simulink model "KUKA_LBR_Simulink_model_flatness_based_control"  (R2017a)
(part 9 of 19)

dblMassInertFullRow6Col4 = (cos(q3)*sin(q1) + cos(q1)*cos(q2)*sin(q3))*(KUKA_LBR_param_.dblLink7InertXZ*(cos(q5)*sin(q2)*sin(q3) + (cos(q3)*cos(q4)*sin(q2) - cos(q2)*sin(q4))*sin(q5)) + KUKA_LBR_param_.dblLink7InertXX*(-(cos(q5)*(cos(q3)*sin(q1) + cos(q1)*cos(q2)*sin(q3))) + (cos(q4)*sin(q1)*sin(q3) - cos(q1)*(cos(q2)*cos(q3)*cos(q4) + sin(q2)*sin(q4)))*sin(q5)) + KUKA_LBR_param_.dblLink7InertXY*(cos(q1)*(cos(q3)*cos(q5) - cos(q4)*sin(q3)*sin(q5)) - sin(q1)*(sin(q2)*sin(q4)*sin(q5) + cos(q2)*(cos(q5)*sin(q3) + cos(q3)*cos(q4)*sin(q5))))) + (-(cos(q1)*cos(q3)) + cos(q2)*sin(q1)*sin(q3))*(KUKA_LBR_param_.dblLink7InertYZ*(cos(q5)*sin(q2)*sin(q3) + (cos(q3)*cos(q4)*sin(q2) - cos(q2)*sin(q4))*sin(q5)) + KUKA_LBR_param_.dblLink7InertXY*(-(cos(q5)*(cos(q3)*sin(q1) + cos(q1)*cos(q2)*sin(q3))) + (cos(q4)*sin(q1)*sin(q3) - cos(q1)*(cos(q2)*cos(q3)*cos(q4) + sin(q2)*sin(q4)))*sin(q5)) + KUKA_LBR_param_.dblLink7InertYY*(cos(q1)*(cos(q3)*cos(q5) - cos(q4)*sin(q3)*sin(q5)) - sin(q1)*(sin(q2)*sin(q4)*sin(q5) + cos(q2)*(cos(q5)*sin(q3) + cos(q3)*cos(q4)*sin(q5))))) - sin(q2)*sin(q3)*(KUKA_LBR_param_.dblLink7InertZZ*(cos(q5)*sin(q2)*sin(q3) + (cos(q3)*cos(q4)*sin(q2) - cos(q2)*sin(q4))*sin(q5)) + KUKA_LBR_param_.dblLink7InertXZ*(-(cos(q5)*(cos(q3)*sin(q1) + cos(q1)*cos(q2)*sin(q3))) + (cos(q4)*sin(q1)*sin(q3) - cos(q1)*(cos(q2)*cos(q3)*cos(q4) + sin(q2)*sin(q4)))*sin(q5)) + KUKA_LBR_param_.dblLink7InertYZ*(cos(q1)*(cos(q3)*cos(q5) - cos(q4)*sin(q3)*sin(q5)) - sin(q1)*(sin(q2)*sin(q4)*sin(q5) + cos(q2)*(cos(q5)*sin(q3) + cos(q3)*cos(q4)*sin(q5))))) + (cos(q5)*(-12*KUKA_LBR_param_.dblLink6InertXX - 12*KUKA_LBR_param_.dblLink6InertYY - 8*KUKA_LBR_param_.dblLink6InertZZ - 32*power(KUKA_LBR_param_.dblLink6CogX,2)*KUKA_LBR_param_.dblLink6Mass - 32*power(KUKA_LBR_param_.dblLink6CogY,2)*KUKA_LBR_param_.dblLink6Mass + 4*(KUKA_LBR_param_.dblLink6InertXX - KUKA_LBR_param_.dblLink6InertYY)*cos(2*q1) + 8*KUKA_LBR_param_.dblLink6InertYZ*cos(q1 - 2*q2) - 2*KUKA_LBR_param_.dblLink6InertXX*cos(2*(q1 - q2)) + 2*KUKA_LBR_param_.dblLink6InertYY*cos(2*(q1 - q2)) - 4*KUKA_LBR_param_.dblLink6InertXX*cos(2*q2) - 4*KUKA_LBR_param_.dblLink6InertYY*cos(2*q2) + 8*KUKA_LBR_param_.dblLink6InertZZ*cos(2*q2) - 2*KUKA_LBR_param_.dblLink6InertXX*cos(2*(q1 + q2)) + 2*KUKA_LBR_param_.dblLink6InertYY*cos(2*(q1 + q2)) - 8*KUKA_LBR_param_.dblLink6InertYZ*cos(q1 + 2*q2) + 8*KUKA_LBR_param_.dblLink6InertYZ*cos(q1 - q2 - 2*q3) - 4*KUKA_LBR_param_.dblLink6InertXX*cos(2*q1 - q2 - 2*q3) + 4*KUKA_LBR_param_.dblLink6InertYY*cos(2*q1 - q2 - 2*q3) - 8*KUKA_LBR_param_.dblLink6InertYZ*cos(q1 + q2 - 2*q3) - 4*KUKA_LBR_param_.dblLink6InertXX*cos(2*q1 + q2 - 2*q3) + 4*KUKA_LBR_param_.dblLink6InertYY*cos(2*q1 + q2 - 2*q3) + 4*KUKA_LBR_param_.dblLink6InertYZ*cos(q1 + 2*q2 - 2*q3) + 6*KUKA_LBR_param_.dblLink6InertXX*cos(2*(q1 - q3)) - 6*KUKA_LBR_param_.dblLink6InertYY*cos(2*(q1 - q3)) + KUKA_LBR_param_.dblLink6InertXX*cos(2*(q1 - q2 - q3)) - KUKA_LBR_param_.dblLink6InertYY*cos(2*(q1 - q2 - q3)) + 2*KUKA_LBR_param_.dblLink6InertXX*cos(2*(q2 - q3)) + 2*KUKA_LBR_param_.dblLink6InertYY*cos(2*(q2 - q3)) - 4*KUKA_LBR_param_.dblLink6InertZZ*cos(2*(q2 - q3)) + KUKA_LBR_param_.dblLink6InertXX*cos(2*(q1 + q2 - q3)) - KUKA_LBR_param_.dblLink6InertYY*cos(2*(q1 + q2 - q3)) - 4*KUKA_LBR_param_.dblLink6InertXX*cos(2*q3) - 4*KUKA_LBR_param_.dblLink6InertYY*cos(2*q3) + 8*KUKA_LBR_param_.dblLink6InertZZ*cos(2*q3) + 6*KUKA_LBR_param_.dblLink6InertXX*cos(2*(q1 + q3)) - 6*KUKA_LBR_param_.dblLink6InertYY*cos(2*(q1 + q3)) + KUKA_LBR_param_.dblLink6InertXX*cos(2*(q1 - q2 + q3)) - KUKA_LBR_param_.dblLink6InertYY*cos(2*(q1 - q2 + q3)) + 2*KUKA_LBR_param_.dblLink6InertXX*cos(2*(q2 + q3)) + 2*KUKA_LBR_param_.dblLink6InertYY*cos(2*(q2 + q3)) - 4*KUKA_LBR_param_.dblLink6InertZZ*cos(2*(q2 + q3)) + KUKA_LBR_param_.dblLink6InertXX*cos(2*(q1 + q2 + q3)) - KUKA_LBR_param_.dblLink6InertYY*cos(2*(q1 + q2 + q3)) - 4*KUKA_LBR_param_.dblLink6InertYZ*cos(q1 - 2*q2 + 2*q3) - 8*KUKA_LBR_param_.dblLink6InertYZ*cos(q1 - q2 + 2*q3) + 4*KUKA_LBR_param_.dblLink6InertXX*cos(2*q1 - q2 + 2*q3) - 4*KUKA_LBR_param_.dblLink6InertYY*cos(2*q1 - q2 + 2*q3) + 8*KUKA_LBR_param_.dblLink6InertYZ*cos(q1 + q2 + 2*q3) + 4*KUKA_LBR_param_.dblLink6InertXX*cos(2*q1 + q2 + 2*q3) - 4*KUKA_LBR_param_.dblLink6InertYY*cos(2*q1 + q2 + 2*q3) - 4*KUKA_LBR_param_.dblLink6InertYZ*cos(q1 - 2*(q2 + q3)) + 4*KUKA_LBR_param_.dblLink6InertYZ*cos(q1 + 2*(q2 + q3)) - 32*KUKA_LBR_param_.dblLink45Len*KUKA_LBR_param_.dblLink6CogY*KUKA_LBR_param_.dblLink6Mass*cos(q6) + 8*KUKA_LBR_param_.dblLink6InertXY*sin(2*q1) - 8*KUKA_LBR_param_.dblLink6InertXZ*sin(q1 - 2*q2) - 4*KUKA_LBR_param_.dblLink6InertXY*sin(2*(q1 - q2)) - 4*KUKA_LBR_param_.dblLink6InertXY*sin(2*(q1 + q2)) + 8*KUKA_LBR_param_.dblLink6InertXZ*sin(q1 + 2*q2) - 8*KUKA_LBR_param_.dblLink6InertXZ*sin(q1 - q2 - 2*q3) - 8*KUKA_LBR_param_.dblLink6InertXY*sin(2*q1 - q2 - 2*q3) + 8*KUKA_LBR_param_.dblLink6InertXZ*sin(q1 + q2 - 2*q3) - 8*KUKA_LBR_param_.dblLink6InertXY*sin(2*q1 + q2 - 2*q3) - 4*KUKA_LBR_param_.dblLink6InertXZ*sin(q1 + 2*q2 - 2*q3) + 12*KUKA_LBR_param_.dblLink6InertXY*sin(2*(q1 - q3)) + 2*KUKA_LBR_param_.dblLink6InertXY*sin(2*(q1 - q2 - q3)) + 2*KUKA_LBR_param_.dblLink6InertXY*sin(2*(q1 + q2 - q3)) + 12*KUKA_LBR_param_.dblLink6InertXY*sin(2*(q1 + q3)) + 2*KUKA_LBR_param_.dblLink6InertXY*sin(2*(q1 - q2 + q3)) + 2*KUKA_LBR_param_.dblLink6InertXY*sin(2*(q1 + q2 + q3)) + 4*KUKA_LBR_param_.dblLink6InertXZ*sin(q1 - 2*q2 + 2*q3) + 8*KUKA_LBR_param_.dblLink6InertXZ*sin(q1 - q2 + 2*q3) + 8*KUKA_LBR_param_.dblLink6InertXY*sin(2*q1 - q2 + 2*q3) - 8*KUKA_LBR_param_.dblLink6InertXZ*sin(q1 + q2 + 2*q3) + 8*KUKA_LBR_param_.dblLink6InertXY*sin(2*q1 + q2 + 2*q3) + 4*KUKA_LBR_param_.dblLink6InertXZ*sin(q1 - 2*(q2 + q3)) - 4*KUKA_LBR_param_.dblLink6InertXZ*sin(q1 + 2*(q2 + q3)) - 32*KUKA_LBR_param_.dblLink45Len*KUKA_LBR_param_.dblLink6CogX*KUKA_LBR_param_.dblLink6Mass*sin(q6)) + 4*sin(q5)*(-8*KUKA_LBR_param_.dblLink6CogX*KUKA_LBR_param_.dblLink6CogZ*KUKA_LBR_param_.dblLink6Mass*cos(q6) + 8*KUKA_LBR_param_.dblLink6InertXZ*power(cos(q3),2)*cos(q4)*sin(q1)*sin(q2) - 8*KUKA_LBR_param_.dblLink6InertXZ*cos(q4)*sin(q1)*sin(q2)*power(sin(q3),2) + KUKA_LBR_param_.dblLink6InertXX*cos(q4)*sin(2*q3) + KUKA_LBR_param_.dblLink6InertYY*cos(q4)*sin(2*q3) - 2*KUKA_LBR_param_.dblLink6InertZZ*cos(q4)*sin(2*q3) + 3*KUKA_LBR_param_.dblLink6InertXX*cos(q4)*power(sin(q1),2)*sin(2*q3) - 3*KUKA_LBR_param_.dblLink6InertYY*cos(q4)*power(sin(q1),2)*sin(2*q3) - 6*KUKA_LBR_param_.dblLink6InertXY*cos(q4)*sin(2*q1)*sin(2*q3) + KUKA_LBR_param_.dblLink6InertXX*cos(q4)*power(sin(q2),2)*sin(2*q3) + KUKA_LBR_param_.dblLink6InertYY*cos(q4)*power(sin(q2),2)*sin(2*q3) - 2*KUKA_LBR_param_.dblLink6InertZZ*cos(q4)*power(sin(q2),2)*sin(2*q3) - KUKA_LBR_param_.dblLink6InertXX*cos(q4)*power(sin(q1),2)*power(sin(q2),2)*sin(2*q3) + KUKA_LBR_param_.dblLink6InertYY*cos(q4)*power(sin(q1),2)*power(sin(q2),2)*sin(2*q3) + 2*KUKA_LBR_param_.dblLink6InertXY*cos(q4)*sin(2*q1)*power(sin(q2),2)*sin(2*q3) + 4*KUKA_LBR_param_.dblLink6InertYZ*cos(q4)*sin(q1)*sin(2*q2)*sin(2*q3) - 8*KUKA_LBR_param_.dblLink6InertXY*cos(q3)*power(sin(q1),2)*sin(q2)*sin(q4) - 4*KUKA_LBR_param_.dblLink6InertXX*cos(q3)*sin(2*q1)*sin(q2)*sin(q4) + 4*KUKA_LBR_param_.dblLink6InertYY*cos(q3)*sin(2*q1)*sin(q2)*sin(q4) - 4*KUKA_LBR_param_.dblLink6InertXX*cos(q2)*sin(q2)*sin(q3)*sin(q4) + 4*KUKA_LBR_param_.dblLink6InertXX*cos(q2)*power(sin(q1),2)*sin(q2)*sin(q3)*sin(q4) + 8*KUKA_LBR_param_.dblLink6InertYZ*sin(q1)*power(sin(q2),2)*sin(q3)*sin(q4) - 2*KUKA_LBR_param_.dblLink6InertYY*sin(2*q2)*sin(q3)*sin(q4) + 4*KUKA_LBR_param_.dblLink6InertZZ*sin(2*q2)*sin(q3)*sin(q4) - 2*KUKA_LBR_param_.dblLink6InertYY*power(sin(q1),2)*sin(2*q2)*sin(q3)*sin(q4) - 4*KUKA_LBR_param_.dblLink6InertXY*sin(2*q1)*sin(2*q2)*sin(q3)*sin(q4) - 4*cos(q2)*(2*KUKA_LBR_param_.dblLink6InertXY*power(cos(q3),2)*cos(q4)*power(sin(q1),2) + cos(q4)*((KUKA_LBR_param_.dblLink6InertXX - KUKA_LBR_param_.dblLink6InertYY)*cos(2*q3)*sin(2*q1) - 2*KUKA_LBR_param_.dblLink6InertXY*power(sin(q1),2)*power(sin(q3),2)) + 2*KUKA_LBR_param_.dblLink6InertXZ*cos(q3)*sin(q1)*sin(q4)) - (power(cos(q2),2)*(cos(q4)*(KUKA_LBR_param_.dblLink6InertXX + 3*KUKA_LBR_param_.dblLink6InertYY - 4*KUKA_LBR_param_.dblLink6InertZZ + (KUKA_LBR_param_.dblLink6InertXX - KUKA_LBR_param_.dblLink6InertYY)*cos(2*q1) + 4*KUKA_LBR_param_.dblLink6InertXY*sin(2*q1))*sin(2*q3) + 16*KUKA_LBR_param_.dblLink6InertYZ*sin(q1)*sin(q3)*sin(q4)))/2.0 - 8*cos(q1)*(KUKA_LBR_param_.dblLink6InertYZ*power(cos(q3),2)*cos(q4)*sin(q2) - cos(q2)*cos(q3)*(2*KUKA_LBR_param_.dblLink6InertXZ*cos(q4)*sin(q2)*sin(q3) + KUKA_LBR_param_.dblLink6InertYZ*sin(q4)) + sin(q3)*(-(KUKA_LBR_param_.dblLink6InertYZ*cos(q4)*sin(q2)*sin(q3)) + KUKA_LBR_param_.dblLink6InertXZ*cos(2*q2)*sin(q4))) + 2*power(cos(q1),2)*(-((KUKA_LBR_param_.dblLink6InertXX - KUKA_LBR_param_.dblLink6InertYY)*power(cos(q2),2)*cos(q3)*cos(q4)*sin(q3)) + KUKA_LBR_param_.dblLink6InertYY*sin(2*q2)*sin(q3)*sin(q4) + cos(q3)*(-((KUKA_LBR_param_.dblLink6InertXX - KUKA_LBR_param_.dblLink6InertYY)*(5 + cos(2*q2))*cos(q4)*sin(q3))/2.0 + 4*KUKA_LBR_param_.dblLink6InertXY*sin(q2)*sin(q4)) + cos(q2)*(4*KUKA_LBR_param_.dblLink6InertXY*power(cos(q3),2)*cos(q4) - 2*sin(q3)*(2*KUKA_LBR_param_.dblLink6InertXY*cos(q4)*sin(q3) + KUKA_LBR_param_.dblLink6InertXX*sin(q2)*sin(q4)))) + 8*KUKA_LBR_param_.dblLink6CogY*KUKA_LBR_param_.dblLink6CogZ*KUKA_LBR_param_.dblLink6Mass*sin(q6)))/32.0 - KUKA_LBR_param_.dblLink7Mass*(cos(q4)*(-(sin(q1)*sin(q2)*sin(q5)*(KUKA_LBR_param_.dblLink7CogY*cos(q7) + KUKA_LBR_param_.dblLink7CogX*sin(q7))) + cos(q1)*sin(q3)*(KUKA_LBR_param_.dblLink45Len + KUKA_LBR_param_.dblLink7CogZ*cos(q6) + KUKA_LBR_param_.dblLink7CogX*cos(q7)*sin(q6) - KUKA_LBR_param_.dblLink7CogY*sin(q6)*sin(q7)) - cos(q5)*sin(q1)*sin(q2)*(KUKA_LBR_param_.dblLink7CogZ*sin(q6) + cos(q6)*(-(KUKA_LBR_param_.dblLink7CogX*cos(q7)) + KUKA_LBR_param_.dblLink7CogY*sin(q7)))) + sin(q4)*(sin(q1)*sin(q2)*(KUKA_LBR_param_.dblLink45Len + KUKA_LBR_param_.dblLink7CogZ*cos(q6) + KUKA_LBR_param_.dblLink7CogX*cos(q7)*sin(q6) - KUKA_LBR_param_.dblLink7CogY*sin(q6)*sin(q7)) + cos(q1)*sin(q3)*(sin(q5)*(KUKA_LBR_param_.dblLink7CogY*cos(q7) + KUKA_LBR_param_.dblLink7CogX*sin(q7)) + cos(q5)*(-(KUKA_LBR_param_.dblLink7CogX*cos(q6)*cos(q7)) + KUKA_LBR_param_.dblLink7CogZ*sin(q6) + KUKA_LBR_param_.dblLink7CogY*cos(q6)*sin(q7)))) + cos(q2)*cos(q3)*sin(q1)*(cos(q4)*(KUKA_LBR_param_.dblLink45Len + KUKA_LBR_param_.dblLink7CogZ*cos(q6) + KUKA_LBR_param_.dblLink7CogX*cos(q7)*sin(q6) - KUKA_LBR_param_.dblLink7CogY*sin(q6)*sin(q7)) + sin(q4)*(sin(q5)*(KUKA_LBR_param_.dblLink7CogY*cos(q7) + KUKA_LBR_param_.dblLink7CogX*sin(q7)) + cos(q5)*(-(KUKA_LBR_param_.dblLink7CogX*cos(q6)*cos(q7)) + KUKA_LBR_param_.dblLink7CogZ*sin(q6) + KUKA_LBR_param_.dblLink7CogY*cos(q6)*sin(q7)))))*(KUKA_LBR_param_.dblLink7CogZ*cos(q5)*cos(q6)*sin(q1)*sin(q2)*sin(q4) - KUKA_LBR_param_.dblLink7CogX*cos(q1)*cos(q6)*cos(q7)*sin(q3)*sin(q4) + KUKA_LBR_param_.dblLink7CogZ*cos(q1)*cos(q3)*cos(q6)*sin(q5) + KUKA_LBR_param_.dblLink7CogX*cos(q5)*cos(q7)*sin(q1)*sin(q2)*sin(q4)*sin(q6) + KUKA_LBR_param_.dblLink7CogZ*cos(q1)*sin(q3)*sin(q4)*sin(q6) + KUKA_LBR_param_.dblLink7CogX*cos(q1)*cos(q3)*cos(q7)*sin(q5)*sin(q6) + KUKA_LBR_param_.dblLink7CogY*cos(q1)*cos(q6)*sin(q3)*sin(q4)*sin(q7) - KUKA_LBR_param_.dblLink7CogY*cos(q5)*sin(q1)*sin(q2)*sin(q4)*sin(q6)*sin(q7) - KUKA_LBR_param_.dblLink7CogY*cos(q1)*cos(q3)*sin(q5)*sin(q6)*sin(q7) + cos(q4)*(cos(q6)*(KUKA_LBR_param_.dblLink7CogX*cos(q7)*sin(q1)*sin(q2) + KUKA_LBR_param_.dblLink7CogZ*cos(q1)*cos(q5)*sin(q3) - KUKA_LBR_param_.dblLink7CogY*sin(q1)*sin(q2)*sin(q7)) - sin(q6)*(KUKA_LBR_param_.dblLink7CogZ*sin(q1)*sin(q2) + cos(q1)*cos(q5)*sin(q3)*(-(KUKA_LBR_param_.dblLink7CogX*cos(q7)) + KUKA_LBR_param_.dblLink7CogY*sin(q7)))) + cos(q2)*sin(q1)*(-(sin(q3)*sin(q5)*(KUKA_LBR_param_.dblLink7CogZ*cos(q6) + sin(q6)*(KUKA_LBR_param_.dblLink7CogX*cos(q7) - KUKA_LBR_param_.dblLink7CogY*sin(q7)))) + cos(q3)*(sin(q4)*(-(KUKA_LBR_param_.dblLink7CogX*cos(q6)*cos(q7)) + KUKA_LBR_param_.dblLink7CogZ*sin(q6) + KUKA_LBR_param_.dblLink7CogY*cos(q6)*sin(q7)) + cos(q4)*cos(q5)*(KUKA_LBR_param_.dblLink7CogZ*cos(q6) + KUKA_LBR_param_.dblLink7CogX*cos(q7)*sin(q6) - KUKA_LBR_param_.dblLink7CogY*sin(q6)*sin(q7))))) + KUKA_LBR_param_.dblLink7Mass*(cos(q2)*(-(sin(q4)*(KUKA_LBR_param_.dblLink45Len + KUKA_LBR_param_.dblLink7CogZ*cos(q6) + KUKA_LBR_param_.dblLink7CogX*cos(q7)*sin(q6) - KUKA_LBR_param_.dblLink7CogY*sin(q6)*sin(q7))) + cos(q4)*(sin(q5)*(KUKA_LBR_param_.dblLink7CogY*cos(q7) + KUKA_LBR_param_.dblLink7CogX*sin(q7)) + cos(q5)*(-(KUKA_LBR_param_.dblLink7CogX*cos(q6)*cos(q7)) + KUKA_LBR_param_.dblLink7CogZ*sin(q6) + KUKA_LBR_param_.dblLink7CogY*cos(q6)*sin(q7)))) + cos(q3)*sin(q2)*(cos(q4)*(KUKA_LBR_param_.dblLink45Len + KUKA_LBR_param_.dblLink7CogZ*cos(q6) + KUKA_LBR_param_.dblLink7CogX*cos(q7)*sin(q6) - KUKA_LBR_param_.dblLink7CogY*sin(q6)*sin(q7)) + sin(q4)*(sin(q5)*(KUKA_LBR_param_.dblLink7CogY*cos(q7) + KUKA_LBR_param_.dblLink7CogX*sin(q7)) + cos(q5)*(-(KUKA_LBR_param_.dblLink7CogX*cos(q6)*cos(q7)) + KUKA_LBR_param_.dblLink7CogZ*sin(q6) + KUKA_LBR_param_.dblLink7CogY*cos(q6)*sin(q7)))))*(cos(q2)*(cos(q4)*(KUKA_LBR_param_.dblLink7CogX*cos(q6)*cos(q7) - KUKA_LBR_param_.dblLink7CogZ*sin(q6) - KUKA_LBR_param_.dblLink7CogY*cos(q6)*sin(q7)) + cos(q5)*sin(q4)*(KUKA_LBR_param_.dblLink7CogZ*cos(q6) + KUKA_LBR_param_.dblLink7CogX*cos(q7)*sin(q6) - KUKA_LBR_param_.dblLink7CogY*sin(q6)*sin(q7))) - sin(q2)*(-(sin(q3)*sin(q5)*(KUKA_LBR_param_.dblLink7CogZ*cos(q6) + sin(q6)*(KUKA_LBR_param_.dblLink7CogX*cos(q7) - KUKA_LBR_param_.dblLink7CogY*sin(q7)))) + cos(q3)*(sin(q4)*(-(KUKA_LBR_param_.dblLink7CogX*cos(q6)*cos(q7)) + KUKA_LBR_param_.dblLink7CogZ*sin(q6) + KUKA_LBR_param_.dblLink7CogY*cos(q6)*sin(q7)) + cos(q4)*cos(q5)*(KUKA_LBR_param_.dblLink7CogZ*cos(q6) + KUKA_LBR_param_.dblLink7CogX*cos(q7)*sin(q6) - KUKA_LBR_param_.dblLink7CogY*sin(q6)*sin(q7))))) + KUKA_LBR_param_.dblLink7Mass*(sin(q1)*sin(q3)*(cos(q4)*(KUKA_LBR_param_.dblLink45Len + KUKA_LBR_param_.dblLink7CogZ*cos(q6) + KUKA_LBR_param_.dblLink7CogX*cos(q7)*sin(q6) - KUKA_LBR_param_.dblLink7CogY*sin(q6)*sin(q7)) + sin(q4)*(sin(q5)*(KUKA_LBR_param_.dblLink7CogY*cos(q7) + KUKA_LBR_param_.dblLink7CogX*sin(q7)) + cos(q5)*(-(KUKA_LBR_param_.dblLink7CogX*cos(q6)*cos(q7)) + KUKA_LBR_param_.dblLink7CogZ*sin(q6) + KUKA_LBR_param_.dblLink7CogY*cos(q6)*sin(q7)))) - cos(q1)*(sin(q2)*(sin(q4)*(KUKA_LBR_param_.dblLink45Len + KUKA_LBR_param_.dblLink7CogZ*cos(q6) + KUKA_LBR_param_.dblLink7CogX*cos(q7)*sin(q6) - KUKA_LBR_param_.dblLink7CogY*sin(q6)*sin(q7)) - cos(q4)*(sin(q5)*(KUKA_LBR_param_.dblLink7CogY*cos(q7) + KUKA_LBR_param_.dblLink7CogX*sin(q7)) + cos(q5)*(-(KUKA_LBR_param_.dblLink7CogX*cos(q6)*cos(q7)) + KUKA_LBR_param_.dblLink7CogZ*sin(q6) + KUKA_LBR_param_.dblLink7CogY*cos(q6)*sin(q7)))) + cos(q2)*cos(q3)*(cos(q4)*(KUKA_LBR_param_.dblLink45Len + KUKA_LBR_param_.dblLink7CogZ*cos(q6) + KUKA_LBR_param_.dblLink7CogX*cos(q7)*sin(q6) - KUKA_LBR_param_.dblLink7CogY*sin(q6)*sin(q7)) + sin(q4)*(sin(q5)*(KUKA_LBR_param_.dblLink7CogY*cos(q7) + KUKA_LBR_param_.dblLink7CogX*sin(q7)) + cos(q5)*(-(KUKA_LBR_param_.dblLink7CogX*cos(q6)*cos(q7)) + KUKA_LBR_param_.dblLink7CogZ*sin(q6) + KUKA_LBR_param_.dblLink7CogY*cos(q6)*sin(q7))))))*(-(sin(q1)*(cos(q6)*(-(KUKA_LBR_param_.dblLink7CogX*cos(q7)*sin(q3)*sin(q4)) + KUKA_LBR_param_.dblLink7CogZ*cos(q3)*sin(q5) + KUKA_LBR_param_.dblLink7CogY*sin(q3)*sin(q4)*sin(q7)) + sin(q6)*(KUKA_LBR_param_.dblLink7CogZ*sin(q3)*sin(q4) + cos(q3)*sin(q5)*(KUKA_LBR_param_.dblLink7CogX*cos(q7) - KUKA_LBR_param_.dblLink7CogY*sin(q7))) + cos(q4)*cos(q5)*sin(q3)*(KUKA_LBR_param_.dblLink7CogZ*cos(q6) + sin(q6)*(KUKA_LBR_param_.dblLink7CogX*cos(q7) - KUKA_LBR_param_.dblLink7CogY*sin(q7))))) + cos(q1)*(sin(q2)*(cos(q4)*(KUKA_LBR_param_.dblLink7CogX*cos(q6)*cos(q7) - KUKA_LBR_param_.dblLink7CogZ*sin(q6) - KUKA_LBR_param_.dblLink7CogY*cos(q6)*sin(q7)) + cos(q5)*sin(q4)*(KUKA_LBR_param_.dblLink7CogZ*cos(q6) + KUKA_LBR_param_.dblLink7CogX*cos(q7)*sin(q6) - KUKA_LBR_param_.dblLink7CogY*sin(q6)*sin(q7))) + cos(q2)*(-(sin(q3)*sin(q5)*(KUKA_LBR_param_.dblLink7CogZ*cos(q6) + sin(q6)*(KUKA_LBR_param_.dblLink7CogX*cos(q7) - KUKA_LBR_param_.dblLink7CogY*sin(q7)))) + cos(q3)*(sin(q4)*(-(KUKA_LBR_param_.dblLink7CogX*cos(q6)*cos(q7)) + KUKA_LBR_param_.dblLink7CogZ*sin(q6) + KUKA_LBR_param_.dblLink7CogY*cos(q6)*sin(q7)) + cos(q4)*cos(q5)*(KUKA_LBR_param_.dblLink7CogZ*cos(q6) + KUKA_LBR_param_.dblLink7CogX*cos(q7)*sin(q6) - KUKA_LBR_param_.dblLink7CogY*sin(q6)*sin(q7))))));
dblMassInertFullRow6Col5 = (sin(q1)*sin(q3)*sin(q4) + cos(q1)*(cos(q4)*sin(q2) - cos(q2)*cos(q3)*sin(q4)))*(KUKA_LBR_param_.dblLink7InertXZ*(cos(q5)*sin(q2)*sin(q3) + (cos(q3)*cos(q4)*sin(q2) - cos(q2)*sin(q4))*sin(q5)) + KUKA_LBR_param_.dblLink7InertXX*(-(cos(q5)*(cos(q3)*sin(q1) + cos(q1)*cos(q2)*sin(q3))) + (cos(q4)*sin(q1)*sin(q3) - cos(q1)*(cos(q2)*cos(q3)*cos(q4) + sin(q2)*sin(q4)))*sin(q5)) + KUKA_LBR_param_.dblLink7InertXY*(cos(q1)*(cos(q3)*cos(q5) - cos(q4)*sin(q3)*sin(q5)) - sin(q1)*(sin(q2)*sin(q4)*sin(q5) + cos(q2)*(cos(q5)*sin(q3) + cos(q3)*cos(q4)*sin(q5))))) + (cos(q4)*sin(q1)*sin(q2) - (cos(q2)*cos(q3)*sin(q1) + cos(q1)*sin(q3))*sin(q4))*(KUKA_LBR_param_.dblLink7InertYZ*(cos(q5)*sin(q2)*sin(q3) + (cos(q3)*cos(q4)*sin(q2) - cos(q2)*sin(q4))*sin(q5)) + KUKA_LBR_param_.dblLink7InertXY*(-(cos(q5)*(cos(q3)*sin(q1) + cos(q1)*cos(q2)*sin(q3))) + (cos(q4)*sin(q1)*sin(q3) - cos(q1)*(cos(q2)*cos(q3)*cos(q4) + sin(q2)*sin(q4)))*sin(q5)) + KUKA_LBR_param_.dblLink7InertYY*(cos(q1)*(cos(q3)*cos(q5) - cos(q4)*sin(q3)*sin(q5)) - sin(q1)*(sin(q2)*sin(q4)*sin(q5) + cos(q2)*(cos(q5)*sin(q3) + cos(q3)*cos(q4)*sin(q5))))) + (cos(q2)*cos(q4) + cos(q3)*sin(q2)*sin(q4))*(KUKA_LBR_param_.dblLink7InertZZ*(cos(q5)*sin(q2)*sin(q3) + (cos(q3)*cos(q4)*sin(q2) - cos(q2)*sin(q4))*sin(q5)) + KUKA_LBR_param_.dblLink7InertXZ*(-(cos(q5)*(cos(q3)*sin(q1) + cos(q1)*cos(q2)*sin(q3))) + (cos(q4)*sin(q1)*sin(q3) - cos(q1)*(cos(q2)*cos(q3)*cos(q4) + sin(q2)*sin(q4)))*sin(q5)) + KUKA_LBR_param_.dblLink7InertYZ*(cos(q1)*(cos(q3)*cos(q5) - cos(q4)*sin(q3)*sin(q5)) - sin(q1)*(sin(q2)*sin(q4)*sin(q5) + cos(q2)*(cos(q5)*sin(q3) + cos(q3)*cos(q4)*sin(q5))))) + (power(cos(q1),2)*(32*KUKA_LBR_param_.dblLink6InertXY*cos(q2)*cos(q5)*power(sin(q3),2)*sin(q4) + 10*KUKA_LBR_param_.dblLink6InertXX*cos(q5)*sin(2*q3)*sin(q4) - 14*KUKA_LBR_param_.dblLink6InertYY*cos(q5)*sin(2*q3)*sin(q4) + 4*KUKA_LBR_param_.dblLink6InertXX*power(cos(q2),2)*cos(q5)*sin(2*q3)*sin(q4) + 2*KUKA_LBR_param_.dblLink6InertXX*cos(2*q2)*cos(q5)*sin(2*q3)*sin(q4) - 2*KUKA_LBR_param_.dblLink6InertYY*cos(2*q2)*cos(q5)*sin(2*q3)*sin(q4) + 4*KUKA_LBR_param_.dblLink6InertYY*cos(q5)*power(sin(q2),2)*sin(2*q3)*sin(q4) - 32*KUKA_LBR_param_.dblLink6InertXY*power(cos(q4),2)*sin(q2)*sin(q3)*sin(q5) + 32*KUKA_LBR_param_.dblLink6InertXY*sin(q2)*sin(q3)*power(sin(q4),2)*sin(q5) - 6*KUKA_LBR_param_.dblLink6InertXX*sin(2*q4)*sin(q5) + 6*KUKA_LBR_param_.dblLink6InertYY*sin(2*q4)*sin(q5) + 5*KUKA_LBR_param_.dblLink6InertXX*power(cos(q2),2)*sin(2*q4)*sin(q5) - 5*KUKA_LBR_param_.dblLink6InertYY*power(cos(q2),2)*sin(2*q4)*sin(q5) + KUKA_LBR_param_.dblLink6InertXX*power(cos(q2),2)*cos(2*q3)*sin(2*q4)*sin(q5) - KUKA_LBR_param_.dblLink6InertYY*power(cos(q2),2)*cos(2*q3)*sin(2*q4)*sin(q5) - 6*KUKA_LBR_param_.dblLink6InertXX*power(sin(q2),2)*sin(2*q4)*sin(q5) + 6*KUKA_LBR_param_.dblLink6InertYY*power(sin(q2),2)*sin(2*q4)*sin(q5) - 6*KUKA_LBR_param_.dblLink6InertXX*power(sin(q3),2)*sin(2*q4)*sin(q5) + 6*KUKA_LBR_param_.dblLink6InertYY*power(sin(q3),2)*sin(2*q4)*sin(q5) - 2*KUKA_LBR_param_.dblLink6InertYY*power(sin(q2),2)*power(sin(q3),2)*sin(2*q4)*sin(q5) + 16*KUKA_LBR_param_.dblLink6InertXY*cos(q2)*sin(2*q3)*sin(2*q4)*sin(q5) - 2*power(cos(q3),2)*sin(q4)*(16*KUKA_LBR_param_.dblLink6InertXY*cos(q2)*cos(q5) - 2*(KUKA_LBR_param_.dblLink6InertXX - KUKA_LBR_param_.dblLink6InertYY)*power(cos(q2),2)*cos(q4)*sin(q5) - (KUKA_LBR_param_.dblLink6InertXX - KUKA_LBR_param_.dblLink6InertYY)*(5 + cos(2*q2))*cos(q4)*sin(q5)) + 4*cos(q4)*sin(q3)*(-2*(KUKA_LBR_param_.dblLink6InertXX - KUKA_LBR_param_.dblLink6InertYY)*cos(q5)*sin(2*q2) + KUKA_LBR_param_.dblLink6InertXX*power(sin(q2),2)*sin(q3)*sin(q4)*sin(q5)) + 8*cos(q3)*(4*KUKA_LBR_param_.dblLink6InertXY*cos(q4)*cos(q5)*sin(q2) - (KUKA_LBR_param_.dblLink6InertXX - KUKA_LBR_param_.dblLink6InertYY)*power(cos(q4),2)*sin(2*q2)*sin(q5) + (KUKA_LBR_param_.dblLink6InertXX - KUKA_LBR_param_.dblLink6InertYY)*sin(2*q2)*power(sin(q4),2)*sin(q5))) + 8*cos(q1)*(4*KUKA_LBR_param_.dblLink6InertXZ*cos(q4)*cos(q5)*power(sin(q2),2)*sin(q3) + 4*KUKA_LBR_param_.dblLink6InertYZ*power(cos(q3),2)*cos(q5)*sin(q2)*sin(q4) - 4*KUKA_LBR_param_.dblLink6InertYZ*cos(q5)*sin(q2)*power(sin(q3),2)*sin(q4) - 2*KUKA_LBR_param_.dblLink6InertXZ*cos(q5)*sin(2*q2)*sin(2*q3)*sin(q4) + 4*KUKA_LBR_param_.dblLink6InertXX*power(cos(q4),2)*sin(q1)*sin(q2)*sin(q3)*sin(q5) - 4*KUKA_LBR_param_.dblLink6InertYY*power(cos(q4),2)*sin(q1)*sin(q2)*sin(q3)*sin(q5) - 4*KUKA_LBR_param_.dblLink6InertXX*sin(q1)*sin(q2)*sin(q3)*power(sin(q4),2)*sin(q5) + 4*KUKA_LBR_param_.dblLink6InertYY*sin(q1)*sin(q2)*sin(q3)*power(sin(q4),2)*sin(q5) - 3*KUKA_LBR_param_.dblLink6InertXZ*sin(2*q2)*sin(2*q4)*sin(q5) + KUKA_LBR_param_.dblLink6InertXZ*sin(2*q2)*power(sin(q3),2)*sin(2*q4)*sin(q5) - 2*KUKA_LBR_param_.dblLink6InertYZ*sin(q2)*sin(2*q3)*sin(2*q4)*sin(q5) - 4*KUKA_LBR_param_.dblLink6InertXZ*power(cos(q2),2)*(cos(q4)*cos(q5)*sin(q3) + cos(q3)*power(cos(q4),2)*sin(q5) - cos(q3)*power(sin(q4),2)*sin(q5)) + 4*cos(q3)*sin(q2)*(-((KUKA_LBR_param_.dblLink6InertXX - KUKA_LBR_param_.dblLink6InertYY)*cos(q4)*cos(q5)*sin(q1)) + KUKA_LBR_param_.dblLink6InertXZ*power(cos(q4),2)*sin(q2)*sin(q5) - KUKA_LBR_param_.dblLink6InertXZ*sin(q2)*power(sin(q4),2)*sin(q5)) + 4*cos(q2)*(KUKA_LBR_param_.dblLink6InertYZ*cos(q3)*cos(q4)*cos(q5) - sin(q3)*((KUKA_LBR_param_.dblLink6InertXX - KUKA_LBR_param_.dblLink6InertYY)*cos(q5)*sin(q1)*sin(q3)*sin(q4) + KUKA_LBR_param_.dblLink6InertYZ*cos(2*q4)*sin(q5)) + power(cos(q3),2)*sin(q4)*((KUKA_LBR_param_.dblLink6InertXX - KUKA_LBR_param_.dblLink6InertYY)*cos(q5)*sin(q1) - KUKA_LBR_param_.dblLink6InertXZ*cos(q4)*sin(q2)*sin(q5)))) - 2*(16*KUKA_LBR_param_.dblLink6CogY*KUKA_LBR_param_.dblLink6CogZ*KUKA_LBR_param_.dblLink6Mass*cos(q6) + 16*KUKA_LBR_param_.dblLink6InertXY*cos(q3)*cos(q4)*cos(q5)*power(sin(q1),2)*sin(q2) - 16*KUKA_LBR_param_.dblLink6InertYZ*cos(q4)*cos(q5)*sin(q1)*power(sin(q2),2)*sin(q3) + 4*KUKA_LBR_param_.dblLink6InertXX*cos(q4)*cos(q5)*sin(2*q2)*sin(q3) + 4*KUKA_LBR_param_.dblLink6InertYY*cos(q4)*cos(q5)*sin(2*q2)*sin(q3) - 8*KUKA_LBR_param_.dblLink6InertZZ*cos(q4)*cos(q5)*sin(2*q2)*sin(q3) - 4*KUKA_LBR_param_.dblLink6InertXX*cos(q4)*cos(q5)*power(sin(q1),2)*sin(2*q2)*sin(q3) + 4*KUKA_LBR_param_.dblLink6InertYY*cos(q4)*cos(q5)*power(sin(q1),2)*sin(2*q2)*sin(q3) + 8*KUKA_LBR_param_.dblLink6InertXY*cos(q4)*cos(q5)*sin(2*q1)*sin(2*q2)*sin(q3) + 16*KUKA_LBR_param_.dblLink6InertXZ*power(cos(q3),2)*cos(q5)*sin(q1)*sin(q2)*sin(q4) + 4*KUKA_LBR_param_.dblLink6InertXX*cos(q3)*cos(q5)*sin(q3)*sin(q4) + 4*KUKA_LBR_param_.dblLink6InertYY*cos(q3)*cos(q5)*sin(q3)*sin(q4) + 4*KUKA_LBR_param_.dblLink6InertXX*cos(q3)*cos(q5)*power(sin(q2),2)*sin(q3)*sin(q4) + 4*KUKA_LBR_param_.dblLink6InertYY*cos(q3)*cos(q5)*power(sin(q2),2)*sin(q3)*sin(q4) + 4*KUKA_LBR_param_.dblLink6InertYY*cos(q3)*cos(q5)*power(sin(q1),2)*power(sin(q2),2)*sin(q3)*sin(q4) - 16*KUKA_LBR_param_.dblLink6InertXZ*cos(q5)*sin(q1)*sin(q2)*power(sin(q3),2)*sin(q4) - 4*KUKA_LBR_param_.dblLink6InertZZ*cos(q5)*sin(2*q3)*sin(q4) + 6*KUKA_LBR_param_.dblLink6InertXX*cos(q5)*power(sin(q1),2)*sin(2*q3)*sin(q4) - 6*KUKA_LBR_param_.dblLink6InertYY*cos(q5)*power(sin(q1),2)*sin(2*q3)*sin(q4) - 12*KUKA_LBR_param_.dblLink6InertXY*cos(q5)*sin(2*q1)*sin(2*q3)*sin(q4) - 4*KUKA_LBR_param_.dblLink6InertZZ*cos(q5)*power(sin(q2),2)*sin(2*q3)*sin(q4) - 2*KUKA_LBR_param_.dblLink6InertXX*cos(q5)*power(sin(q1),2)*power(sin(q2),2)*sin(2*q3)*sin(q4) + 4*KUKA_LBR_param_.dblLink6InertXY*cos(q5)*sin(2*q1)*power(sin(q2),2)*sin(2*q3)*sin(q4) + 8*KUKA_LBR_param_.dblLink6InertYZ*cos(q5)*sin(q1)*sin(2*q2)*sin(2*q3)*sin(q4) - 16*KUKA_LBR_param_.dblLink6InertYZ*cos(q3)*power(cos(q4),2)*sin(q1)*power(sin(q2),2)*sin(q5) + 4*KUKA_LBR_param_.dblLink6InertXX*cos(q3)*power(cos(q4),2)*sin(2*q2)*sin(q5) + 4*KUKA_LBR_param_.dblLink6InertYY*cos(q3)*power(cos(q4),2)*sin(2*q2)*sin(q5) - 8*KUKA_LBR_param_.dblLink6InertZZ*cos(q3)*power(cos(q4),2)*sin(2*q2)*sin(q5) - 4*KUKA_LBR_param_.dblLink6InertXX*cos(q3)*power(cos(q4),2)*power(sin(q1),2)*sin(2*q2)*sin(q5) + 4*KUKA_LBR_param_.dblLink6InertYY*cos(q3)*power(cos(q4),2)*power(sin(q1),2)*sin(2*q2)*sin(q5) + 8*KUKA_LBR_param_.dblLink6InertXY*cos(q3)*power(cos(q4),2)*sin(2*q1)*sin(2*q2)*sin(q5) - 16*KUKA_LBR_param_.dblLink6InertXY*power(cos(q4),2)*power(sin(q1),2)*sin(q2)*sin(q3)*sin(q5) - 2*KUKA_LBR_param_.dblLink6InertXX*cos(q4)*sin(q4)*sin(q5) - 2*KUKA_LBR_param_.dblLink6InertYY*cos(q4)*sin(q4)*sin(q5) + 4*KUKA_LBR_param_.dblLink6InertZZ*cos(q4)*sin(q4)*sin(q5) - 2*KUKA_LBR_param_.dblLink6InertXX*power(cos(q3),2)*cos(q4)*power(sin(q1),2)*power(sin(q2),2)*sin(q4)*sin(q5) - 2*KUKA_LBR_param_.dblLink6InertXX*cos(q4)*power(sin(q3),2)*sin(q4)*sin(q5) - 2*KUKA_LBR_param_.dblLink6InertYY*cos(q4)*power(sin(q3),2)*sin(q4)*sin(q5) + 4*KUKA_LBR_param_.dblLink6InertZZ*cos(q4)*power(sin(q3),2)*sin(q4)*sin(q5) - 2*KUKA_LBR_param_.dblLink6InertXX*cos(q4)*power(sin(q2),2)*power(sin(q3),2)*sin(q4)*sin(q5) - 2*KUKA_LBR_param_.dblLink6InertYY*cos(q4)*power(sin(q2),2)*power(sin(q3),2)*sin(q4)*sin(q5) + 4*KUKA_LBR_param_.dblLink6InertZZ*cos(q4)*power(sin(q2),2)*power(sin(q3),2)*sin(q4)*sin(q5) - 2*KUKA_LBR_param_.dblLink6InertYY*cos(q4)*power(sin(q1),2)*power(sin(q2),2)*power(sin(q3),2)*sin(q4)*sin(q5) + 16*KUKA_LBR_param_.dblLink6InertYZ*cos(q3)*sin(q1)*power(sin(q2),2)*power(sin(q4),2)*sin(q5) - 4*KUKA_LBR_param_.dblLink6InertXX*cos(q3)*sin(2*q2)*power(sin(q4),2)*sin(q5) - 4*KUKA_LBR_param_.dblLink6InertYY*cos(q3)*sin(2*q2)*power(sin(q4),2)*sin(q5) + 8*KUKA_LBR_param_.dblLink6InertZZ*cos(q3)*sin(2*q2)*power(sin(q4),2)*sin(q5) + 4*KUKA_LBR_param_.dblLink6InertXX*cos(q3)*power(sin(q1),2)*sin(2*q2)*power(sin(q4),2)*sin(q5) - 4*KUKA_LBR_param_.dblLink6InertYY*cos(q3)*power(sin(q1),2)*sin(2*q2)*power(sin(q4),2)*sin(q5) - 8*KUKA_LBR_param_.dblLink6InertXY*cos(q3)*sin(2*q1)*sin(2*q2)*power(sin(q4),2)*sin(q5) + 16*KUKA_LBR_param_.dblLink6InertXY*power(sin(q1),2)*sin(q2)*sin(q3)*power(sin(q4),2)*sin(q5) + KUKA_LBR_param_.dblLink6InertXX*power(cos(q3),2)*sin(2*q4)*sin(q5) + KUKA_LBR_param_.dblLink6InertYY*power(cos(q3),2)*sin(2*q4)*sin(q5) - 2*KUKA_LBR_param_.dblLink6InertZZ*power(cos(q3),2)*sin(2*q4)*sin(q5) - 3*KUKA_LBR_param_.dblLink6InertXX*power(sin(q1),2)*sin(2*q4)*sin(q5) + 3*KUKA_LBR_param_.dblLink6InertYY*power(sin(q1),2)*sin(2*q4)*sin(q5) + 3*KUKA_LBR_param_.dblLink6InertXX*power(cos(q3),2)*power(sin(q1),2)*sin(2*q4)*sin(q5) - 3*KUKA_LBR_param_.dblLink6InertYY*power(cos(q3),2)*power(sin(q1),2)*sin(2*q4)*sin(q5) + 6*KUKA_LBR_param_.dblLink6InertXY*sin(2*q1)*sin(2*q4)*sin(q5) - 6*KUKA_LBR_param_.dblLink6InertXY*power(cos(q3),2)*sin(2*q1)*sin(2*q4)*sin(q5) + 3*KUKA_LBR_param_.dblLink6InertXX*power(sin(q2),2)*sin(2*q4)*sin(q5) + 3*KUKA_LBR_param_.dblLink6InertYY*power(sin(q2),2)*sin(2*q4)*sin(q5) - 6*KUKA_LBR_param_.dblLink6InertZZ*power(sin(q2),2)*sin(2*q4)*sin(q5) + KUKA_LBR_param_.dblLink6InertXX*power(cos(q3),2)*power(sin(q2),2)*sin(2*q4)*sin(q5) + KUKA_LBR_param_.dblLink6InertYY*power(cos(q3),2)*power(sin(q2),2)*sin(2*q4)*sin(q5) - 2*KUKA_LBR_param_.dblLink6InertZZ*power(cos(q3),2)*power(sin(q2),2)*sin(2*q4)*sin(q5) - 3*KUKA_LBR_param_.dblLink6InertXX*power(sin(q1),2)*power(sin(q2),2)*sin(2*q4)*sin(q5) + 3*KUKA_LBR_param_.dblLink6InertYY*power(sin(q1),2)*power(sin(q2),2)*sin(2*q4)*sin(q5) + KUKA_LBR_param_.dblLink6InertYY*power(cos(q3),2)*power(sin(q1),2)*power(sin(q2),2)*sin(2*q4)*sin(q5) + 6*KUKA_LBR_param_.dblLink6InertXY*sin(2*q1)*power(sin(q2),2)*sin(2*q4)*sin(q5) + 2*KUKA_LBR_param_.dblLink6InertXY*power(cos(q3),2)*sin(2*q1)*power(sin(q2),2)*sin(2*q4)*sin(q5) + 12*KUKA_LBR_param_.dblLink6InertYZ*sin(q1)*sin(2*q2)*sin(2*q4)*sin(q5) + 4*KUKA_LBR_param_.dblLink6InertYZ*power(cos(q3),2)*sin(q1)*sin(2*q2)*sin(2*q4)*sin(q5) - 3*KUKA_LBR_param_.dblLink6InertXX*power(sin(q1),2)*power(sin(q3),2)*sin(2*q4)*sin(q5) + 3*KUKA_LBR_param_.dblLink6InertYY*power(sin(q1),2)*power(sin(q3),2)*sin(2*q4)*sin(q5) + 6*KUKA_LBR_param_.dblLink6InertXY*sin(2*q1)*power(sin(q3),2)*sin(2*q4)*sin(q5) + KUKA_LBR_param_.dblLink6InertXX*power(sin(q1),2)*power(sin(q2),2)*power(sin(q3),2)*sin(2*q4)*sin(q5) - 2*KUKA_LBR_param_.dblLink6InertXY*sin(2*q1)*power(sin(q2),2)*power(sin(q3),2)*sin(2*q4)*sin(q5) - 4*KUKA_LBR_param_.dblLink6InertYZ*sin(q1)*sin(2*q2)*power(sin(q3),2)*sin(2*q4)*sin(q5) - 8*KUKA_LBR_param_.dblLink6InertXZ*sin(q1)*sin(q2)*sin(2*q3)*sin(2*q4)*sin(q5) + 4*cos(q2)*(4*KUKA_LBR_param_.dblLink6InertXZ*cos(q3)*cos(q4)*cos(q5)*sin(q1) - 4*KUKA_LBR_param_.dblLink6InertXY*power(cos(q3),2)*cos(q5)*power(sin(q1),2)*sin(q4) + 4*KUKA_LBR_param_.dblLink6InertXY*cos(q5)*power(sin(q1),2)*power(sin(q3),2)*sin(q4) + (-4*KUKA_LBR_param_.dblLink6InertXZ*power(cos(q4),2)*sin(q1)*sin(q3) + 4*KUKA_LBR_param_.dblLink6InertXZ*sin(q1)*sin(q3)*power(sin(q4),2) + 2*KUKA_LBR_param_.dblLink6InertXY*power(sin(q1),2)*sin(2*q3)*sin(2*q4) + (KUKA_LBR_param_.dblLink6InertXX - KUKA_LBR_param_.dblLink6InertYY)*sin(2*q1)*sin(2*q3)*sin(2*q4))*sin(q5)) + power(cos(q2),2)*(-2*KUKA_LBR_param_.dblLink6InertXX*cos(q5)*sin(2*q3)*sin(q4) - 2*KUKA_LBR_param_.dblLink6InertYY*cos(q5)*sin(2*q3)*sin(q4) + 4*KUKA_LBR_param_.dblLink6InertZZ*cos(q5)*sin(2*q3)*sin(q4) - 2*KUKA_LBR_param_.dblLink6InertYY*cos(q5)*power(sin(q1),2)*sin(2*q3)*sin(q4) - 4*KUKA_LBR_param_.dblLink6InertXY*cos(q5)*sin(2*q1)*sin(2*q3)*sin(q4) + 16*KUKA_LBR_param_.dblLink6InertYZ*cos(q3)*power(cos(q4),2)*sin(q1)*sin(q5) - 3*KUKA_LBR_param_.dblLink6InertXX*sin(2*q4)*sin(q5) - 3*KUKA_LBR_param_.dblLink6InertYY*sin(2*q4)*sin(q5) + 6*KUKA_LBR_param_.dblLink6InertZZ*sin(2*q4)*sin(q5) + 3*KUKA_LBR_param_.dblLink6InertXX*power(sin(q1),2)*sin(2*q4)*sin(q5) - 3*KUKA_LBR_param_.dblLink6InertYY*power(sin(q1),2)*sin(2*q4)*sin(q5) + power(cos(q3),2)*sin(q1)*(-4*KUKA_LBR_param_.dblLink6InertXY*cos(q1) + KUKA_LBR_param_.dblLink6InertXX*sin(q1))*sin(2*q4)*sin(q5) - 6*KUKA_LBR_param_.dblLink6InertXY*sin(2*q1)*sin(2*q4)*sin(q5) + KUKA_LBR_param_.dblLink6InertXX*power(sin(q3),2)*sin(2*q4)*sin(q5) + KUKA_LBR_param_.dblLink6InertYY*power(sin(q3),2)*sin(2*q4)*sin(q5) - 2*KUKA_LBR_param_.dblLink6InertZZ*power(sin(q3),2)*sin(2*q4)*sin(q5) + KUKA_LBR_param_.dblLink6InertYY*power(sin(q1),2)*power(sin(q3),2)*sin(2*q4)*sin(q5) + 2*KUKA_LBR_param_.dblLink6InertXY*sin(2*q1)*power(sin(q3),2)*sin(2*q4)*sin(q5) + 4*cos(q3)*sin(q1)*sin(q4)*(KUKA_LBR_param_.dblLink6InertXX*cos(q5)*sin(q1)*sin(q3) - 4*KUKA_LBR_param_.dblLink6InertYZ*sin(q4)*sin(q5)) + 2*cos(q4)*(8*KUKA_LBR_param_.dblLink6InertYZ*cos(q5)*sin(q1)*sin(q3) - (power(cos(q3),2)*(KUKA_LBR_param_.dblLink6InertXX + KUKA_LBR_param_.dblLink6InertYY - 2*KUKA_LBR_param_.dblLink6InertZZ + KUKA_LBR_param_.dblLink6InertYY*power(sin(q1),2)) + KUKA_LBR_param_.dblLink6InertXX*power(sin(q1),2)*power(sin(q3),2))*sin(q4)*sin(q5))) + 16*KUKA_LBR_param_.dblLink6CogX*KUKA_LBR_param_.dblLink6CogZ*KUKA_LBR_param_.dblLink6Mass*sin(q6)))/32.0 - KUKA_LBR_param_.dblLink7Mass*(cos(q5)*(KUKA_LBR_param_.dblLink7CogZ*sin(q2)*sin(q3)*sin(q6) + cos(q2)*sin(q4)*(KUKA_LBR_param_.dblLink7CogY*cos(q7) + KUKA_LBR_param_.dblLink7CogX*sin(q7)) - cos(q6)*sin(q2)*sin(q3)*(KUKA_LBR_param_.dblLink7CogX*cos(q7) - KUKA_LBR_param_.dblLink7CogY*sin(q7))) + sin(q5)*(cos(q7)*(KUKA_LBR_param_.dblLink7CogY*sin(q2)*sin(q3) + KUKA_LBR_param_.dblLink7CogX*cos(q2)*cos(q6)*sin(q4)) + KUKA_LBR_param_.dblLink7CogX*sin(q2)*sin(q3)*sin(q7) - cos(q2)*sin(q4)*(KUKA_LBR_param_.dblLink7CogZ*sin(q6) + KUKA_LBR_param_.dblLink7CogY*cos(q6)*sin(q7))) - cos(q3)*cos(q4)*sin(q2)*(cos(q5)*(KUKA_LBR_param_.dblLink7CogY*cos(q7) + KUKA_LBR_param_.dblLink7CogX*sin(q7)) - sin(q5)*(KUKA_LBR_param_.dblLink7CogZ*sin(q6) + cos(q6)*(-(KUKA_LBR_param_.dblLink7CogX*cos(q7)) + KUKA_LBR_param_.dblLink7CogY*sin(q7)))))*(cos(q2)*(cos(q4)*(-(KUKA_LBR_param_.dblLink7CogX*cos(q6)*cos(q7)) + KUKA_LBR_param_.dblLink7CogZ*sin(q6) + KUKA_LBR_param_.dblLink7CogY*cos(q6)*sin(q7)) - cos(q5)*sin(q4)*(KUKA_LBR_param_.dblLink7CogZ*cos(q6) + KUKA_LBR_param_.dblLink7CogX*cos(q7)*sin(q6) - KUKA_LBR_param_.dblLink7CogY*sin(q6)*sin(q7))) + sin(q2)*(-(sin(q3)*sin(q5)*(KUKA_LBR_param_.dblLink7CogZ*cos(q6) + sin(q6)*(KUKA_LBR_param_.dblLink7CogX*cos(q7) - KUKA_LBR_param_.dblLink7CogY*sin(q7)))) + cos(q3)*(sin(q4)*(-(KUKA_LBR_param_.dblLink7CogX*cos(q6)*cos(q7)) + KUKA_LBR_param_.dblLink7CogZ*sin(q6) + KUKA_LBR_param_.dblLink7CogY*cos(q6)*sin(q7)) + cos(q4)*cos(q5)*(KUKA_LBR_param_.dblLink7CogZ*cos(q6) + KUKA_LBR_param_.dblLink7CogX*cos(q7)*sin(q6) - KUKA_LBR_param_.dblLink7CogY*sin(q6)*sin(q7))))) + KUKA_LBR_param_.dblLink7Mass*(KUKA_LBR_param_.dblLink7CogZ*cos(q5)*cos(q6)*sin(q1)*sin(q2)*sin(q4) - KUKA_LBR_param_.dblLink7CogX*cos(q1)*cos(q6)*cos(q7)*sin(q3)*sin(q4) + KUKA_LBR_param_.dblLink7CogZ*cos(q1)*cos(q3)*cos(q6)*sin(q5) + KUKA_LBR_param_.dblLink7CogX*cos(q5)*cos(q7)*sin(q1)*sin(q2)*sin(q4)*sin(q6) + KUKA_LBR_param_.dblLink7CogZ*cos(q1)*sin(q3)*sin(q4)*sin(q6) + KUKA_LBR_param_.dblLink7CogX*cos(q1)*cos(q3)*cos(q7)*sin(q5)*sin(q6) + KUKA_LBR_param_.dblLink7CogY*cos(q1)*cos(q6)*sin(q3)*sin(q4)*sin(q7) - KUKA_LBR_param_.dblLink7CogY*cos(q5)*sin(q1)*sin(q2)*sin(q4)*sin(q6)*sin(q7) - KUKA_LBR_param_.dblLink7CogY*cos(q1)*cos(q3)*sin(q5)*sin(q6)*sin(q7) + cos(q4)*(cos(q6)*(KUKA_LBR_param_.dblLink7CogX*cos(q7)*sin(q1)*sin(q2) + KUKA_LBR_param_.dblLink7CogZ*cos(q1)*cos(q5)*sin(q3) - KUKA_LBR_param_.dblLink7CogY*sin(q1)*sin(q2)*sin(q7)) - sin(q6)*(KUKA_LBR_param_.dblLink7CogZ*sin(q1)*sin(q2) + cos(q1)*cos(q5)*sin(q3)*(-(KUKA_LBR_param_.dblLink7CogX*cos(q7)) + KUKA_LBR_param_.dblLink7CogY*sin(q7)))) + cos(q2)*sin(q1)*(-(sin(q3)*sin(q5)*(KUKA_LBR_param_.dblLink7CogZ*cos(q6) + sin(q6)*(KUKA_LBR_param_.dblLink7CogX*cos(q7) - KUKA_LBR_param_.dblLink7CogY*sin(q7)))) + cos(q3)*(sin(q4)*(-(KUKA_LBR_param_.dblLink7CogX*cos(q6)*cos(q7)) + KUKA_LBR_param_.dblLink7CogZ*sin(q6) + KUKA_LBR_param_.dblLink7CogY*cos(q6)*sin(q7)) + cos(q4)*cos(q5)*(KUKA_LBR_param_.dblLink7CogZ*cos(q6) + KUKA_LBR_param_.dblLink7CogX*cos(q7)*sin(q6) - KUKA_LBR_param_.dblLink7CogY*sin(q6)*sin(q7)))))*(cos(q1)*(cos(q4)*sin(q3)*(cos(q5)*(KUKA_LBR_param_.dblLink7CogY*cos(q7) + KUKA_LBR_param_.dblLink7CogX*sin(q7)) + sin(q5)*(KUKA_LBR_param_.dblLink7CogX*cos(q6)*cos(q7) - KUKA_LBR_param_.dblLink7CogZ*sin(q6) - KUKA_LBR_param_.dblLink7CogY*cos(q6)*sin(q7))) + cos(q3)*(sin(q5)*(KUKA_LBR_param_.dblLink7CogY*cos(q7) + KUKA_LBR_param_.dblLink7CogX*sin(q7)) + cos(q5)*(-(KUKA_LBR_param_.dblLink7CogX*cos(q6)*cos(q7)) + KUKA_LBR_param_.dblLink7CogZ*sin(q6) + KUKA_LBR_param_.dblLink7CogY*cos(q6)*sin(q7)))) + sin(q1)*(sin(q2)*sin(q4)*(cos(q5)*(KUKA_LBR_param_.dblLink7CogY*cos(q7) + KUKA_LBR_param_.dblLink7CogX*sin(q7)) + sin(q5)*(KUKA_LBR_param_.dblLink7CogX*cos(q6)*cos(q7) - KUKA_LBR_param_.dblLink7CogZ*sin(q6) - KUKA_LBR_param_.dblLink7CogY*cos(q6)*sin(q7))) + cos(q2)*(cos(q3)*cos(q4)*(cos(q5)*(KUKA_LBR_param_.dblLink7CogY*cos(q7) + KUKA_LBR_param_.dblLink7CogX*sin(q7)) + sin(q5)*(KUKA_LBR_param_.dblLink7CogX*cos(q6)*cos(q7) - KUKA_LBR_param_.dblLink7CogZ*sin(q6) - KUKA_LBR_param_.dblLink7CogY*cos(q6)*sin(q7))) - sin(q3)*(sin(q5)*(KUKA_LBR_param_.dblLink7CogY*cos(q7) + KUKA_LBR_param_.dblLink7CogX*sin(q7)) + cos(q5)*(-(KUKA_LBR_param_.dblLink7CogX*cos(q6)*cos(q7)) + KUKA_LBR_param_.dblLink7CogZ*sin(q6) + KUKA_LBR_param_.dblLink7CogY*cos(q6)*sin(q7)))))) - KUKA_LBR_param_.dblLink7Mass*(sin(q1)*(-(cos(q4)*sin(q3)*(cos(q5)*(KUKA_LBR_param_.dblLink7CogY*cos(q7) + KUKA_LBR_param_.dblLink7CogX*sin(q7)) + sin(q5)*(KUKA_LBR_param_.dblLink7CogX*cos(q6)*cos(q7) - KUKA_LBR_param_.dblLink7CogZ*sin(q6) - KUKA_LBR_param_.dblLink7CogY*cos(q6)*sin(q7)))) - cos(q3)*(sin(q5)*(KUKA_LBR_param_.dblLink7CogY*cos(q7) + KUKA_LBR_param_.dblLink7CogX*sin(q7)) + cos(q5)*(-(KUKA_LBR_param_.dblLink7CogX*cos(q6)*cos(q7)) + KUKA_LBR_param_.dblLink7CogZ*sin(q6) + KUKA_LBR_param_.dblLink7CogY*cos(q6)*sin(q7)))) + cos(q1)*(sin(q2)*sin(q4)*(cos(q5)*(KUKA_LBR_param_.dblLink7CogY*cos(q7) + KUKA_LBR_param_.dblLink7CogX*sin(q7)) + sin(q5)*(KUKA_LBR_param_.dblLink7CogX*cos(q6)*cos(q7) - KUKA_LBR_param_.dblLink7CogZ*sin(q6) - KUKA_LBR_param_.dblLink7CogY*cos(q6)*sin(q7))) + cos(q2)*(cos(q3)*cos(q4)*(cos(q5)*(KUKA_LBR_param_.dblLink7CogY*cos(q7) + KUKA_LBR_param_.dblLink7CogX*sin(q7)) + sin(q5)*(KUKA_LBR_param_.dblLink7CogX*cos(q6)*cos(q7) - KUKA_LBR_param_.dblLink7CogZ*sin(q6) - KUKA_LBR_param_.dblLink7CogY*cos(q6)*sin(q7))) - sin(q3)*(sin(q5)*(KUKA_LBR_param_.dblLink7CogY*cos(q7) + KUKA_LBR_param_.dblLink7CogX*sin(q7)) + cos(q5)*(-(KUKA_LBR_param_.dblLink7CogX*cos(q6)*cos(q7)) + KUKA_LBR_param_.dblLink7CogZ*sin(q6) + KUKA_LBR_param_.dblLink7CogY*cos(q6)*sin(q7))))))*(sin(q1)*(cos(q6)*(-(KUKA_LBR_param_.dblLink7CogX*cos(q7)*sin(q3)*sin(q4)) + KUKA_LBR_param_.dblLink7CogZ*cos(q3)*sin(q5) + KUKA_LBR_param_.dblLink7CogY*sin(q3)*sin(q4)*sin(q7)) + sin(q6)*(KUKA_LBR_param_.dblLink7CogZ*sin(q3)*sin(q4) + cos(q3)*sin(q5)*(KUKA_LBR_param_.dblLink7CogX*cos(q7) - KUKA_LBR_param_.dblLink7CogY*sin(q7))) + cos(q4)*cos(q5)*sin(q3)*(KUKA_LBR_param_.dblLink7CogZ*cos(q6) + sin(q6)*(KUKA_LBR_param_.dblLink7CogX*cos(q7) - KUKA_LBR_param_.dblLink7CogY*sin(q7)))) - cos(q1)*(sin(q2)*(cos(q4)*(KUKA_LBR_param_.dblLink7CogX*cos(q6)*cos(q7) - KUKA_LBR_param_.dblLink7CogZ*sin(q6) - KUKA_LBR_param_.dblLink7CogY*cos(q6)*sin(q7)) + cos(q5)*sin(q4)*(KUKA_LBR_param_.dblLink7CogZ*cos(q6) + KUKA_LBR_param_.dblLink7CogX*cos(q7)*sin(q6) - KUKA_LBR_param_.dblLink7CogY*sin(q6)*sin(q7))) + cos(q2)*(-(sin(q3)*sin(q5)*(KUKA_LBR_param_.dblLink7CogZ*cos(q6) + sin(q6)*(KUKA_LBR_param_.dblLink7CogX*cos(q7) - KUKA_LBR_param_.dblLink7CogY*sin(q7)))) + cos(q3)*(sin(q4)*(-(KUKA_LBR_param_.dblLink7CogX*cos(q6)*cos(q7)) + KUKA_LBR_param_.dblLink7CogZ*sin(q6) + KUKA_LBR_param_.dblLink7CogY*cos(q6)*sin(q7)) + cos(q4)*cos(q5)*(KUKA_LBR_param_.dblLink7CogZ*cos(q6) + KUKA_LBR_param_.dblLink7CogX*cos(q7)*sin(q6) - KUKA_LBR_param_.dblLink7CogY*sin(q6)*sin(q7))))));
dblMassInertFullRow6Col6 = (-(cos(q5)*(cos(q3)*sin(q1) + cos(q1)*cos(q2)*sin(q3))) + (cos(q4)*sin(q1)*sin(q3) - cos(q1)*(cos(q2)*cos(q3)*cos(q4) + sin(q2)*sin(q4)))*sin(q5))*(KUKA_LBR_param_.dblLink6InertXZ*(cos(q5)*sin(q2)*sin(q3) + (cos(q3)*cos(q4)*sin(q2) - cos(q2)*sin(q4))*sin(q5)) + KUKA_LBR_param_.dblLink6InertXX*(-(cos(q5)*(cos(q3)*sin(q1) + cos(q1)*cos(q2)*sin(q3))) + (cos(q4)*sin(q1)*sin(q3) - cos(q1)*(cos(q2)*cos(q3)*cos(q4) + sin(q2)*sin(q4)))*sin(q5)) + KUKA_LBR_param_.dblLink6InertXY*(cos(q1)*(cos(q3)*cos(q5) - cos(q4)*sin(q3)*sin(q5)) - sin(q1)*(sin(q2)*sin(q4)*sin(q5) + cos(q2)*(cos(q5)*sin(q3) + cos(q3)*cos(q4)*sin(q5))))) + (cos(q1)*(cos(q3)*cos(q5) - cos(q4)*sin(q3)*sin(q5)) - sin(q1)*(sin(q2)*sin(q4)*sin(q5) + cos(q2)*(cos(q5)*sin(q3) + cos(q3)*cos(q4)*sin(q5))))*(KUKA_LBR_param_.dblLink6InertYZ*(cos(q5)*sin(q2)*sin(q3) + (cos(q3)*cos(q4)*sin(q2) - cos(q2)*sin(q4))*sin(q5)) + KUKA_LBR_param_.dblLink6InertXY*(-(cos(q5)*(cos(q3)*sin(q1) + cos(q1)*cos(q2)*sin(q3))) + (cos(q4)*sin(q1)*sin(q3) - cos(q1)*(cos(q2)*cos(q3)*cos(q4) + sin(q2)*sin(q4)))*sin(q5)) + KUKA_LBR_param_.dblLink6InertYY*(cos(q1)*(cos(q3)*cos(q5) - cos(q4)*sin(q3)*sin(q5)) - sin(q1)*(sin(q2)*sin(q4)*sin(q5) + cos(q2)*(cos(q5)*sin(q3) + cos(q3)*cos(q4)*sin(q5))))) + (cos(q5)*sin(q2)*sin(q3) + (cos(q3)*cos(q4)*sin(q2) - cos(q2)*sin(q4))*sin(q5))*(KUKA_LBR_param_.dblLink6InertZZ*(cos(q5)*sin(q2)*sin(q3) + (cos(q3)*cos(q4)*sin(q2) - cos(q2)*sin(q4))*sin(q5)) + KUKA_LBR_param_.dblLink6InertXZ*(-(cos(q5)*(cos(q3)*sin(q1) + cos(q1)*cos(q2)*sin(q3))) + (cos(q4)*sin(q1)*sin(q3) - cos(q1)*(cos(q2)*cos(q3)*cos(q4) + sin(q2)*sin(q4)))*sin(q5)) + KUKA_LBR_param_.dblLink6InertYZ*(cos(q1)*(cos(q3)*cos(q5) - cos(q4)*sin(q3)*sin(q5)) - sin(q1)*(sin(q2)*sin(q4)*sin(q5) + cos(q2)*(cos(q5)*sin(q3) + cos(q3)*cos(q4)*sin(q5))))) + (-(cos(q5)*(cos(q3)*sin(q1) + cos(q1)*cos(q2)*sin(q3))) + (cos(q4)*sin(q1)*sin(q3) - cos(q1)*(cos(q2)*cos(q3)*cos(q4) + sin(q2)*sin(q4)))*sin(q5))*(KUKA_LBR_param_.dblLink7InertXZ*(cos(q5)*sin(q2)*sin(q3) + (cos(q3)*cos(q4)*sin(q2) - cos(q2)*sin(q4))*sin(q5)) + KUKA_LBR_param_.dblLink7InertXX*(-(cos(q5)*(cos(q3)*sin(q1) + cos(q1)*cos(q2)*sin(q3))) + (cos(q4)*sin(q1)*sin(q3) - cos(q1)*(cos(q2)*cos(q3)*cos(q4) + sin(q2)*sin(q4)))*sin(q5)) + KUKA_LBR_param_.dblLink7InertXY*(cos(q1)*(cos(q3)*cos(q5) - cos(q4)*sin(q3)*sin(q5)) - sin(q1)*(sin(q2)*sin(q4)*sin(q5) + cos(q2)*(cos(q5)*sin(q3) + cos(q3)*cos(q4)*sin(q5))))) + (cos(q1)*(cos(q3)*cos(q5) - cos(q4)*sin(q3)*sin(q5)) - sin(q1)*(sin(q2)*sin(q4)*sin(q5) + cos(q2)*(cos(q5)*sin(q3) + cos(q3)*cos(q4)*sin(q5))))*(KUKA_LBR_param_.dblLink7InertYZ*(cos(q5)*sin(q2)*sin(q3) + (cos(q3)*cos(q4)*sin(q2) - cos(q2)*sin(q4))*sin(q5)) + KUKA_LBR_param_.dblLink7InertXY*(-(cos(q5)*(cos(q3)*sin(q1) + cos(q1)*cos(q2)*sin(q3))) + (cos(q4)*sin(q1)*sin(q3) - cos(q1)*(cos(q2)*cos(q3)*cos(q4) + sin(q2)*sin(q4)))*sin(q5)) + KUKA_LBR_param_.dblLink7InertYY*(cos(q1)*(cos(q3)*cos(q5) - cos(q4)*sin(q3)*sin(q5)) - sin(q1)*(sin(q2)*sin(q4)*sin(q5) + cos(q2)*(cos(q5)*sin(q3) + cos(q3)*cos(q4)*sin(q5))))) + (cos(q5)*sin(q2)*sin(q3) + (cos(q3)*cos(q4)*sin(q2) - cos(q2)*sin(q4))*sin(q5))*(KUKA_LBR_param_.dblLink7InertZZ*(cos(q5)*sin(q2)*sin(q3) + (cos(q3)*cos(q4)*sin(q2) - cos(q2)*sin(q4))*sin(q5)) + KUKA_LBR_param_.dblLink7InertXZ*(-(cos(q5)*(cos(q3)*sin(q1) + cos(q1)*cos(q2)*sin(q3))) + (cos(q4)*sin(q1)*sin(q3) - cos(q1)*(cos(q2)*cos(q3)*cos(q4) + sin(q2)*sin(q4)))*sin(q5)) + KUKA_LBR_param_.dblLink7InertYZ*(cos(q1)*(cos(q3)*cos(q5) - cos(q4)*sin(q3)*sin(q5)) - sin(q1)*(sin(q2)*sin(q4)*sin(q5) + cos(q2)*(cos(q5)*sin(q3) + cos(q3)*cos(q4)*sin(q5))))) + KUKA_LBR_param_.dblLink6Mass*power(cos(q2)*(cos(q5)*sin(q4)*(KUKA_LBR_param_.dblLink6CogY*cos(q6) + KUKA_LBR_param_.dblLink6CogX*sin(q6)) + cos(q4)*(KUKA_LBR_param_.dblLink6CogX*cos(q6) - KUKA_LBR_param_.dblLink6CogY*sin(q6))) + sin(q2)*(sin(q3)*sin(q5)*(KUKA_LBR_param_.dblLink6CogY*cos(q6) + KUKA_LBR_param_.dblLink6CogX*sin(q6)) - cos(q3)*(cos(q4)*cos(q5)*(KUKA_LBR_param_.dblLink6CogY*cos(q6) + KUKA_LBR_param_.dblLink6CogX*sin(q6)) + sin(q4)*(-(KUKA_LBR_param_.dblLink6CogX*cos(q6)) + KUKA_LBR_param_.dblLink6CogY*sin(q6)))),2) + KUKA_LBR_param_.dblLink6Mass*power(KUKA_LBR_param_.dblLink6CogY*cos(q5)*cos(q6)*sin(q1)*sin(q2)*sin(q4) - KUKA_LBR_param_.dblLink6CogX*cos(q1)*cos(q6)*sin(q3)*sin(q4) + KUKA_LBR_param_.dblLink6CogY*cos(q1)*cos(q3)*cos(q6)*sin(q5) + KUKA_LBR_param_.dblLink6CogX*cos(q5)*sin(q1)*sin(q2)*sin(q4)*sin(q6) + KUKA_LBR_param_.dblLink6CogY*cos(q1)*sin(q3)*sin(q4)*sin(q6) + KUKA_LBR_param_.dblLink6CogX*cos(q1)*cos(q3)*sin(q5)*sin(q6) + cos(q4)*(KUKA_LBR_param_.dblLink6CogX*cos(q6)*sin(q1)*sin(q2) + KUKA_LBR_param_.dblLink6CogY*cos(q1)*cos(q5)*cos(q6)*sin(q3) - KUKA_LBR_param_.dblLink6CogY*sin(q1)*sin(q2)*sin(q6) + KUKA_LBR_param_.dblLink6CogX*cos(q1)*cos(q5)*sin(q3)*sin(q6)) + cos(q2)*sin(q1)*(-(sin(q3)*sin(q5)*(KUKA_LBR_param_.dblLink6CogY*cos(q6) + KUKA_LBR_param_.dblLink6CogX*sin(q6))) + cos(q3)*(cos(q4)*cos(q5)*(KUKA_LBR_param_.dblLink6CogY*cos(q6) + KUKA_LBR_param_.dblLink6CogX*sin(q6)) + sin(q4)*(-(KUKA_LBR_param_.dblLink6CogX*cos(q6)) + KUKA_LBR_param_.dblLink6CogY*sin(q6)))),2) + KUKA_LBR_param_.dblLink6Mass*power(sin(q1)*(-(KUKA_LBR_param_.dblLink6CogX*cos(q6)*sin(q3)*sin(q4)) + KUKA_LBR_param_.dblLink6CogY*cos(q3)*cos(q6)*sin(q5) + KUKA_LBR_param_.dblLink6CogY*sin(q3)*sin(q4)*sin(q6) + KUKA_LBR_param_.dblLink6CogX*cos(q3)*sin(q5)*sin(q6) + cos(q4)*cos(q5)*sin(q3)*(KUKA_LBR_param_.dblLink6CogY*cos(q6) + KUKA_LBR_param_.dblLink6CogX*sin(q6))) - cos(q1)*(sin(q2)*(cos(q5)*sin(q4)*(KUKA_LBR_param_.dblLink6CogY*cos(q6) + KUKA_LBR_param_.dblLink6CogX*sin(q6)) + cos(q4)*(KUKA_LBR_param_.dblLink6CogX*cos(q6) - KUKA_LBR_param_.dblLink6CogY*sin(q6))) + cos(q2)*(-(sin(q3)*sin(q5)*(KUKA_LBR_param_.dblLink6CogY*cos(q6) + KUKA_LBR_param_.dblLink6CogX*sin(q6))) + cos(q3)*(cos(q4)*cos(q5)*(KUKA_LBR_param_.dblLink6CogY*cos(q6) + KUKA_LBR_param_.dblLink6CogX*sin(q6)) + sin(q4)*(-(KUKA_LBR_param_.dblLink6CogX*cos(q6)) + KUKA_LBR_param_.dblLink6CogY*sin(q6))))),2) + KUKA_LBR_param_.dblLink7Mass*power(KUKA_LBR_param_.dblLink7CogZ*cos(q5)*cos(q6)*sin(q1)*sin(q2)*sin(q4) - KUKA_LBR_param_.dblLink7CogX*cos(q1)*cos(q6)*cos(q7)*sin(q3)*sin(q4) + KUKA_LBR_param_.dblLink7CogZ*cos(q1)*cos(q3)*cos(q6)*sin(q5) + KUKA_LBR_param_.dblLink7CogX*cos(q5)*cos(q7)*sin(q1)*sin(q2)*sin(q4)*sin(q6) + KUKA_LBR_param_.dblLink7CogZ*cos(q1)*sin(q3)*sin(q4)*sin(q6) + KUKA_LBR_param_.dblLink7CogX*cos(q1)*cos(q3)*cos(q7)*sin(q5)*sin(q6) + KUKA_LBR_param_.dblLink7CogY*cos(q1)*cos(q6)*sin(q3)*sin(q4)*sin(q7) - KUKA_LBR_param_.dblLink7CogY*cos(q5)*sin(q1)*sin(q2)*sin(q4)*sin(q6)*sin(q7) - KUKA_LBR_param_.dblLink7CogY*cos(q1)*cos(q3)*sin(q5)*sin(q6)*sin(q7) + cos(q4)*(cos(q6)*(KUKA_LBR_param_.dblLink7CogX*cos(q7)*sin(q1)*sin(q2) + KUKA_LBR_param_.dblLink7CogZ*cos(q1)*cos(q5)*sin(q3) - KUKA_LBR_param_.dblLink7CogY*sin(q1)*sin(q2)*sin(q7)) - sin(q6)*(KUKA_LBR_param_.dblLink7CogZ*sin(q1)*sin(q2) + cos(q1)*cos(q5)*sin(q3)*(-(KUKA_LBR_param_.dblLink7CogX*cos(q7)) + KUKA_LBR_param_.dblLink7CogY*sin(q7)))) + cos(q2)*sin(q1)*(-(sin(q3)*sin(q5)*(KUKA_LBR_param_.dblLink7CogZ*cos(q6) + sin(q6)*(KUKA_LBR_param_.dblLink7CogX*cos(q7) - KUKA_LBR_param_.dblLink7CogY*sin(q7)))) + cos(q3)*(sin(q4)*(-(KUKA_LBR_param_.dblLink7CogX*cos(q6)*cos(q7)) + KUKA_LBR_param_.dblLink7CogZ*sin(q6) + KUKA_LBR_param_.dblLink7CogY*cos(q6)*sin(q7)) + cos(q4)*cos(q5)*(KUKA_LBR_param_.dblLink7CogZ*cos(q6) + KUKA_LBR_param_.dblLink7CogX*cos(q7)*sin(q6) - KUKA_LBR_param_.dblLink7CogY*sin(q6)*sin(q7)))),2) + KUKA_LBR_param_.dblLink7Mass*power(cos(q2)*(cos(q4)*(KUKA_LBR_param_.dblLink7CogX*cos(q6)*cos(q7) - KUKA_LBR_param_.dblLink7CogZ*sin(q6) - KUKA_LBR_param_.dblLink7CogY*cos(q6)*sin(q7)) + cos(q5)*sin(q4)*(KUKA_LBR_param_.dblLink7CogZ*cos(q6) + KUKA_LBR_param_.dblLink7CogX*cos(q7)*sin(q6) - KUKA_LBR_param_.dblLink7CogY*sin(q6)*sin(q7))) - sin(q2)*(-(sin(q3)*sin(q5)*(KUKA_LBR_param_.dblLink7CogZ*cos(q6) + sin(q6)*(KUKA_LBR_param_.dblLink7CogX*cos(q7) - KUKA_LBR_param_.dblLink7CogY*sin(q7)))) + cos(q3)*(sin(q4)*(-(KUKA_LBR_param_.dblLink7CogX*cos(q6)*cos(q7)) + KUKA_LBR_param_.dblLink7CogZ*sin(q6) + KUKA_LBR_param_.dblLink7CogY*cos(q6)*sin(q7)) + cos(q4)*cos(q5)*(KUKA_LBR_param_.dblLink7CogZ*cos(q6) + KUKA_LBR_param_.dblLink7CogX*cos(q7)*sin(q6) - KUKA_LBR_param_.dblLink7CogY*sin(q6)*sin(q7)))),2) + KUKA_LBR_param_.dblLink7Mass*power(sin(q1)*(cos(q6)*(-(KUKA_LBR_param_.dblLink7CogX*cos(q7)*sin(q3)*sin(q4)) + KUKA_LBR_param_.dblLink7CogZ*cos(q3)*sin(q5) + KUKA_LBR_param_.dblLink7CogY*sin(q3)*sin(q4)*sin(q7)) + sin(q6)*(KUKA_LBR_param_.dblLink7CogZ*sin(q3)*sin(q4) + cos(q3)*sin(q5)*(KUKA_LBR_param_.dblLink7CogX*cos(q7) - KUKA_LBR_param_.dblLink7CogY*sin(q7))) + cos(q4)*cos(q5)*sin(q3)*(KUKA_LBR_param_.dblLink7CogZ*cos(q6) + sin(q6)*(KUKA_LBR_param_.dblLink7CogX*cos(q7) - KUKA_LBR_param_.dblLink7CogY*sin(q7)))) - cos(q1)*(sin(q2)*(cos(q4)*(KUKA_LBR_param_.dblLink7CogX*cos(q6)*cos(q7) - KUKA_LBR_param_.dblLink7CogZ*sin(q6) - KUKA_LBR_param_.dblLink7CogY*cos(q6)*sin(q7)) + cos(q5)*sin(q4)*(KUKA_LBR_param_.dblLink7CogZ*cos(q6) + KUKA_LBR_param_.dblLink7CogX*cos(q7)*sin(q6) - KUKA_LBR_param_.dblLink7CogY*sin(q6)*sin(q7))) + cos(q2)*(-(sin(q3)*sin(q5)*(KUKA_LBR_param_.dblLink7CogZ*cos(q6) + sin(q6)*(KUKA_LBR_param_.dblLink7CogX*cos(q7) - KUKA_LBR_param_.dblLink7CogY*sin(q7)))) + cos(q3)*(sin(q4)*(-(KUKA_LBR_param_.dblLink7CogX*cos(q6)*cos(q7)) + KUKA_LBR_param_.dblLink7CogZ*sin(q6) + KUKA_LBR_param_.dblLink7CogY*cos(q6)*sin(q7)) + cos(q4)*cos(q5)*(KUKA_LBR_param_.dblLink7CogZ*cos(q6) + KUKA_LBR_param_.dblLink7CogX*cos(q7)*sin(q6) - KUKA_LBR_param_.dblLink7CogY*sin(q6)*sin(q7))))),2);
dblMassInertFullRow6Col7 = (KUKA_LBR_param_.dblLink7InertXZ*(cos(q5)*sin(q2)*sin(q3) + (cos(q3)*cos(q4)*sin(q2) - cos(q2)*sin(q4))*sin(q5)) + KUKA_LBR_param_.dblLink7InertXX*(-(cos(q5)*(cos(q3)*sin(q1) + cos(q1)*cos(q2)*sin(q3))) + (cos(q4)*sin(q1)*sin(q3) - cos(q1)*(cos(q2)*cos(q3)*cos(q4) + sin(q2)*sin(q4)))*sin(q5)) + KUKA_LBR_param_.dblLink7InertXY*(cos(q1)*(cos(q3)*cos(q5) - cos(q4)*sin(q3)*sin(q5)) - sin(q1)*(sin(q2)*sin(q4)*sin(q5) + cos(q2)*(cos(q5)*sin(q3) + cos(q3)*cos(q4)*sin(q5)))))*(cos(q6)*(sin(q1)*sin(q3)*sin(q4) + cos(q1)*(cos(q4)*sin(q2) - cos(q2)*cos(q3)*sin(q4))) - (cos(q5)*(cos(q4)*sin(q1)*sin(q3) - cos(q1)*(cos(q2)*cos(q3)*cos(q4) + sin(q2)*sin(q4))) + (cos(q3)*sin(q1) + cos(q1)*cos(q2)*sin(q3))*sin(q5))*sin(q6)) + (KUKA_LBR_param_.dblLink7InertYZ*(cos(q5)*sin(q2)*sin(q3) + (cos(q3)*cos(q4)*sin(q2) - cos(q2)*sin(q4))*sin(q5)) + KUKA_LBR_param_.dblLink7InertXY*(-(cos(q5)*(cos(q3)*sin(q1) + cos(q1)*cos(q2)*sin(q3))) + (cos(q4)*sin(q1)*sin(q3) - cos(q1)*(cos(q2)*cos(q3)*cos(q4) + sin(q2)*sin(q4)))*sin(q5)) + KUKA_LBR_param_.dblLink7InertYY*(cos(q1)*(cos(q3)*cos(q5) - cos(q4)*sin(q3)*sin(q5)) - sin(q1)*(sin(q2)*sin(q4)*sin(q5) + cos(q2)*(cos(q5)*sin(q3) + cos(q3)*cos(q4)*sin(q5)))))*(cos(q6)*(cos(q4)*sin(q1)*sin(q2) - (cos(q2)*cos(q3)*sin(q1) + cos(q1)*sin(q3))*sin(q4)) + (cos(q5)*sin(q1)*sin(q2)*sin(q4) + cos(q1)*(cos(q4)*cos(q5)*sin(q3) + cos(q3)*sin(q5)) + cos(q2)*sin(q1)*(cos(q3)*cos(q4)*cos(q5) - sin(q3)*sin(q5)))*sin(q6)) + (KUKA_LBR_param_.dblLink7InertZZ*(cos(q5)*sin(q2)*sin(q3) + (cos(q3)*cos(q4)*sin(q2) - cos(q2)*sin(q4))*sin(q5)) + KUKA_LBR_param_.dblLink7InertXZ*(-(cos(q5)*(cos(q3)*sin(q1) + cos(q1)*cos(q2)*sin(q3))) + (cos(q4)*sin(q1)*sin(q3) - cos(q1)*(cos(q2)*cos(q3)*cos(q4) + sin(q2)*sin(q4)))*sin(q5)) + KUKA_LBR_param_.dblLink7InertYZ*(cos(q1)*(cos(q3)*cos(q5) - cos(q4)*sin(q3)*sin(q5)) - sin(q1)*(sin(q2)*sin(q4)*sin(q5) + cos(q2)*(cos(q5)*sin(q3) + cos(q3)*cos(q4)*sin(q5)))))*(cos(q2)*(cos(q4)*cos(q6) + cos(q5)*sin(q4)*sin(q6)) + sin(q2)*(sin(q3)*sin(q5)*sin(q6) + cos(q3)*(cos(q6)*sin(q4) - cos(q4)*cos(q5)*sin(q6)))) - KUKA_LBR_param_.dblLink7Mass*(-(KUKA_LBR_param_.dblLink7CogY*cos(q6)*cos(q7)*sin(q2)*sin(q3)*sin(q5)) - KUKA_LBR_param_.dblLink7CogX*cos(q2)*cos(q7)*sin(q4)*sin(q5) + KUKA_LBR_param_.dblLink7CogY*cos(q2)*cos(q4)*cos(q7)*sin(q6) - KUKA_LBR_param_.dblLink7CogX*cos(q6)*sin(q2)*sin(q3)*sin(q5)*sin(q7) + KUKA_LBR_param_.dblLink7CogY*cos(q2)*sin(q4)*sin(q5)*sin(q7) + KUKA_LBR_param_.dblLink7CogX*cos(q2)*cos(q4)*sin(q6)*sin(q7) + cos(q5)*(cos(q7)*(KUKA_LBR_param_.dblLink7CogX*sin(q2)*sin(q3) - KUKA_LBR_param_.dblLink7CogY*cos(q2)*cos(q6)*sin(q4)) - (KUKA_LBR_param_.dblLink7CogY*sin(q2)*sin(q3) + KUKA_LBR_param_.dblLink7CogX*cos(q2)*cos(q6)*sin(q4))*sin(q7)) + cos(q3)*sin(q2)*(sin(q4)*sin(q6)*(KUKA_LBR_param_.dblLink7CogY*cos(q7) + KUKA_LBR_param_.dblLink7CogX*sin(q7)) + cos(q4)*(cos(q5)*cos(q6)*(KUKA_LBR_param_.dblLink7CogY*cos(q7) + KUKA_LBR_param_.dblLink7CogX*sin(q7)) + sin(q5)*(KUKA_LBR_param_.dblLink7CogX*cos(q7) - KUKA_LBR_param_.dblLink7CogY*sin(q7)))))*(cos(q2)*(cos(q4)*(KUKA_LBR_param_.dblLink7CogX*cos(q6)*cos(q7) - KUKA_LBR_param_.dblLink7CogZ*sin(q6) - KUKA_LBR_param_.dblLink7CogY*cos(q6)*sin(q7)) + cos(q5)*sin(q4)*(KUKA_LBR_param_.dblLink7CogZ*cos(q6) + KUKA_LBR_param_.dblLink7CogX*cos(q7)*sin(q6) - KUKA_LBR_param_.dblLink7CogY*sin(q6)*sin(q7))) - sin(q2)*(-(sin(q3)*sin(q5)*(KUKA_LBR_param_.dblLink7CogZ*cos(q6) + sin(q6)*(KUKA_LBR_param_.dblLink7CogX*cos(q7) - KUKA_LBR_param_.dblLink7CogY*sin(q7)))) + cos(q3)*(sin(q4)*(-(KUKA_LBR_param_.dblLink7CogX*cos(q6)*cos(q7)) + KUKA_LBR_param_.dblLink7CogZ*sin(q6) + KUKA_LBR_param_.dblLink7CogY*cos(q6)*sin(q7)) + cos(q4)*cos(q5)*(KUKA_LBR_param_.dblLink7CogZ*cos(q6) + KUKA_LBR_param_.dblLink7CogX*cos(q7)*sin(q6) - KUKA_LBR_param_.dblLink7CogY*sin(q6)*sin(q7))))) + KUKA_LBR_param_.dblLink7Mass*(-(sin(q1)*(cos(q6)*(-(KUKA_LBR_param_.dblLink7CogX*cos(q7)*sin(q3)*sin(q4)) + KUKA_LBR_param_.dblLink7CogZ*cos(q3)*sin(q5) + KUKA_LBR_param_.dblLink7CogY*sin(q3)*sin(q4)*sin(q7)) + sin(q6)*(KUKA_LBR_param_.dblLink7CogZ*sin(q3)*sin(q4) + cos(q3)*sin(q5)*(KUKA_LBR_param_.dblLink7CogX*cos(q7) - KUKA_LBR_param_.dblLink7CogY*sin(q7))) + cos(q4)*cos(q5)*sin(q3)*(KUKA_LBR_param_.dblLink7CogZ*cos(q6) + sin(q6)*(KUKA_LBR_param_.dblLink7CogX*cos(q7) - KUKA_LBR_param_.dblLink7CogY*sin(q7))))) + cos(q1)*(sin(q2)*(cos(q4)*(KUKA_LBR_param_.dblLink7CogX*cos(q6)*cos(q7) - KUKA_LBR_param_.dblLink7CogZ*sin(q6) - KUKA_LBR_param_.dblLink7CogY*cos(q6)*sin(q7)) + cos(q5)*sin(q4)*(KUKA_LBR_param_.dblLink7CogZ*cos(q6) + KUKA_LBR_param_.dblLink7CogX*cos(q7)*sin(q6) - KUKA_LBR_param_.dblLink7CogY*sin(q6)*sin(q7))) + cos(q2)*(-(sin(q3)*sin(q5)*(KUKA_LBR_param_.dblLink7CogZ*cos(q6) + sin(q6)*(KUKA_LBR_param_.dblLink7CogX*cos(q7) - KUKA_LBR_param_.dblLink7CogY*sin(q7)))) + cos(q3)*(sin(q4)*(-(KUKA_LBR_param_.dblLink7CogX*cos(q6)*cos(q7)) + KUKA_LBR_param_.dblLink7CogZ*sin(q6) + KUKA_LBR_param_.dblLink7CogY*cos(q6)*sin(q7)) + cos(q4)*cos(q5)*(KUKA_LBR_param_.dblLink7CogZ*cos(q6) + KUKA_LBR_param_.dblLink7CogX*cos(q7)*sin(q6) - KUKA_LBR_param_.dblLink7CogY*sin(q6)*sin(q7))))))*(sin(q1)*(cos(q3)*(-(cos(q6)*sin(q5)*(KUKA_LBR_param_.dblLink7CogY*cos(q7) + KUKA_LBR_param_.dblLink7CogX*sin(q7))) + cos(q5)*(KUKA_LBR_param_.dblLink7CogX*cos(q7) - KUKA_LBR_param_.dblLink7CogY*sin(q7))) - sin(q3)*(sin(q4)*sin(q6)*(KUKA_LBR_param_.dblLink7CogY*cos(q7) + KUKA_LBR_param_.dblLink7CogX*sin(q7)) + cos(q4)*(cos(q5)*cos(q6)*(KUKA_LBR_param_.dblLink7CogY*cos(q7) + KUKA_LBR_param_.dblLink7CogX*sin(q7)) + sin(q5)*(KUKA_LBR_param_.dblLink7CogX*cos(q7) - KUKA_LBR_param_.dblLink7CogY*sin(q7))))) + cos(q1)*(sin(q2)*(cos(q7)*(KUKA_LBR_param_.dblLink7CogX*sin(q4)*sin(q5) - KUKA_LBR_param_.dblLink7CogY*cos(q4)*sin(q6)) - (KUKA_LBR_param_.dblLink7CogY*sin(q4)*sin(q5) + KUKA_LBR_param_.dblLink7CogX*cos(q4)*sin(q6))*sin(q7) + cos(q5)*cos(q6)*sin(q4)*(KUKA_LBR_param_.dblLink7CogY*cos(q7) + KUKA_LBR_param_.dblLink7CogX*sin(q7))) + cos(q2)*(sin(q3)*(-(cos(q6)*sin(q5)*(KUKA_LBR_param_.dblLink7CogY*cos(q7) + KUKA_LBR_param_.dblLink7CogX*sin(q7))) + cos(q5)*(KUKA_LBR_param_.dblLink7CogX*cos(q7) - KUKA_LBR_param_.dblLink7CogY*sin(q7))) + cos(q3)*(sin(q4)*sin(q6)*(KUKA_LBR_param_.dblLink7CogY*cos(q7) + KUKA_LBR_param_.dblLink7CogX*sin(q7)) + cos(q4)*(cos(q5)*cos(q6)*(KUKA_LBR_param_.dblLink7CogY*cos(q7) + KUKA_LBR_param_.dblLink7CogX*sin(q7)) + sin(q5)*(KUKA_LBR_param_.dblLink7CogX*cos(q7) - KUKA_LBR_param_.dblLink7CogY*sin(q7))))))) + KUKA_LBR_param_.dblLink7Mass*(KUKA_LBR_param_.dblLink7CogZ*cos(q5)*cos(q6)*sin(q1)*sin(q2)*sin(q4) - KUKA_LBR_param_.dblLink7CogX*cos(q1)*cos(q6)*cos(q7)*sin(q3)*sin(q4) + KUKA_LBR_param_.dblLink7CogZ*cos(q1)*cos(q3)*cos(q6)*sin(q5) + KUKA_LBR_param_.dblLink7CogX*cos(q5)*cos(q7)*sin(q1)*sin(q2)*sin(q4)*sin(q6) + KUKA_LBR_param_.dblLink7CogZ*cos(q1)*sin(q3)*sin(q4)*sin(q6) + KUKA_LBR_param_.dblLink7CogX*cos(q1)*cos(q3)*cos(q7)*sin(q5)*sin(q6) + KUKA_LBR_param_.dblLink7CogY*cos(q1)*cos(q6)*sin(q3)*sin(q4)*sin(q7) - KUKA_LBR_param_.dblLink7CogY*cos(q5)*sin(q1)*sin(q2)*sin(q4)*sin(q6)*sin(q7) - KUKA_LBR_param_.dblLink7CogY*cos(q1)*cos(q3)*sin(q5)*sin(q6)*sin(q7) + cos(q4)*(cos(q6)*(KUKA_LBR_param_.dblLink7CogX*cos(q7)*sin(q1)*sin(q2) + KUKA_LBR_param_.dblLink7CogZ*cos(q1)*cos(q5)*sin(q3) - KUKA_LBR_param_.dblLink7CogY*sin(q1)*sin(q2)*sin(q7)) - sin(q6)*(KUKA_LBR_param_.dblLink7CogZ*sin(q1)*sin(q2) + cos(q1)*cos(q5)*sin(q3)*(-(KUKA_LBR_param_.dblLink7CogX*cos(q7)) + KUKA_LBR_param_.dblLink7CogY*sin(q7)))) + cos(q2)*sin(q1)*(-(sin(q3)*sin(q5)*(KUKA_LBR_param_.dblLink7CogZ*cos(q6) + sin(q6)*(KUKA_LBR_param_.dblLink7CogX*cos(q7) - KUKA_LBR_param_.dblLink7CogY*sin(q7)))) + cos(q3)*(sin(q4)*(-(KUKA_LBR_param_.dblLink7CogX*cos(q6)*cos(q7)) + KUKA_LBR_param_.dblLink7CogZ*sin(q6) + KUKA_LBR_param_.dblLink7CogY*cos(q6)*sin(q7)) + cos(q4)*cos(q5)*(KUKA_LBR_param_.dblLink7CogZ*cos(q6) + KUKA_LBR_param_.dblLink7CogX*cos(q7)*sin(q6) - KUKA_LBR_param_.dblLink7CogY*sin(q6)*sin(q7)))))*(cos(q1)*(cos(q3)*(cos(q6)*sin(q5)*(KUKA_LBR_param_.dblLink7CogY*cos(q7) + KUKA_LBR_param_.dblLink7CogX*sin(q7)) + cos(q5)*(-(KUKA_LBR_param_.dblLink7CogX*cos(q7)) + KUKA_LBR_param_.dblLink7CogY*sin(q7))) + sin(q3)*(sin(q4)*sin(q6)*(KUKA_LBR_param_.dblLink7CogY*cos(q7) + KUKA_LBR_param_.dblLink7CogX*sin(q7)) + cos(q4)*(cos(q5)*cos(q6)*(KUKA_LBR_param_.dblLink7CogY*cos(q7) + KUKA_LBR_param_.dblLink7CogX*sin(q7)) + sin(q5)*(KUKA_LBR_param_.dblLink7CogX*cos(q7) - KUKA_LBR_param_.dblLink7CogY*sin(q7))))) + sin(q1)*(sin(q2)*(cos(q7)*(KUKA_LBR_param_.dblLink7CogX*sin(q4)*sin(q5) - KUKA_LBR_param_.dblLink7CogY*cos(q4)*sin(q6)) - (KUKA_LBR_param_.dblLink7CogY*sin(q4)*sin(q5) + KUKA_LBR_param_.dblLink7CogX*cos(q4)*sin(q6))*sin(q7) + cos(q5)*cos(q6)*sin(q4)*(KUKA_LBR_param_.dblLink7CogY*cos(q7) + KUKA_LBR_param_.dblLink7CogX*sin(q7))) + cos(q2)*(sin(q3)*(-(cos(q6)*sin(q5)*(KUKA_LBR_param_.dblLink7CogY*cos(q7) + KUKA_LBR_param_.dblLink7CogX*sin(q7))) + cos(q5)*(KUKA_LBR_param_.dblLink7CogX*cos(q7) - KUKA_LBR_param_.dblLink7CogY*sin(q7))) + cos(q3)*(sin(q4)*sin(q6)*(KUKA_LBR_param_.dblLink7CogY*cos(q7) + KUKA_LBR_param_.dblLink7CogX*sin(q7)) + cos(q4)*(cos(q5)*cos(q6)*(KUKA_LBR_param_.dblLink7CogY*cos(q7) + KUKA_LBR_param_.dblLink7CogX*sin(q7)) + sin(q5)*(KUKA_LBR_param_.dblLink7CogX*cos(q7) - KUKA_LBR_param_.dblLink7CogY*sin(q7)))))));
dblMassInertFullRow7Col1 = KUKA_LBR_param_.dblLink7InertXZ*(cos(q6)*(sin(q1)*sin(q3)*sin(q4) + cos(q1)*(cos(q4)*sin(q2) - cos(q2)*cos(q3)*sin(q4))) - (cos(q5)*(cos(q4)*sin(q1)*sin(q3) - cos(q1)*(cos(q2)*cos(q3)*cos(q4) + sin(q2)*sin(q4))) + (cos(q3)*sin(q1) + cos(q1)*cos(q2)*sin(q3))*sin(q5))*sin(q6)) + KUKA_LBR_param_.dblLink7InertYZ*(cos(q6)*(cos(q4)*sin(q1)*sin(q2) - (cos(q2)*cos(q3)*sin(q1) + cos(q1)*sin(q3))*sin(q4)) + (cos(q5)*sin(q1)*sin(q2)*sin(q4) + cos(q1)*(cos(q4)*cos(q5)*sin(q3) + cos(q3)*sin(q5)) + cos(q2)*sin(q1)*(cos(q3)*cos(q4)*cos(q5) - sin(q3)*sin(q5)))*sin(q6)) + KUKA_LBR_param_.dblLink7InertZZ*(cos(q2)*(cos(q4)*cos(q6) + cos(q5)*sin(q4)*sin(q6)) + sin(q2)*(sin(q3)*sin(q5)*sin(q6) + cos(q3)*(cos(q6)*sin(q4) - cos(q4)*cos(q5)*sin(q6)))) - KUKA_LBR_param_.dblLink7Mass*(sin(q1)*(cos(q3)*(cos(q6)*sin(q5)*(KUKA_LBR_param_.dblLink7CogY*cos(q7) + KUKA_LBR_param_.dblLink7CogX*sin(q7)) + cos(q5)*(-(KUKA_LBR_param_.dblLink7CogX*cos(q7)) + KUKA_LBR_param_.dblLink7CogY*sin(q7))) + sin(q3)*(sin(q4)*sin(q6)*(KUKA_LBR_param_.dblLink7CogY*cos(q7) + KUKA_LBR_param_.dblLink7CogX*sin(q7)) + cos(q4)*(cos(q5)*cos(q6)*(KUKA_LBR_param_.dblLink7CogY*cos(q7) + KUKA_LBR_param_.dblLink7CogX*sin(q7)) + sin(q5)*(KUKA_LBR_param_.dblLink7CogX*cos(q7) - KUKA_LBR_param_.dblLink7CogY*sin(q7))))) - cos(q1)*(sin(q2)*(cos(q7)*(KUKA_LBR_param_.dblLink7CogX*sin(q4)*sin(q5) - KUKA_LBR_param_.dblLink7CogY*cos(q4)*sin(q6)) - (KUKA_LBR_param_.dblLink7CogY*sin(q4)*sin(q5) + KUKA_LBR_param_.dblLink7CogX*cos(q4)*sin(q6))*sin(q7) + cos(q5)*cos(q6)*sin(q4)*(KUKA_LBR_param_.dblLink7CogY*cos(q7) + KUKA_LBR_param_.dblLink7CogX*sin(q7))) + cos(q2)*(sin(q3)*(-(cos(q6)*sin(q5)*(KUKA_LBR_param_.dblLink7CogY*cos(q7) + KUKA_LBR_param_.dblLink7CogX*sin(q7))) + cos(q5)*(KUKA_LBR_param_.dblLink7CogX*cos(q7) - KUKA_LBR_param_.dblLink7CogY*sin(q7))) + cos(q3)*(sin(q4)*sin(q6)*(KUKA_LBR_param_.dblLink7CogY*cos(q7) + KUKA_LBR_param_.dblLink7CogX*sin(q7)) + cos(q4)*(cos(q5)*cos(q6)*(KUKA_LBR_param_.dblLink7CogY*cos(q7) + KUKA_LBR_param_.dblLink7CogX*sin(q7)) + sin(q5)*(KUKA_LBR_param_.dblLink7CogX*cos(q7) - KUKA_LBR_param_.dblLink7CogY*sin(q7)))))))*(cos(q1)*(cos(q3)*(cos(q5)*(KUKA_LBR_param_.dblLink7CogY*cos(q7) + KUKA_LBR_param_.dblLink7CogX*sin(q7)) + sin(q5)*(KUKA_LBR_param_.dblLink7CogX*cos(q6)*cos(q7) - KUKA_LBR_param_.dblLink7CogZ*sin(q6) - KUKA_LBR_param_.dblLink7CogY*cos(q6)*sin(q7))) + sin(q3)*(sin(q4)*(KUKA_LBR_param_.dblLink45Len + KUKA_LBR_param_.dblLink7CogZ*cos(q6) + KUKA_LBR_param_.dblLink7CogX*cos(q7)*sin(q6) - KUKA_LBR_param_.dblLink7CogY*sin(q6)*sin(q7)) - cos(q4)*(sin(q5)*(KUKA_LBR_param_.dblLink7CogY*cos(q7) + KUKA_LBR_param_.dblLink7CogX*sin(q7)) + cos(q5)*(-(KUKA_LBR_param_.dblLink7CogX*cos(q6)*cos(q7)) + KUKA_LBR_param_.dblLink7CogZ*sin(q6) + KUKA_LBR_param_.dblLink7CogY*cos(q6)*sin(q7))))) + sin(q1)*(-(sin(q2)*(KUKA_LBR_param_.dblLink23Len + KUKA_LBR_param_.dblLink7CogY*cos(q7)*sin(q4)*sin(q5) + KUKA_LBR_param_.dblLink7CogX*sin(q4)*sin(q5)*sin(q7) + cos(q5)*sin(q4)*(-(KUKA_LBR_param_.dblLink7CogX*cos(q6)*cos(q7)) + KUKA_LBR_param_.dblLink7CogZ*sin(q6) + KUKA_LBR_param_.dblLink7CogY*cos(q6)*sin(q7)) + cos(q4)*(KUKA_LBR_param_.dblLink45Len + KUKA_LBR_param_.dblLink7CogZ*cos(q6) + KUKA_LBR_param_.dblLink7CogX*cos(q7)*sin(q6) - KUKA_LBR_param_.dblLink7CogY*sin(q6)*sin(q7)))) + cos(q2)*(-(sin(q3)*(cos(q5)*(KUKA_LBR_param_.dblLink7CogY*cos(q7) + KUKA_LBR_param_.dblLink7CogX*sin(q7)) + sin(q5)*(KUKA_LBR_param_.dblLink7CogX*cos(q6)*cos(q7) - KUKA_LBR_param_.dblLink7CogZ*sin(q6) - KUKA_LBR_param_.dblLink7CogY*cos(q6)*sin(q7)))) + cos(q3)*(sin(q4)*(KUKA_LBR_param_.dblLink45Len + KUKA_LBR_param_.dblLink7CogZ*cos(q6) + KUKA_LBR_param_.dblLink7CogX*cos(q7)*sin(q6) - KUKA_LBR_param_.dblLink7CogY*sin(q6)*sin(q7)) - cos(q4)*(sin(q5)*(KUKA_LBR_param_.dblLink7CogY*cos(q7) + KUKA_LBR_param_.dblLink7CogX*sin(q7)) + cos(q5)*(-(KUKA_LBR_param_.dblLink7CogX*cos(q6)*cos(q7)) + KUKA_LBR_param_.dblLink7CogZ*sin(q6) + KUKA_LBR_param_.dblLink7CogY*cos(q6)*sin(q7))))))) + KUKA_LBR_param_.dblLink7Mass*(cos(q1)*(cos(q3)*(cos(q6)*sin(q5)*(KUKA_LBR_param_.dblLink7CogY*cos(q7) + KUKA_LBR_param_.dblLink7CogX*sin(q7)) + cos(q5)*(-(KUKA_LBR_param_.dblLink7CogX*cos(q7)) + KUKA_LBR_param_.dblLink7CogY*sin(q7))) + sin(q3)*(sin(q4)*sin(q6)*(KUKA_LBR_param_.dblLink7CogY*cos(q7) + KUKA_LBR_param_.dblLink7CogX*sin(q7)) + cos(q4)*(cos(q5)*cos(q6)*(KUKA_LBR_param_.dblLink7CogY*cos(q7) + KUKA_LBR_param_.dblLink7CogX*sin(q7)) + sin(q5)*(KUKA_LBR_param_.dblLink7CogX*cos(q7) - KUKA_LBR_param_.dblLink7CogY*sin(q7))))) + sin(q1)*(sin(q2)*(cos(q7)*(KUKA_LBR_param_.dblLink7CogX*sin(q4)*sin(q5) - KUKA_LBR_param_.dblLink7CogY*cos(q4)*sin(q6)) - (KUKA_LBR_param_.dblLink7CogY*sin(q4)*sin(q5) + KUKA_LBR_param_.dblLink7CogX*cos(q4)*sin(q6))*sin(q7) + cos(q5)*cos(q6)*sin(q4)*(KUKA_LBR_param_.dblLink7CogY*cos(q7) + KUKA_LBR_param_.dblLink7CogX*sin(q7))) + cos(q2)*(sin(q3)*(-(cos(q6)*sin(q5)*(KUKA_LBR_param_.dblLink7CogY*cos(q7) + KUKA_LBR_param_.dblLink7CogX*sin(q7))) + cos(q5)*(KUKA_LBR_param_.dblLink7CogX*cos(q7) - KUKA_LBR_param_.dblLink7CogY*sin(q7))) + cos(q3)*(sin(q4)*sin(q6)*(KUKA_LBR_param_.dblLink7CogY*cos(q7) + KUKA_LBR_param_.dblLink7CogX*sin(q7)) + cos(q4)*(cos(q5)*cos(q6)*(KUKA_LBR_param_.dblLink7CogY*cos(q7) + KUKA_LBR_param_.dblLink7CogX*sin(q7)) + sin(q5)*(KUKA_LBR_param_.dblLink7CogX*cos(q7) - KUKA_LBR_param_.dblLink7CogY*sin(q7)))))))*(sin(q1)*(cos(q3)*(cos(q5)*(KUKA_LBR_param_.dblLink7CogY*cos(q7) + KUKA_LBR_param_.dblLink7CogX*sin(q7)) + sin(q5)*(KUKA_LBR_param_.dblLink7CogX*cos(q6)*cos(q7) - KUKA_LBR_param_.dblLink7CogZ*sin(q6) - KUKA_LBR_param_.dblLink7CogY*cos(q6)*sin(q7))) + sin(q3)*(sin(q4)*(KUKA_LBR_param_.dblLink45Len + KUKA_LBR_param_.dblLink7CogZ*cos(q6) + KUKA_LBR_param_.dblLink7CogX*cos(q7)*sin(q6) - KUKA_LBR_param_.dblLink7CogY*sin(q6)*sin(q7)) - cos(q4)*(sin(q5)*(KUKA_LBR_param_.dblLink7CogY*cos(q7) + KUKA_LBR_param_.dblLink7CogX*sin(q7)) + cos(q5)*(-(KUKA_LBR_param_.dblLink7CogX*cos(q6)*cos(q7)) + KUKA_LBR_param_.dblLink7CogZ*sin(q6) + KUKA_LBR_param_.dblLink7CogY*cos(q6)*sin(q7))))) + cos(q1)*(sin(q2)*(KUKA_LBR_param_.dblLink23Len + KUKA_LBR_param_.dblLink7CogY*cos(q7)*sin(q4)*sin(q5) + KUKA_LBR_param_.dblLink7CogX*sin(q4)*sin(q5)*sin(q7) + cos(q5)*sin(q4)*(-(KUKA_LBR_param_.dblLink7CogX*cos(q6)*cos(q7)) + KUKA_LBR_param_.dblLink7CogZ*sin(q6) + KUKA_LBR_param_.dblLink7CogY*cos(q6)*sin(q7)) + cos(q4)*(KUKA_LBR_param_.dblLink45Len + KUKA_LBR_param_.dblLink7CogZ*cos(q6) + KUKA_LBR_param_.dblLink7CogX*cos(q7)*sin(q6) - KUKA_LBR_param_.dblLink7CogY*sin(q6)*sin(q7))) + cos(q2)*(sin(q3)*(cos(q5)*(KUKA_LBR_param_.dblLink7CogY*cos(q7) + KUKA_LBR_param_.dblLink7CogX*sin(q7)) + sin(q5)*(KUKA_LBR_param_.dblLink7CogX*cos(q6)*cos(q7) - KUKA_LBR_param_.dblLink7CogZ*sin(q6) - KUKA_LBR_param_.dblLink7CogY*cos(q6)*sin(q7))) + cos(q3)*(-(sin(q4)*(KUKA_LBR_param_.dblLink45Len + KUKA_LBR_param_.dblLink7CogZ*cos(q6) + KUKA_LBR_param_.dblLink7CogX*cos(q7)*sin(q6) - KUKA_LBR_param_.dblLink7CogY*sin(q6)*sin(q7))) + cos(q4)*(sin(q5)*(KUKA_LBR_param_.dblLink7CogY*cos(q7) + KUKA_LBR_param_.dblLink7CogX*sin(q7)) + cos(q5)*(-(KUKA_LBR_param_.dblLink7CogX*cos(q6)*cos(q7)) + KUKA_LBR_param_.dblLink7CogZ*sin(q6) + KUKA_LBR_param_.dblLink7CogY*cos(q6)*sin(q7)))))));
dblMassInertFullRow7Col2 = -(sin(q1)*(KUKA_LBR_param_.dblLink7InertXX*(cos(q6)*(sin(q1)*sin(q3)*sin(q4) + cos(q1)*(cos(q4)*sin(q2) - cos(q2)*cos(q3)*sin(q4))) - (cos(q5)*(cos(q4)*sin(q1)*sin(q3) - cos(q1)*(cos(q2)*cos(q3)*cos(q4) + sin(q2)*sin(q4))) + (cos(q3)*sin(q1) + cos(q1)*cos(q2)*sin(q3))*sin(q5))*sin(q6)) + KUKA_LBR_param_.dblLink7InertXY*(cos(q6)*(cos(q4)*sin(q1)*sin(q2) - (cos(q2)*cos(q3)*sin(q1) + cos(q1)*sin(q3))*sin(q4)) + (cos(q5)*sin(q1)*sin(q2)*sin(q4) + cos(q1)*(cos(q4)*cos(q5)*sin(q3) + cos(q3)*sin(q5)) + cos(q2)*sin(q1)*(cos(q3)*cos(q4)*cos(q5) - sin(q3)*sin(q5)))*sin(q6)) + KUKA_LBR_param_.dblLink7InertXZ*(cos(q2)*(cos(q4)*cos(q6) + cos(q5)*sin(q4)*sin(q6)) + sin(q2)*(sin(q3)*sin(q5)*sin(q6) + cos(q3)*(cos(q6)*sin(q4) - cos(q4)*cos(q5)*sin(q6)))))) + cos(q1)*(KUKA_LBR_param_.dblLink7InertXY*(cos(q6)*(sin(q1)*sin(q3)*sin(q4) + cos(q1)*(cos(q4)*sin(q2) - cos(q2)*cos(q3)*sin(q4))) - (cos(q5)*(cos(q4)*sin(q1)*sin(q3) - cos(q1)*(cos(q2)*cos(q3)*cos(q4) + sin(q2)*sin(q4))) + (cos(q3)*sin(q1) + cos(q1)*cos(q2)*sin(q3))*sin(q5))*sin(q6)) + KUKA_LBR_param_.dblLink7InertYY*(cos(q6)*(cos(q4)*sin(q1)*sin(q2) - (cos(q2)*cos(q3)*sin(q1) + cos(q1)*sin(q3))*sin(q4)) + (cos(q5)*sin(q1)*sin(q2)*sin(q4) + cos(q1)*(cos(q4)*cos(q5)*sin(q3) + cos(q3)*sin(q5)) + cos(q2)*sin(q1)*(cos(q3)*cos(q4)*cos(q5) - sin(q3)*sin(q5)))*sin(q6)) + KUKA_LBR_param_.dblLink7InertYZ*(cos(q2)*(cos(q4)*cos(q6) + cos(q5)*sin(q4)*sin(q6)) + sin(q2)*(sin(q3)*sin(q5)*sin(q6) + cos(q3)*(cos(q6)*sin(q4) - cos(q4)*cos(q5)*sin(q6))))) - KUKA_LBR_param_.dblLink7Mass*(-(KUKA_LBR_param_.dblLink7CogY*cos(q6)*cos(q7)*sin(q2)*sin(q3)*sin(q5)) - KUKA_LBR_param_.dblLink7CogX*cos(q2)*cos(q7)*sin(q4)*sin(q5) + KUKA_LBR_param_.dblLink7CogY*cos(q2)*cos(q4)*cos(q7)*sin(q6) - KUKA_LBR_param_.dblLink7CogX*cos(q6)*sin(q2)*sin(q3)*sin(q5)*sin(q7) + KUKA_LBR_param_.dblLink7CogY*cos(q2)*sin(q4)*sin(q5)*sin(q7) + KUKA_LBR_param_.dblLink7CogX*cos(q2)*cos(q4)*sin(q6)*sin(q7) + cos(q5)*(cos(q7)*(KUKA_LBR_param_.dblLink7CogX*sin(q2)*sin(q3) - KUKA_LBR_param_.dblLink7CogY*cos(q2)*cos(q6)*sin(q4)) - (KUKA_LBR_param_.dblLink7CogY*sin(q2)*sin(q3) + KUKA_LBR_param_.dblLink7CogX*cos(q2)*cos(q6)*sin(q4))*sin(q7)) + cos(q3)*sin(q2)*(sin(q4)*sin(q6)*(KUKA_LBR_param_.dblLink7CogY*cos(q7) + KUKA_LBR_param_.dblLink7CogX*sin(q7)) + cos(q4)*(cos(q5)*cos(q6)*(KUKA_LBR_param_.dblLink7CogY*cos(q7) + KUKA_LBR_param_.dblLink7CogX*sin(q7)) + sin(q5)*(KUKA_LBR_param_.dblLink7CogX*cos(q7) - KUKA_LBR_param_.dblLink7CogY*sin(q7)))))*(-(sin(q2)*(KUKA_LBR_param_.dblLink23Len + KUKA_LBR_param_.dblLink7CogY*cos(q7)*sin(q4)*sin(q5) + KUKA_LBR_param_.dblLink7CogX*sin(q4)*sin(q5)*sin(q7) + cos(q5)*sin(q4)*(-(KUKA_LBR_param_.dblLink7CogX*cos(q6)*cos(q7)) + KUKA_LBR_param_.dblLink7CogZ*sin(q6) + KUKA_LBR_param_.dblLink7CogY*cos(q6)*sin(q7)) + cos(q4)*(KUKA_LBR_param_.dblLink45Len + KUKA_LBR_param_.dblLink7CogZ*cos(q6) + KUKA_LBR_param_.dblLink7CogX*cos(q7)*sin(q6) - KUKA_LBR_param_.dblLink7CogY*sin(q6)*sin(q7)))) + cos(q2)*(-(sin(q3)*(cos(q5)*(KUKA_LBR_param_.dblLink7CogY*cos(q7) + KUKA_LBR_param_.dblLink7CogX*sin(q7)) + sin(q5)*(KUKA_LBR_param_.dblLink7CogX*cos(q6)*cos(q7) - KUKA_LBR_param_.dblLink7CogZ*sin(q6) - KUKA_LBR_param_.dblLink7CogY*cos(q6)*sin(q7)))) + cos(q3)*(sin(q4)*(KUKA_LBR_param_.dblLink45Len + KUKA_LBR_param_.dblLink7CogZ*cos(q6) + KUKA_LBR_param_.dblLink7CogX*cos(q7)*sin(q6) - KUKA_LBR_param_.dblLink7CogY*sin(q6)*sin(q7)) - cos(q4)*(sin(q5)*(KUKA_LBR_param_.dblLink7CogY*cos(q7) + KUKA_LBR_param_.dblLink7CogX*sin(q7)) + cos(q5)*(-(KUKA_LBR_param_.dblLink7CogX*cos(q6)*cos(q7)) + KUKA_LBR_param_.dblLink7CogZ*sin(q6) + KUKA_LBR_param_.dblLink7CogY*cos(q6)*sin(q7)))))) + KUKA_LBR_param_.dblLink7Mass*cos(q1)*(cos(q2)*(KUKA_LBR_param_.dblLink23Len + KUKA_LBR_param_.dblLink7CogY*cos(q7)*sin(q4)*sin(q5) + KUKA_LBR_param_.dblLink7CogX*sin(q4)*sin(q5)*sin(q7) + cos(q5)*sin(q4)*(-(KUKA_LBR_param_.dblLink7CogX*cos(q6)*cos(q7)) + KUKA_LBR_param_.dblLink7CogZ*sin(q6) + KUKA_LBR_param_.dblLink7CogY*cos(q6)*sin(q7)) + cos(q4)*(KUKA_LBR_param_.dblLink45Len + KUKA_LBR_param_.dblLink7CogZ*cos(q6) + KUKA_LBR_param_.dblLink7CogX*cos(q7)*sin(q6) - KUKA_LBR_param_.dblLink7CogY*sin(q6)*sin(q7))) + sin(q2)*(-(sin(q3)*(cos(q5)*(KUKA_LBR_param_.dblLink7CogY*cos(q7) + KUKA_LBR_param_.dblLink7CogX*sin(q7)) + sin(q5)*(KUKA_LBR_param_.dblLink7CogX*cos(q6)*cos(q7) - KUKA_LBR_param_.dblLink7CogZ*sin(q6) - KUKA_LBR_param_.dblLink7CogY*cos(q6)*sin(q7)))) + cos(q3)*(sin(q4)*(KUKA_LBR_param_.dblLink45Len + KUKA_LBR_param_.dblLink7CogZ*cos(q6) + KUKA_LBR_param_.dblLink7CogX*cos(q7)*sin(q6) - KUKA_LBR_param_.dblLink7CogY*sin(q6)*sin(q7)) - cos(q4)*(sin(q5)*(KUKA_LBR_param_.dblLink7CogY*cos(q7) + KUKA_LBR_param_.dblLink7CogX*sin(q7)) + cos(q5)*(-(KUKA_LBR_param_.dblLink7CogX*cos(q6)*cos(q7)) + KUKA_LBR_param_.dblLink7CogZ*sin(q6) + KUKA_LBR_param_.dblLink7CogY*cos(q6)*sin(q7))))))*(sin(q1)*(cos(q3)*(-(cos(q6)*sin(q5)*(KUKA_LBR_param_.dblLink7CogY*cos(q7) + KUKA_LBR_param_.dblLink7CogX*sin(q7))) + cos(q5)*(KUKA_LBR_param_.dblLink7CogX*cos(q7) - KUKA_LBR_param_.dblLink7CogY*sin(q7))) - sin(q3)*(sin(q4)*sin(q6)*(KUKA_LBR_param_.dblLink7CogY*cos(q7) + KUKA_LBR_param_.dblLink7CogX*sin(q7)) + cos(q4)*(cos(q5)*cos(q6)*(KUKA_LBR_param_.dblLink7CogY*cos(q7) + KUKA_LBR_param_.dblLink7CogX*sin(q7)) + sin(q5)*(KUKA_LBR_param_.dblLink7CogX*cos(q7) - KUKA_LBR_param_.dblLink7CogY*sin(q7))))) + cos(q1)*(sin(q2)*(cos(q7)*(KUKA_LBR_param_.dblLink7CogX*sin(q4)*sin(q5) - KUKA_LBR_param_.dblLink7CogY*cos(q4)*sin(q6)) - (KUKA_LBR_param_.dblLink7CogY*sin(q4)*sin(q5) + KUKA_LBR_param_.dblLink7CogX*cos(q4)*sin(q6))*sin(q7) + cos(q5)*cos(q6)*sin(q4)*(KUKA_LBR_param_.dblLink7CogY*cos(q7) + KUKA_LBR_param_.dblLink7CogX*sin(q7))) + cos(q2)*(sin(q3)*(-(cos(q6)*sin(q5)*(KUKA_LBR_param_.dblLink7CogY*cos(q7) + KUKA_LBR_param_.dblLink7CogX*sin(q7))) + cos(q5)*(KUKA_LBR_param_.dblLink7CogX*cos(q7) - KUKA_LBR_param_.dblLink7CogY*sin(q7))) + cos(q3)*(sin(q4)*sin(q6)*(KUKA_LBR_param_.dblLink7CogY*cos(q7) + KUKA_LBR_param_.dblLink7CogX*sin(q7)) + cos(q4)*(cos(q5)*cos(q6)*(KUKA_LBR_param_.dblLink7CogY*cos(q7) + KUKA_LBR_param_.dblLink7CogX*sin(q7)) + sin(q5)*(KUKA_LBR_param_.dblLink7CogX*cos(q7) - KUKA_LBR_param_.dblLink7CogY*sin(q7))))))) + KUKA_LBR_param_.dblLink7Mass*sin(q1)*(cos(q2)*(KUKA_LBR_param_.dblLink23Len + KUKA_LBR_param_.dblLink7CogY*cos(q7)*sin(q4)*sin(q5) + KUKA_LBR_param_.dblLink7CogX*sin(q4)*sin(q5)*sin(q7) + cos(q5)*sin(q4)*(-(KUKA_LBR_param_.dblLink7CogX*cos(q6)*cos(q7)) + KUKA_LBR_param_.dblLink7CogZ*sin(q6) + KUKA_LBR_param_.dblLink7CogY*cos(q6)*sin(q7)) + cos(q4)*(KUKA_LBR_param_.dblLink45Len + KUKA_LBR_param_.dblLink7CogZ*cos(q6) + KUKA_LBR_param_.dblLink7CogX*cos(q7)*sin(q6) - KUKA_LBR_param_.dblLink7CogY*sin(q6)*sin(q7))) + sin(q2)*(-(sin(q3)*(cos(q5)*(KUKA_LBR_param_.dblLink7CogY*cos(q7) + KUKA_LBR_param_.dblLink7CogX*sin(q7)) + sin(q5)*(KUKA_LBR_param_.dblLink7CogX*cos(q6)*cos(q7) - KUKA_LBR_param_.dblLink7CogZ*sin(q6) - KUKA_LBR_param_.dblLink7CogY*cos(q6)*sin(q7)))) + cos(q3)*(sin(q4)*(KUKA_LBR_param_.dblLink45Len + KUKA_LBR_param_.dblLink7CogZ*cos(q6) + KUKA_LBR_param_.dblLink7CogX*cos(q7)*sin(q6) - KUKA_LBR_param_.dblLink7CogY*sin(q6)*sin(q7)) - cos(q4)*(sin(q5)*(KUKA_LBR_param_.dblLink7CogY*cos(q7) + KUKA_LBR_param_.dblLink7CogX*sin(q7)) + cos(q5)*(-(KUKA_LBR_param_.dblLink7CogX*cos(q6)*cos(q7)) + KUKA_LBR_param_.dblLink7CogZ*sin(q6) + KUKA_LBR_param_.dblLink7CogY*cos(q6)*sin(q7))))))*(cos(q1)*(cos(q3)*(cos(q6)*sin(q5)*(KUKA_LBR_param_.dblLink7CogY*cos(q7) + KUKA_LBR_param_.dblLink7CogX*sin(q7)) + cos(q5)*(-(KUKA_LBR_param_.dblLink7CogX*cos(q7)) + KUKA_LBR_param_.dblLink7CogY*sin(q7))) + sin(q3)*(sin(q4)*sin(q6)*(KUKA_LBR_param_.dblLink7CogY*cos(q7) + KUKA_LBR_param_.dblLink7CogX*sin(q7)) + cos(q4)*(cos(q5)*cos(q6)*(KUKA_LBR_param_.dblLink7CogY*cos(q7) + KUKA_LBR_param_.dblLink7CogX*sin(q7)) + sin(q5)*(KUKA_LBR_param_.dblLink7CogX*cos(q7) - KUKA_LBR_param_.dblLink7CogY*sin(q7))))) + sin(q1)*(sin(q2)*(cos(q7)*(KUKA_LBR_param_.dblLink7CogX*sin(q4)*sin(q5) - KUKA_LBR_param_.dblLink7CogY*cos(q4)*sin(q6)) - (KUKA_LBR_param_.dblLink7CogY*sin(q4)*sin(q5) + KUKA_LBR_param_.dblLink7CogX*cos(q4)*sin(q6))*sin(q7) + cos(q5)*cos(q6)*sin(q4)*(KUKA_LBR_param_.dblLink7CogY*cos(q7) + KUKA_LBR_param_.dblLink7CogX*sin(q7))) + cos(q2)*(sin(q3)*(-(cos(q6)*sin(q5)*(KUKA_LBR_param_.dblLink7CogY*cos(q7) + KUKA_LBR_param_.dblLink7CogX*sin(q7))) + cos(q5)*(KUKA_LBR_param_.dblLink7CogX*cos(q7) - KUKA_LBR_param_.dblLink7CogY*sin(q7))) + cos(q3)*(sin(q4)*sin(q6)*(KUKA_LBR_param_.dblLink7CogY*cos(q7) + KUKA_LBR_param_.dblLink7CogX*sin(q7)) + cos(q4)*(cos(q5)*cos(q6)*(KUKA_LBR_param_.dblLink7CogY*cos(q7) + KUKA_LBR_param_.dblLink7CogX*sin(q7)) + sin(q5)*(KUKA_LBR_param_.dblLink7CogX*cos(q7) - KUKA_LBR_param_.dblLink7CogY*sin(q7)))))));
dblMassInertFullRow7Col3 = cos(q1)*sin(q2)*(KUKA_LBR_param_.dblLink7InertXX*(cos(q6)*(sin(q1)*sin(q3)*sin(q4) + cos(q1)*(cos(q4)*sin(q2) - cos(q2)*cos(q3)*sin(q4))) - (cos(q5)*(cos(q4)*sin(q1)*sin(q3) - cos(q1)*(cos(q2)*cos(q3)*cos(q4) + sin(q2)*sin(q4))) + (cos(q3)*sin(q1) + cos(q1)*cos(q2)*sin(q3))*sin(q5))*sin(q6)) + KUKA_LBR_param_.dblLink7InertXY*(cos(q6)*(cos(q4)*sin(q1)*sin(q2) - (cos(q2)*cos(q3)*sin(q1) + cos(q1)*sin(q3))*sin(q4)) + (cos(q5)*sin(q1)*sin(q2)*sin(q4) + cos(q1)*(cos(q4)*cos(q5)*sin(q3) + cos(q3)*sin(q5)) + cos(q2)*sin(q1)*(cos(q3)*cos(q4)*cos(q5) - sin(q3)*sin(q5)))*sin(q6)) + KUKA_LBR_param_.dblLink7InertXZ*(cos(q2)*(cos(q4)*cos(q6) + cos(q5)*sin(q4)*sin(q6)) + sin(q2)*(sin(q3)*sin(q5)*sin(q6) + cos(q3)*(cos(q6)*sin(q4) - cos(q4)*cos(q5)*sin(q6))))) + sin(q1)*sin(q2)*(KUKA_LBR_param_.dblLink7InertXY*(cos(q6)*(sin(q1)*sin(q3)*sin(q4) + cos(q1)*(cos(q4)*sin(q2) - cos(q2)*cos(q3)*sin(q4))) - (cos(q5)*(cos(q4)*sin(q1)*sin(q3) - cos(q1)*(cos(q2)*cos(q3)*cos(q4) + sin(q2)*sin(q4))) + (cos(q3)*sin(q1) + cos(q1)*cos(q2)*sin(q3))*sin(q5))*sin(q6)) + KUKA_LBR_param_.dblLink7InertYY*(cos(q6)*(cos(q4)*sin(q1)*sin(q2) - (cos(q2)*cos(q3)*sin(q1) + cos(q1)*sin(q3))*sin(q4)) + (cos(q5)*sin(q1)*sin(q2)*sin(q4) + cos(q1)*(cos(q4)*cos(q5)*sin(q3) + cos(q3)*sin(q5)) + cos(q2)*sin(q1)*(cos(q3)*cos(q4)*cos(q5) - sin(q3)*sin(q5)))*sin(q6)) + KUKA_LBR_param_.dblLink7InertYZ*(cos(q2)*(cos(q4)*cos(q6) + cos(q5)*sin(q4)*sin(q6)) + sin(q2)*(sin(q3)*sin(q5)*sin(q6) + cos(q3)*(cos(q6)*sin(q4) - cos(q4)*cos(q5)*sin(q6))))) + cos(q2)*(KUKA_LBR_param_.dblLink7InertXZ*(cos(q6)*(sin(q1)*sin(q3)*sin(q4) + cos(q1)*(cos(q4)*sin(q2) - cos(q2)*cos(q3)*sin(q4))) - (cos(q5)*(cos(q4)*sin(q1)*sin(q3) - cos(q1)*(cos(q2)*cos(q3)*cos(q4) + sin(q2)*sin(q4))) + (cos(q3)*sin(q1) + cos(q1)*cos(q2)*sin(q3))*sin(q5))*sin(q6)) + KUKA_LBR_param_.dblLink7InertYZ*(cos(q6)*(cos(q4)*sin(q1)*sin(q2) - (cos(q2)*cos(q3)*sin(q1) + cos(q1)*sin(q3))*sin(q4)) + (cos(q5)*sin(q1)*sin(q2)*sin(q4) + cos(q1)*(cos(q4)*cos(q5)*sin(q3) + cos(q3)*sin(q5)) + cos(q2)*sin(q1)*(cos(q3)*cos(q4)*cos(q5) - sin(q3)*sin(q5)))*sin(q6)) + KUKA_LBR_param_.dblLink7InertZZ*(cos(q2)*(cos(q4)*cos(q6) + cos(q5)*sin(q4)*sin(q6)) + sin(q2)*(sin(q3)*sin(q5)*sin(q6) + cos(q3)*(cos(q6)*sin(q4) - cos(q4)*cos(q5)*sin(q6))))) + KUKA_LBR_param_.dblLink7Mass*sin(q2)*(-(KUKA_LBR_param_.dblLink7CogY*cos(q6)*cos(q7)*sin(q2)*sin(q3)*sin(q5)) - KUKA_LBR_param_.dblLink7CogX*cos(q2)*cos(q7)*sin(q4)*sin(q5) + KUKA_LBR_param_.dblLink7CogY*cos(q2)*cos(q4)*cos(q7)*sin(q6) - KUKA_LBR_param_.dblLink7CogX*cos(q6)*sin(q2)*sin(q3)*sin(q5)*sin(q7) + KUKA_LBR_param_.dblLink7CogY*cos(q2)*sin(q4)*sin(q5)*sin(q7) + KUKA_LBR_param_.dblLink7CogX*cos(q2)*cos(q4)*sin(q6)*sin(q7) + cos(q5)*(cos(q7)*(KUKA_LBR_param_.dblLink7CogX*sin(q2)*sin(q3) - KUKA_LBR_param_.dblLink7CogY*cos(q2)*cos(q6)*sin(q4)) - (KUKA_LBR_param_.dblLink7CogY*sin(q2)*sin(q3) + KUKA_LBR_param_.dblLink7CogX*cos(q2)*cos(q6)*sin(q4))*sin(q7)) + cos(q3)*sin(q2)*(sin(q4)*sin(q6)*(KUKA_LBR_param_.dblLink7CogY*cos(q7) + KUKA_LBR_param_.dblLink7CogX*sin(q7)) + cos(q4)*(cos(q5)*cos(q6)*(KUKA_LBR_param_.dblLink7CogY*cos(q7) + KUKA_LBR_param_.dblLink7CogX*sin(q7)) + sin(q5)*(KUKA_LBR_param_.dblLink7CogX*cos(q7) - KUKA_LBR_param_.dblLink7CogY*sin(q7)))))*(cos(q3)*(cos(q5)*(KUKA_LBR_param_.dblLink7CogY*cos(q7) + KUKA_LBR_param_.dblLink7CogX*sin(q7)) + sin(q5)*(KUKA_LBR_param_.dblLink7CogX*cos(q6)*cos(q7) - KUKA_LBR_param_.dblLink7CogZ*sin(q6) - KUKA_LBR_param_.dblLink7CogY*cos(q6)*sin(q7))) + sin(q3)*(sin(q4)*(KUKA_LBR_param_.dblLink45Len + KUKA_LBR_param_.dblLink7CogZ*cos(q6) + KUKA_LBR_param_.dblLink7CogX*cos(q7)*sin(q6) - KUKA_LBR_param_.dblLink7CogY*sin(q6)*sin(q7)) - cos(q4)*(sin(q5)*(KUKA_LBR_param_.dblLink7CogY*cos(q7) + KUKA_LBR_param_.dblLink7CogX*sin(q7)) + cos(q5)*(-(KUKA_LBR_param_.dblLink7CogX*cos(q6)*cos(q7)) + KUKA_LBR_param_.dblLink7CogZ*sin(q6) + KUKA_LBR_param_.dblLink7CogY*cos(q6)*sin(q7))))) + KUKA_LBR_param_.dblLink7Mass*(sin(q1)*(-(sin(q3)*(cos(q5)*(KUKA_LBR_param_.dblLink7CogY*cos(q7) + KUKA_LBR_param_.dblLink7CogX*sin(q7)) + sin(q5)*(KUKA_LBR_param_.dblLink7CogX*cos(q6)*cos(q7) - KUKA_LBR_param_.dblLink7CogZ*sin(q6) - KUKA_LBR_param_.dblLink7CogY*cos(q6)*sin(q7)))) + cos(q3)*(sin(q4)*(KUKA_LBR_param_.dblLink45Len + KUKA_LBR_param_.dblLink7CogZ*cos(q6) + KUKA_LBR_param_.dblLink7CogX*cos(q7)*sin(q6) - KUKA_LBR_param_.dblLink7CogY*sin(q6)*sin(q7)) - cos(q4)*(sin(q5)*(KUKA_LBR_param_.dblLink7CogY*cos(q7) + KUKA_LBR_param_.dblLink7CogX*sin(q7)) + cos(q5)*(-(KUKA_LBR_param_.dblLink7CogX*cos(q6)*cos(q7)) + KUKA_LBR_param_.dblLink7CogZ*sin(q6) + KUKA_LBR_param_.dblLink7CogY*cos(q6)*sin(q7))))) + cos(q1)*cos(q2)*(cos(q3)*(cos(q5)*(KUKA_LBR_param_.dblLink7CogY*cos(q7) + KUKA_LBR_param_.dblLink7CogX*sin(q7)) + sin(q5)*(KUKA_LBR_param_.dblLink7CogX*cos(q6)*cos(q7) - KUKA_LBR_param_.dblLink7CogZ*sin(q6) - KUKA_LBR_param_.dblLink7CogY*cos(q6)*sin(q7))) + sin(q3)*(sin(q4)*(KUKA_LBR_param_.dblLink45Len + KUKA_LBR_param_.dblLink7CogZ*cos(q6) + KUKA_LBR_param_.dblLink7CogX*cos(q7)*sin(q6) - KUKA_LBR_param_.dblLink7CogY*sin(q6)*sin(q7)) - cos(q4)*(sin(q5)*(KUKA_LBR_param_.dblLink7CogY*cos(q7) + KUKA_LBR_param_.dblLink7CogX*sin(q7)) + cos(q5)*(-(KUKA_LBR_param_.dblLink7CogX*cos(q6)*cos(q7)) + KUKA_LBR_param_.dblLink7CogZ*sin(q6) + KUKA_LBR_param_.dblLink7CogY*cos(q6)*sin(q7))))))*(sin(q1)*(cos(q3)*(-(cos(q6)*sin(q5)*(KUKA_LBR_param_.dblLink7CogY*cos(q7) + KUKA_LBR_param_.dblLink7CogX*sin(q7))) + cos(q5)*(KUKA_LBR_param_.dblLink7CogX*cos(q7) - KUKA_LBR_param_.dblLink7CogY*sin(q7))) - sin(q3)*(sin(q4)*sin(q6)*(KUKA_LBR_param_.dblLink7CogY*cos(q7) + KUKA_LBR_param_.dblLink7CogX*sin(q7)) + cos(q4)*(cos(q5)*cos(q6)*(KUKA_LBR_param_.dblLink7CogY*cos(q7) + KUKA_LBR_param_.dblLink7CogX*sin(q7)) + sin(q5)*(KUKA_LBR_param_.dblLink7CogX*cos(q7) - KUKA_LBR_param_.dblLink7CogY*sin(q7))))) + cos(q1)*(sin(q2)*(cos(q7)*(KUKA_LBR_param_.dblLink7CogX*sin(q4)*sin(q5) - KUKA_LBR_param_.dblLink7CogY*cos(q4)*sin(q6)) - (KUKA_LBR_param_.dblLink7CogY*sin(q4)*sin(q5) + KUKA_LBR_param_.dblLink7CogX*cos(q4)*sin(q6))*sin(q7) + cos(q5)*cos(q6)*sin(q4)*(KUKA_LBR_param_.dblLink7CogY*cos(q7) + KUKA_LBR_param_.dblLink7CogX*sin(q7))) + cos(q2)*(sin(q3)*(-(cos(q6)*sin(q5)*(KUKA_LBR_param_.dblLink7CogY*cos(q7) + KUKA_LBR_param_.dblLink7CogX*sin(q7))) + cos(q5)*(KUKA_LBR_param_.dblLink7CogX*cos(q7) - KUKA_LBR_param_.dblLink7CogY*sin(q7))) + cos(q3)*(sin(q4)*sin(q6)*(KUKA_LBR_param_.dblLink7CogY*cos(q7) + KUKA_LBR_param_.dblLink7CogX*sin(q7)) + cos(q4)*(cos(q5)*cos(q6)*(KUKA_LBR_param_.dblLink7CogY*cos(q7) + KUKA_LBR_param_.dblLink7CogX*sin(q7)) + sin(q5)*(KUKA_LBR_param_.dblLink7CogX*cos(q7) - KUKA_LBR_param_.dblLink7CogY*sin(q7))))))) + KUKA_LBR_param_.dblLink7Mass*(cos(q2)*sin(q1)*(cos(q3)*(cos(q5)*(KUKA_LBR_param_.dblLink7CogY*cos(q7) + KUKA_LBR_param_.dblLink7CogX*sin(q7)) + sin(q5)*(KUKA_LBR_param_.dblLink7CogX*cos(q6)*cos(q7) - KUKA_LBR_param_.dblLink7CogZ*sin(q6) - KUKA_LBR_param_.dblLink7CogY*cos(q6)*sin(q7))) + sin(q3)*(sin(q4)*(KUKA_LBR_param_.dblLink45Len + KUKA_LBR_param_.dblLink7CogZ*cos(q6) + KUKA_LBR_param_.dblLink7CogX*cos(q7)*sin(q6) - KUKA_LBR_param_.dblLink7CogY*sin(q6)*sin(q7)) - cos(q4)*(sin(q5)*(KUKA_LBR_param_.dblLink7CogY*cos(q7) + KUKA_LBR_param_.dblLink7CogX*sin(q7)) + cos(q5)*(-(KUKA_LBR_param_.dblLink7CogX*cos(q6)*cos(q7)) + KUKA_LBR_param_.dblLink7CogZ*sin(q6) + KUKA_LBR_param_.dblLink7CogY*cos(q6)*sin(q7))))) + cos(q1)*(sin(q3)*(cos(q5)*(KUKA_LBR_param_.dblLink7CogY*cos(q7) + KUKA_LBR_param_.dblLink7CogX*sin(q7)) + sin(q5)*(KUKA_LBR_param_.dblLink7CogX*cos(q6)*cos(q7) - KUKA_LBR_param_.dblLink7CogZ*sin(q6) - KUKA_LBR_param_.dblLink7CogY*cos(q6)*sin(q7))) + cos(q3)*(-(sin(q4)*(KUKA_LBR_param_.dblLink45Len + KUKA_LBR_param_.dblLink7CogZ*cos(q6) + KUKA_LBR_param_.dblLink7CogX*cos(q7)*sin(q6) - KUKA_LBR_param_.dblLink7CogY*sin(q6)*sin(q7))) + cos(q4)*(sin(q5)*(KUKA_LBR_param_.dblLink7CogY*cos(q7) + KUKA_LBR_param_.dblLink7CogX*sin(q7)) + cos(q5)*(-(KUKA_LBR_param_.dblLink7CogX*cos(q6)*cos(q7)) + KUKA_LBR_param_.dblLink7CogZ*sin(q6) + KUKA_LBR_param_.dblLink7CogY*cos(q6)*sin(q7))))))*(cos(q1)*(cos(q3)*(cos(q6)*sin(q5)*(KUKA_LBR_param_.dblLink7CogY*cos(q7) + KUKA_LBR_param_.dblLink7CogX*sin(q7)) + cos(q5)*(-(KUKA_LBR_param_.dblLink7CogX*cos(q7)) + KUKA_LBR_param_.dblLink7CogY*sin(q7))) + sin(q3)*(sin(q4)*sin(q6)*(KUKA_LBR_param_.dblLink7CogY*cos(q7) + KUKA_LBR_param_.dblLink7CogX*sin(q7)) + cos(q4)*(cos(q5)*cos(q6)*(KUKA_LBR_param_.dblLink7CogY*cos(q7) + KUKA_LBR_param_.dblLink7CogX*sin(q7)) + sin(q5)*(KUKA_LBR_param_.dblLink7CogX*cos(q7) - KUKA_LBR_param_.dblLink7CogY*sin(q7))))) + sin(q1)*(sin(q2)*(cos(q7)*(KUKA_LBR_param_.dblLink7CogX*sin(q4)*sin(q5) - KUKA_LBR_param_.dblLink7CogY*cos(q4)*sin(q6)) - (KUKA_LBR_param_.dblLink7CogY*sin(q4)*sin(q5) + KUKA_LBR_param_.dblLink7CogX*cos(q4)*sin(q6))*sin(q7) + cos(q5)*cos(q6)*sin(q4)*(KUKA_LBR_param_.dblLink7CogY*cos(q7) + KUKA_LBR_param_.dblLink7CogX*sin(q7))) + cos(q2)*(sin(q3)*(-(cos(q6)*sin(q5)*(KUKA_LBR_param_.dblLink7CogY*cos(q7) + KUKA_LBR_param_.dblLink7CogX*sin(q7))) + cos(q5)*(KUKA_LBR_param_.dblLink7CogX*cos(q7) - KUKA_LBR_param_.dblLink7CogY*sin(q7))) + cos(q3)*(sin(q4)*sin(q6)*(KUKA_LBR_param_.dblLink7CogY*cos(q7) + KUKA_LBR_param_.dblLink7CogX*sin(q7)) + cos(q4)*(cos(q5)*cos(q6)*(KUKA_LBR_param_.dblLink7CogY*cos(q7) + KUKA_LBR_param_.dblLink7CogX*sin(q7)) + sin(q5)*(KUKA_LBR_param_.dblLink7CogX*cos(q7) - KUKA_LBR_param_.dblLink7CogY*sin(q7)))))));
dblMassInertFullRow7Col4 = (cos(q3)*sin(q1) + cos(q1)*cos(q2)*sin(q3))*(KUKA_LBR_param_.dblLink7InertXX*(cos(q6)*(sin(q1)*sin(q3)*sin(q4) + cos(q1)*(cos(q4)*sin(q2) - cos(q2)*cos(q3)*sin(q4))) - (cos(q5)*(cos(q4)*sin(q1)*sin(q3) - cos(q1)*(cos(q2)*cos(q3)*cos(q4) + sin(q2)*sin(q4))) + (cos(q3)*sin(q1) + cos(q1)*cos(q2)*sin(q3))*sin(q5))*sin(q6)) + KUKA_LBR_param_.dblLink7InertXY*(cos(q6)*(cos(q4)*sin(q1)*sin(q2) - (cos(q2)*cos(q3)*sin(q1) + cos(q1)*sin(q3))*sin(q4)) + (cos(q5)*sin(q1)*sin(q2)*sin(q4) + cos(q1)*(cos(q4)*cos(q5)*sin(q3) + cos(q3)*sin(q5)) + cos(q2)*sin(q1)*(cos(q3)*cos(q4)*cos(q5) - sin(q3)*sin(q5)))*sin(q6)) + KUKA_LBR_param_.dblLink7InertXZ*(cos(q2)*(cos(q4)*cos(q6) + cos(q5)*sin(q4)*sin(q6)) + sin(q2)*(sin(q3)*sin(q5)*sin(q6) + cos(q3)*(cos(q6)*sin(q4) - cos(q4)*cos(q5)*sin(q6))))) + (-(cos(q1)*cos(q3)) + cos(q2)*sin(q1)*sin(q3))*(KUKA_LBR_param_.dblLink7InertXY*(cos(q6)*(sin(q1)*sin(q3)*sin(q4) + cos(q1)*(cos(q4)*sin(q2) - cos(q2)*cos(q3)*sin(q4))) - (cos(q5)*(cos(q4)*sin(q1)*sin(q3) - cos(q1)*(cos(q2)*cos(q3)*cos(q4) + sin(q2)*sin(q4))) + (cos(q3)*sin(q1) + cos(q1)*cos(q2)*sin(q3))*sin(q5))*sin(q6)) + KUKA_LBR_param_.dblLink7InertYY*(cos(q6)*(cos(q4)*sin(q1)*sin(q2) - (cos(q2)*cos(q3)*sin(q1) + cos(q1)*sin(q3))*sin(q4)) + (cos(q5)*sin(q1)*sin(q2)*sin(q4) + cos(q1)*(cos(q4)*cos(q5)*sin(q3) + cos(q3)*sin(q5)) + cos(q2)*sin(q1)*(cos(q3)*cos(q4)*cos(q5) - sin(q3)*sin(q5)))*sin(q6)) + KUKA_LBR_param_.dblLink7InertYZ*(cos(q2)*(cos(q4)*cos(q6) + cos(q5)*sin(q4)*sin(q6)) + sin(q2)*(sin(q3)*sin(q5)*sin(q6) + cos(q3)*(cos(q6)*sin(q4) - cos(q4)*cos(q5)*sin(q6))))) - sin(q2)*sin(q3)*(KUKA_LBR_param_.dblLink7InertXZ*(cos(q6)*(sin(q1)*sin(q3)*sin(q4) + cos(q1)*(cos(q4)*sin(q2) - cos(q2)*cos(q3)*sin(q4))) - (cos(q5)*(cos(q4)*sin(q1)*sin(q3) - cos(q1)*(cos(q2)*cos(q3)*cos(q4) + sin(q2)*sin(q4))) + (cos(q3)*sin(q1) + cos(q1)*cos(q2)*sin(q3))*sin(q5))*sin(q6)) + KUKA_LBR_param_.dblLink7InertYZ*(cos(q6)*(cos(q4)*sin(q1)*sin(q2) - (cos(q2)*cos(q3)*sin(q1) + cos(q1)*sin(q3))*sin(q4)) + (cos(q5)*sin(q1)*sin(q2)*sin(q4) + cos(q1)*(cos(q4)*cos(q5)*sin(q3) + cos(q3)*sin(q5)) + cos(q2)*sin(q1)*(cos(q3)*cos(q4)*cos(q5) - sin(q3)*sin(q5)))*sin(q6)) + KUKA_LBR_param_.dblLink7InertZZ*(cos(q2)*(cos(q4)*cos(q6) + cos(q5)*sin(q4)*sin(q6)) + sin(q2)*(sin(q3)*sin(q5)*sin(q6) + cos(q3)*(cos(q6)*sin(q4) - cos(q4)*cos(q5)*sin(q6))))) + KUKA_LBR_param_.dblLink7Mass*(KUKA_LBR_param_.dblLink7CogY*cos(q6)*cos(q7)*sin(q2)*sin(q3)*sin(q5) + KUKA_LBR_param_.dblLink7CogX*cos(q2)*cos(q7)*sin(q4)*sin(q5) - KUKA_LBR_param_.dblLink7CogY*cos(q2)*cos(q4)*cos(q7)*sin(q6) + KUKA_LBR_param_.dblLink7CogX*cos(q6)*sin(q2)*sin(q3)*sin(q5)*sin(q7) - KUKA_LBR_param_.dblLink7CogY*cos(q2)*sin(q4)*sin(q5)*sin(q7) - KUKA_LBR_param_.dblLink7CogX*cos(q2)*cos(q4)*sin(q6)*sin(q7) + cos(q5)*(-(KUKA_LBR_param_.dblLink7CogX*cos(q7)*sin(q2)*sin(q3)) + KUKA_LBR_param_.dblLink7CogY*cos(q2)*cos(q6)*cos(q7)*sin(q4) + KUKA_LBR_param_.dblLink7CogY*sin(q2)*sin(q3)*sin(q7) + KUKA_LBR_param_.dblLink7CogX*cos(q2)*cos(q6)*sin(q4)*sin(q7)) - cos(q3)*sin(q2)*(sin(q4)*sin(q6)*(KUKA_LBR_param_.dblLink7CogY*cos(q7) + KUKA_LBR_param_.dblLink7CogX*sin(q7)) + cos(q4)*(cos(q5)*cos(q6)*(KUKA_LBR_param_.dblLink7CogY*cos(q7) + KUKA_LBR_param_.dblLink7CogX*sin(q7)) + sin(q5)*(KUKA_LBR_param_.dblLink7CogX*cos(q7) - KUKA_LBR_param_.dblLink7CogY*sin(q7)))))*(cos(q2)*(-(sin(q4)*(KUKA_LBR_param_.dblLink45Len + KUKA_LBR_param_.dblLink7CogZ*cos(q6) + KUKA_LBR_param_.dblLink7CogX*cos(q7)*sin(q6) - KUKA_LBR_param_.dblLink7CogY*sin(q6)*sin(q7))) + cos(q4)*(sin(q5)*(KUKA_LBR_param_.dblLink7CogY*cos(q7) + KUKA_LBR_param_.dblLink7CogX*sin(q7)) + cos(q5)*(-(KUKA_LBR_param_.dblLink7CogX*cos(q6)*cos(q7)) + KUKA_LBR_param_.dblLink7CogZ*sin(q6) + KUKA_LBR_param_.dblLink7CogY*cos(q6)*sin(q7)))) + cos(q3)*sin(q2)*(cos(q4)*(KUKA_LBR_param_.dblLink45Len + KUKA_LBR_param_.dblLink7CogZ*cos(q6) + KUKA_LBR_param_.dblLink7CogX*cos(q7)*sin(q6) - KUKA_LBR_param_.dblLink7CogY*sin(q6)*sin(q7)) + sin(q4)*(sin(q5)*(KUKA_LBR_param_.dblLink7CogY*cos(q7) + KUKA_LBR_param_.dblLink7CogX*sin(q7)) + cos(q5)*(-(KUKA_LBR_param_.dblLink7CogX*cos(q6)*cos(q7)) + KUKA_LBR_param_.dblLink7CogZ*sin(q6) + KUKA_LBR_param_.dblLink7CogY*cos(q6)*sin(q7))))) + KUKA_LBR_param_.dblLink7Mass*(sin(q1)*sin(q3)*(cos(q4)*(KUKA_LBR_param_.dblLink45Len + KUKA_LBR_param_.dblLink7CogZ*cos(q6) + KUKA_LBR_param_.dblLink7CogX*cos(q7)*sin(q6) - KUKA_LBR_param_.dblLink7CogY*sin(q6)*sin(q7)) + sin(q4)*(sin(q5)*(KUKA_LBR_param_.dblLink7CogY*cos(q7) + KUKA_LBR_param_.dblLink7CogX*sin(q7)) + cos(q5)*(-(KUKA_LBR_param_.dblLink7CogX*cos(q6)*cos(q7)) + KUKA_LBR_param_.dblLink7CogZ*sin(q6) + KUKA_LBR_param_.dblLink7CogY*cos(q6)*sin(q7)))) - cos(q1)*(sin(q2)*(sin(q4)*(KUKA_LBR_param_.dblLink45Len + KUKA_LBR_param_.dblLink7CogZ*cos(q6) + KUKA_LBR_param_.dblLink7CogX*cos(q7)*sin(q6) - KUKA_LBR_param_.dblLink7CogY*sin(q6)*sin(q7)) - cos(q4)*(sin(q5)*(KUKA_LBR_param_.dblLink7CogY*cos(q7) + KUKA_LBR_param_.dblLink7CogX*sin(q7)) + cos(q5)*(-(KUKA_LBR_param_.dblLink7CogX*cos(q6)*cos(q7)) + KUKA_LBR_param_.dblLink7CogZ*sin(q6) + KUKA_LBR_param_.dblLink7CogY*cos(q6)*sin(q7)))) + cos(q2)*cos(q3)*(cos(q4)*(KUKA_LBR_param_.dblLink45Len + KUKA_LBR_param_.dblLink7CogZ*cos(q6) + KUKA_LBR_param_.dblLink7CogX*cos(q7)*sin(q6) - KUKA_LBR_param_.dblLink7CogY*sin(q6)*sin(q7)) + sin(q4)*(sin(q5)*(KUKA_LBR_param_.dblLink7CogY*cos(q7) + KUKA_LBR_param_.dblLink7CogX*sin(q7)) + cos(q5)*(-(KUKA_LBR_param_.dblLink7CogX*cos(q6)*cos(q7)) + KUKA_LBR_param_.dblLink7CogZ*sin(q6) + KUKA_LBR_param_.dblLink7CogY*cos(q6)*sin(q7))))))*(sin(q1)*(cos(q3)*(-(cos(q6)*sin(q5)*(KUKA_LBR_param_.dblLink7CogY*cos(q7) + KUKA_LBR_param_.dblLink7CogX*sin(q7))) + cos(q5)*(KUKA_LBR_param_.dblLink7CogX*cos(q7) - KUKA_LBR_param_.dblLink7CogY*sin(q7))) - sin(q3)*(sin(q4)*sin(q6)*(KUKA_LBR_param_.dblLink7CogY*cos(q7) + KUKA_LBR_param_.dblLink7CogX*sin(q7)) + cos(q4)*(cos(q5)*cos(q6)*(KUKA_LBR_param_.dblLink7CogY*cos(q7) + KUKA_LBR_param_.dblLink7CogX*sin(q7)) + sin(q5)*(KUKA_LBR_param_.dblLink7CogX*cos(q7) - KUKA_LBR_param_.dblLink7CogY*sin(q7))))) + cos(q1)*(sin(q2)*(cos(q7)*(KUKA_LBR_param_.dblLink7CogX*sin(q4)*sin(q5) - KUKA_LBR_param_.dblLink7CogY*cos(q4)*sin(q6)) - (KUKA_LBR_param_.dblLink7CogY*sin(q4)*sin(q5) + KUKA_LBR_param_.dblLink7CogX*cos(q4)*sin(q6))*sin(q7) + cos(q5)*cos(q6)*sin(q4)*(KUKA_LBR_param_.dblLink7CogY*cos(q7) + KUKA_LBR_param_.dblLink7CogX*sin(q7))) + cos(q2)*(sin(q3)*(-(cos(q6)*sin(q5)*(KUKA_LBR_param_.dblLink7CogY*cos(q7) + KUKA_LBR_param_.dblLink7CogX*sin(q7))) + cos(q5)*(KUKA_LBR_param_.dblLink7CogX*cos(q7) - KUKA_LBR_param_.dblLink7CogY*sin(q7))) + cos(q3)*(sin(q4)*sin(q6)*(KUKA_LBR_param_.dblLink7CogY*cos(q7) + KUKA_LBR_param_.dblLink7CogX*sin(q7)) + cos(q4)*(cos(q5)*cos(q6)*(KUKA_LBR_param_.dblLink7CogY*cos(q7) + KUKA_LBR_param_.dblLink7CogX*sin(q7)) + sin(q5)*(KUKA_LBR_param_.dblLink7CogX*cos(q7) - KUKA_LBR_param_.dblLink7CogY*sin(q7))))))) + KUKA_LBR_param_.dblLink7Mass*(cos(q4)*(sin(q1)*sin(q2)*sin(q5)*(KUKA_LBR_param_.dblLink7CogY*cos(q7) + KUKA_LBR_param_.dblLink7CogX*sin(q7)) - cos(q1)*sin(q3)*(KUKA_LBR_param_.dblLink45Len + KUKA_LBR_param_.dblLink7CogZ*cos(q6) + KUKA_LBR_param_.dblLink7CogX*cos(q7)*sin(q6) - KUKA_LBR_param_.dblLink7CogY*sin(q6)*sin(q7)) + cos(q5)*sin(q1)*sin(q2)*(KUKA_LBR_param_.dblLink7CogZ*sin(q6) + cos(q6)*(-(KUKA_LBR_param_.dblLink7CogX*cos(q7)) + KUKA_LBR_param_.dblLink7CogY*sin(q7)))) - sin(q4)*(sin(q1)*sin(q2)*(KUKA_LBR_param_.dblLink45Len + KUKA_LBR_param_.dblLink7CogZ*cos(q6) + KUKA_LBR_param_.dblLink7CogX*cos(q7)*sin(q6) - KUKA_LBR_param_.dblLink7CogY*sin(q6)*sin(q7)) + cos(q1)*sin(q3)*(sin(q5)*(KUKA_LBR_param_.dblLink7CogY*cos(q7) + KUKA_LBR_param_.dblLink7CogX*sin(q7)) + cos(q5)*(-(KUKA_LBR_param_.dblLink7CogX*cos(q6)*cos(q7)) + KUKA_LBR_param_.dblLink7CogZ*sin(q6) + KUKA_LBR_param_.dblLink7CogY*cos(q6)*sin(q7)))) - cos(q2)*cos(q3)*sin(q1)*(cos(q4)*(KUKA_LBR_param_.dblLink45Len + KUKA_LBR_param_.dblLink7CogZ*cos(q6) + KUKA_LBR_param_.dblLink7CogX*cos(q7)*sin(q6) - KUKA_LBR_param_.dblLink7CogY*sin(q6)*sin(q7)) + sin(q4)*(sin(q5)*(KUKA_LBR_param_.dblLink7CogY*cos(q7) + KUKA_LBR_param_.dblLink7CogX*sin(q7)) + cos(q5)*(-(KUKA_LBR_param_.dblLink7CogX*cos(q6)*cos(q7)) + KUKA_LBR_param_.dblLink7CogZ*sin(q6) + KUKA_LBR_param_.dblLink7CogY*cos(q6)*sin(q7)))))*(cos(q1)*(cos(q3)*(cos(q6)*sin(q5)*(KUKA_LBR_param_.dblLink7CogY*cos(q7) + KUKA_LBR_param_.dblLink7CogX*sin(q7)) + cos(q5)*(-(KUKA_LBR_param_.dblLink7CogX*cos(q7)) + KUKA_LBR_param_.dblLink7CogY*sin(q7))) + sin(q3)*(sin(q4)*sin(q6)*(KUKA_LBR_param_.dblLink7CogY*cos(q7) + KUKA_LBR_param_.dblLink7CogX*sin(q7)) + cos(q4)*(cos(q5)*cos(q6)*(KUKA_LBR_param_.dblLink7CogY*cos(q7) + KUKA_LBR_param_.dblLink7CogX*sin(q7)) + sin(q5)*(KUKA_LBR_param_.dblLink7CogX*cos(q7) - KUKA_LBR_param_.dblLink7CogY*sin(q7))))) + sin(q1)*(sin(q2)*(cos(q7)*(KUKA_LBR_param_.dblLink7CogX*sin(q4)*sin(q5) - KUKA_LBR_param_.dblLink7CogY*cos(q4)*sin(q6)) - (KUKA_LBR_param_.dblLink7CogY*sin(q4)*sin(q5) + KUKA_LBR_param_.dblLink7CogX*cos(q4)*sin(q6))*sin(q7) + cos(q5)*cos(q6)*sin(q4)*(KUKA_LBR_param_.dblLink7CogY*cos(q7) + KUKA_LBR_param_.dblLink7CogX*sin(q7))) + cos(q2)*(sin(q3)*(-(cos(q6)*sin(q5)*(KUKA_LBR_param_.dblLink7CogY*cos(q7) + KUKA_LBR_param_.dblLink7CogX*sin(q7))) + cos(q5)*(KUKA_LBR_param_.dblLink7CogX*cos(q7) - KUKA_LBR_param_.dblLink7CogY*sin(q7))) + cos(q3)*(sin(q4)*sin(q6)*(KUKA_LBR_param_.dblLink7CogY*cos(q7) + KUKA_LBR_param_.dblLink7CogX*sin(q7)) + cos(q4)*(cos(q5)*cos(q6)*(KUKA_LBR_param_.dblLink7CogY*cos(q7) + KUKA_LBR_param_.dblLink7CogX*sin(q7)) + sin(q5)*(KUKA_LBR_param_.dblLink7CogX*cos(q7) - KUKA_LBR_param_.dblLink7CogY*sin(q7)))))));
dblMassInertFullRow7Col5 = (sin(q1)*sin(q3)*sin(q4) + cos(q1)*(cos(q4)*sin(q2) - cos(q2)*cos(q3)*sin(q4)))*(KUKA_LBR_param_.dblLink7InertXX*(cos(q6)*(sin(q1)*sin(q3)*sin(q4) + cos(q1)*(cos(q4)*sin(q2) - cos(q2)*cos(q3)*sin(q4))) - (cos(q5)*(cos(q4)*sin(q1)*sin(q3) - cos(q1)*(cos(q2)*cos(q3)*cos(q4) + sin(q2)*sin(q4))) + (cos(q3)*sin(q1) + cos(q1)*cos(q2)*sin(q3))*sin(q5))*sin(q6)) + KUKA_LBR_param_.dblLink7InertXY*(cos(q6)*(cos(q4)*sin(q1)*sin(q2) - (cos(q2)*cos(q3)*sin(q1) + cos(q1)*sin(q3))*sin(q4)) + (cos(q5)*sin(q1)*sin(q2)*sin(q4) + cos(q1)*(cos(q4)*cos(q5)*sin(q3) + cos(q3)*sin(q5)) + cos(q2)*sin(q1)*(cos(q3)*cos(q4)*cos(q5) - sin(q3)*sin(q5)))*sin(q6)) + KUKA_LBR_param_.dblLink7InertXZ*(cos(q2)*(cos(q4)*cos(q6) + cos(q5)*sin(q4)*sin(q6)) + sin(q2)*(sin(q3)*sin(q5)*sin(q6) + cos(q3)*(cos(q6)*sin(q4) - cos(q4)*cos(q5)*sin(q6))))) + (cos(q4)*sin(q1)*sin(q2) - (cos(q2)*cos(q3)*sin(q1) + cos(q1)*sin(q3))*sin(q4))*(KUKA_LBR_param_.dblLink7InertXY*(cos(q6)*(sin(q1)*sin(q3)*sin(q4) + cos(q1)*(cos(q4)*sin(q2) - cos(q2)*cos(q3)*sin(q4))) - (cos(q5)*(cos(q4)*sin(q1)*sin(q3) - cos(q1)*(cos(q2)*cos(q3)*cos(q4) + sin(q2)*sin(q4))) + (cos(q3)*sin(q1) + cos(q1)*cos(q2)*sin(q3))*sin(q5))*sin(q6)) + KUKA_LBR_param_.dblLink7InertYY*(cos(q6)*(cos(q4)*sin(q1)*sin(q2) - (cos(q2)*cos(q3)*sin(q1) + cos(q1)*sin(q3))*sin(q4)) + (cos(q5)*sin(q1)*sin(q2)*sin(q4) + cos(q1)*(cos(q4)*cos(q5)*sin(q3) + cos(q3)*sin(q5)) + cos(q2)*sin(q1)*(cos(q3)*cos(q4)*cos(q5) - sin(q3)*sin(q5)))*sin(q6)) + KUKA_LBR_param_.dblLink7InertYZ*(cos(q2)*(cos(q4)*cos(q6) + cos(q5)*sin(q4)*sin(q6)) + sin(q2)*(sin(q3)*sin(q5)*sin(q6) + cos(q3)*(cos(q6)*sin(q4) - cos(q4)*cos(q5)*sin(q6))))) + (cos(q2)*cos(q4) + cos(q3)*sin(q2)*sin(q4))*(KUKA_LBR_param_.dblLink7InertXZ*(cos(q6)*(sin(q1)*sin(q3)*sin(q4) + cos(q1)*(cos(q4)*sin(q2) - cos(q2)*cos(q3)*sin(q4))) - (cos(q5)*(cos(q4)*sin(q1)*sin(q3) - cos(q1)*(cos(q2)*cos(q3)*cos(q4) + sin(q2)*sin(q4))) + (cos(q3)*sin(q1) + cos(q1)*cos(q2)*sin(q3))*sin(q5))*sin(q6)) + KUKA_LBR_param_.dblLink7InertYZ*(cos(q6)*(cos(q4)*sin(q1)*sin(q2) - (cos(q2)*cos(q3)*sin(q1) + cos(q1)*sin(q3))*sin(q4)) + (cos(q5)*sin(q1)*sin(q2)*sin(q4) + cos(q1)*(cos(q4)*cos(q5)*sin(q3) + cos(q3)*sin(q5)) + cos(q2)*sin(q1)*(cos(q3)*cos(q4)*cos(q5) - sin(q3)*sin(q5)))*sin(q6)) + KUKA_LBR_param_.dblLink7InertZZ*(cos(q2)*(cos(q4)*cos(q6) + cos(q5)*sin(q4)*sin(q6)) + sin(q2)*(sin(q3)*sin(q5)*sin(q6) + cos(q3)*(cos(q6)*sin(q4) - cos(q4)*cos(q5)*sin(q6))))) - KUKA_LBR_param_.dblLink7Mass*(-(KUKA_LBR_param_.dblLink7CogY*cos(q6)*cos(q7)*sin(q2)*sin(q3)*sin(q5)) - KUKA_LBR_param_.dblLink7CogX*cos(q2)*cos(q7)*sin(q4)*sin(q5) + KUKA_LBR_param_.dblLink7CogY*cos(q2)*cos(q4)*cos(q7)*sin(q6) - KUKA_LBR_param_.dblLink7CogX*cos(q6)*sin(q2)*sin(q3)*sin(q5)*sin(q7) + KUKA_LBR_param_.dblLink7CogY*cos(q2)*sin(q4)*sin(q5)*sin(q7) + KUKA_LBR_param_.dblLink7CogX*cos(q2)*cos(q4)*sin(q6)*sin(q7) + cos(q5)*(cos(q7)*(KUKA_LBR_param_.dblLink7CogX*sin(q2)*sin(q3) - KUKA_LBR_param_.dblLink7CogY*cos(q2)*cos(q6)*sin(q4)) - (KUKA_LBR_param_.dblLink7CogY*sin(q2)*sin(q3) + KUKA_LBR_param_.dblLink7CogX*cos(q2)*cos(q6)*sin(q4))*sin(q7)) + cos(q3)*sin(q2)*(sin(q4)*sin(q6)*(KUKA_LBR_param_.dblLink7CogY*cos(q7) + KUKA_LBR_param_.dblLink7CogX*sin(q7)) + cos(q4)*(cos(q5)*cos(q6)*(KUKA_LBR_param_.dblLink7CogY*cos(q7) + KUKA_LBR_param_.dblLink7CogX*sin(q7)) + sin(q5)*(KUKA_LBR_param_.dblLink7CogX*cos(q7) - KUKA_LBR_param_.dblLink7CogY*sin(q7)))))*(cos(q5)*(KUKA_LBR_param_.dblLink7CogZ*sin(q2)*sin(q3)*sin(q6) + cos(q2)*sin(q4)*(KUKA_LBR_param_.dblLink7CogY*cos(q7) + KUKA_LBR_param_.dblLink7CogX*sin(q7)) - cos(q6)*sin(q2)*sin(q3)*(KUKA_LBR_param_.dblLink7CogX*cos(q7) - KUKA_LBR_param_.dblLink7CogY*sin(q7))) + sin(q5)*(cos(q7)*(KUKA_LBR_param_.dblLink7CogY*sin(q2)*sin(q3) + KUKA_LBR_param_.dblLink7CogX*cos(q2)*cos(q6)*sin(q4)) + KUKA_LBR_param_.dblLink7CogX*sin(q2)*sin(q3)*sin(q7) - cos(q2)*sin(q4)*(KUKA_LBR_param_.dblLink7CogZ*sin(q6) + KUKA_LBR_param_.dblLink7CogY*cos(q6)*sin(q7))) - cos(q3)*cos(q4)*sin(q2)*(cos(q5)*(KUKA_LBR_param_.dblLink7CogY*cos(q7) + KUKA_LBR_param_.dblLink7CogX*sin(q7)) - sin(q5)*(KUKA_LBR_param_.dblLink7CogZ*sin(q6) + cos(q6)*(-(KUKA_LBR_param_.dblLink7CogX*cos(q7)) + KUKA_LBR_param_.dblLink7CogY*sin(q7))))) + KUKA_LBR_param_.dblLink7Mass*(sin(q1)*(-(cos(q4)*sin(q3)*(cos(q5)*(KUKA_LBR_param_.dblLink7CogY*cos(q7) + KUKA_LBR_param_.dblLink7CogX*sin(q7)) + sin(q5)*(KUKA_LBR_param_.dblLink7CogX*cos(q6)*cos(q7) - KUKA_LBR_param_.dblLink7CogZ*sin(q6) - KUKA_LBR_param_.dblLink7CogY*cos(q6)*sin(q7)))) - cos(q3)*(sin(q5)*(KUKA_LBR_param_.dblLink7CogY*cos(q7) + KUKA_LBR_param_.dblLink7CogX*sin(q7)) + cos(q5)*(-(KUKA_LBR_param_.dblLink7CogX*cos(q6)*cos(q7)) + KUKA_LBR_param_.dblLink7CogZ*sin(q6) + KUKA_LBR_param_.dblLink7CogY*cos(q6)*sin(q7)))) + cos(q1)*(sin(q2)*sin(q4)*(cos(q5)*(KUKA_LBR_param_.dblLink7CogY*cos(q7) + KUKA_LBR_param_.dblLink7CogX*sin(q7)) + sin(q5)*(KUKA_LBR_param_.dblLink7CogX*cos(q6)*cos(q7) - KUKA_LBR_param_.dblLink7CogZ*sin(q6) - KUKA_LBR_param_.dblLink7CogY*cos(q6)*sin(q7))) + cos(q2)*(cos(q3)*cos(q4)*(cos(q5)*(KUKA_LBR_param_.dblLink7CogY*cos(q7) + KUKA_LBR_param_.dblLink7CogX*sin(q7)) + sin(q5)*(KUKA_LBR_param_.dblLink7CogX*cos(q6)*cos(q7) - KUKA_LBR_param_.dblLink7CogZ*sin(q6) - KUKA_LBR_param_.dblLink7CogY*cos(q6)*sin(q7))) - sin(q3)*(sin(q5)*(KUKA_LBR_param_.dblLink7CogY*cos(q7) + KUKA_LBR_param_.dblLink7CogX*sin(q7)) + cos(q5)*(-(KUKA_LBR_param_.dblLink7CogX*cos(q6)*cos(q7)) + KUKA_LBR_param_.dblLink7CogZ*sin(q6) + KUKA_LBR_param_.dblLink7CogY*cos(q6)*sin(q7))))))*(sin(q1)*(cos(q3)*(-(cos(q6)*sin(q5)*(KUKA_LBR_param_.dblLink7CogY*cos(q7) + KUKA_LBR_param_.dblLink7CogX*sin(q7))) + cos(q5)*(KUKA_LBR_param_.dblLink7CogX*cos(q7) - KUKA_LBR_param_.dblLink7CogY*sin(q7))) - sin(q3)*(sin(q4)*sin(q6)*(KUKA_LBR_param_.dblLink7CogY*cos(q7) + KUKA_LBR_param_.dblLink7CogX*sin(q7)) + cos(q4)*(cos(q5)*cos(q6)*(KUKA_LBR_param_.dblLink7CogY*cos(q7) + KUKA_LBR_param_.dblLink7CogX*sin(q7)) + sin(q5)*(KUKA_LBR_param_.dblLink7CogX*cos(q7) - KUKA_LBR_param_.dblLink7CogY*sin(q7))))) + cos(q1)*(sin(q2)*(cos(q7)*(KUKA_LBR_param_.dblLink7CogX*sin(q4)*sin(q5) - KUKA_LBR_param_.dblLink7CogY*cos(q4)*sin(q6)) - (KUKA_LBR_param_.dblLink7CogY*sin(q4)*sin(q5) + KUKA_LBR_param_.dblLink7CogX*cos(q4)*sin(q6))*sin(q7) + cos(q5)*cos(q6)*sin(q4)*(KUKA_LBR_param_.dblLink7CogY*cos(q7) + KUKA_LBR_param_.dblLink7CogX*sin(q7))) + cos(q2)*(sin(q3)*(-(cos(q6)*sin(q5)*(KUKA_LBR_param_.dblLink7CogY*cos(q7) + KUKA_LBR_param_.dblLink7CogX*sin(q7))) + cos(q5)*(KUKA_LBR_param_.dblLink7CogX*cos(q7) - KUKA_LBR_param_.dblLink7CogY*sin(q7))) + cos(q3)*(sin(q4)*sin(q6)*(KUKA_LBR_param_.dblLink7CogY*cos(q7) + KUKA_LBR_param_.dblLink7CogX*sin(q7)) + cos(q4)*(cos(q5)*cos(q6)*(KUKA_LBR_param_.dblLink7CogY*cos(q7) + KUKA_LBR_param_.dblLink7CogX*sin(q7)) + sin(q5)*(KUKA_LBR_param_.dblLink7CogX*cos(q7) - KUKA_LBR_param_.dblLink7CogY*sin(q7))))))) + KUKA_LBR_param_.dblLink7Mass*(cos(q1)*(cos(q4)*sin(q3)*(cos(q5)*(KUKA_LBR_param_.dblLink7CogY*cos(q7) + KUKA_LBR_param_.dblLink7CogX*sin(q7)) + sin(q5)*(KUKA_LBR_param_.dblLink7CogX*cos(q6)*cos(q7) - KUKA_LBR_param_.dblLink7CogZ*sin(q6) - KUKA_LBR_param_.dblLink7CogY*cos(q6)*sin(q7))) + cos(q3)*(sin(q5)*(KUKA_LBR_param_.dblLink7CogY*cos(q7) + KUKA_LBR_param_.dblLink7CogX*sin(q7)) + cos(q5)*(-(KUKA_LBR_param_.dblLink7CogX*cos(q6)*cos(q7)) + KUKA_LBR_param_.dblLink7CogZ*sin(q6) + KUKA_LBR_param_.dblLink7CogY*cos(q6)*sin(q7)))) + sin(q1)*(sin(q2)*sin(q4)*(cos(q5)*(KUKA_LBR_param_.dblLink7CogY*cos(q7) + KUKA_LBR_param_.dblLink7CogX*sin(q7)) + sin(q5)*(KUKA_LBR_param_.dblLink7CogX*cos(q6)*cos(q7) - KUKA_LBR_param_.dblLink7CogZ*sin(q6) - KUKA_LBR_param_.dblLink7CogY*cos(q6)*sin(q7))) + cos(q2)*(cos(q3)*cos(q4)*(cos(q5)*(KUKA_LBR_param_.dblLink7CogY*cos(q7) + KUKA_LBR_param_.dblLink7CogX*sin(q7)) + sin(q5)*(KUKA_LBR_param_.dblLink7CogX*cos(q6)*cos(q7) - KUKA_LBR_param_.dblLink7CogZ*sin(q6) - KUKA_LBR_param_.dblLink7CogY*cos(q6)*sin(q7))) - sin(q3)*(sin(q5)*(KUKA_LBR_param_.dblLink7CogY*cos(q7) + KUKA_LBR_param_.dblLink7CogX*sin(q7)) + cos(q5)*(-(KUKA_LBR_param_.dblLink7CogX*cos(q6)*cos(q7)) + KUKA_LBR_param_.dblLink7CogZ*sin(q6) + KUKA_LBR_param_.dblLink7CogY*cos(q6)*sin(q7))))))*(cos(q1)*(cos(q3)*(cos(q6)*sin(q5)*(KUKA_LBR_param_.dblLink7CogY*cos(q7) + KUKA_LBR_param_.dblLink7CogX*sin(q7)) + cos(q5)*(-(KUKA_LBR_param_.dblLink7CogX*cos(q7)) + KUKA_LBR_param_.dblLink7CogY*sin(q7))) + sin(q3)*(sin(q4)*sin(q6)*(KUKA_LBR_param_.dblLink7CogY*cos(q7) + KUKA_LBR_param_.dblLink7CogX*sin(q7)) + cos(q4)*(cos(q5)*cos(q6)*(KUKA_LBR_param_.dblLink7CogY*cos(q7) + KUKA_LBR_param_.dblLink7CogX*sin(q7)) + sin(q5)*(KUKA_LBR_param_.dblLink7CogX*cos(q7) - KUKA_LBR_param_.dblLink7CogY*sin(q7))))) + sin(q1)*(sin(q2)*(cos(q7)*(KUKA_LBR_param_.dblLink7CogX*sin(q4)*sin(q5) - KUKA_LBR_param_.dblLink7CogY*cos(q4)*sin(q6)) - (KUKA_LBR_param_.dblLink7CogY*sin(q4)*sin(q5) + KUKA_LBR_param_.dblLink7CogX*cos(q4)*sin(q6))*sin(q7) + cos(q5)*cos(q6)*sin(q4)*(KUKA_LBR_param_.dblLink7CogY*cos(q7) + KUKA_LBR_param_.dblLink7CogX*sin(q7))) + cos(q2)*(sin(q3)*(-(cos(q6)*sin(q5)*(KUKA_LBR_param_.dblLink7CogY*cos(q7) + KUKA_LBR_param_.dblLink7CogX*sin(q7))) + cos(q5)*(KUKA_LBR_param_.dblLink7CogX*cos(q7) - KUKA_LBR_param_.dblLink7CogY*sin(q7))) + cos(q3)*(sin(q4)*sin(q6)*(KUKA_LBR_param_.dblLink7CogY*cos(q7) + KUKA_LBR_param_.dblLink7CogX*sin(q7)) + cos(q4)*(cos(q5)*cos(q6)*(KUKA_LBR_param_.dblLink7CogY*cos(q7) + KUKA_LBR_param_.dblLink7CogX*sin(q7)) + sin(q5)*(KUKA_LBR_param_.dblLink7CogX*cos(q7) - KUKA_LBR_param_.dblLink7CogY*sin(q7)))))));
dblMassInertFullRow7Col6 = (-(cos(q5)*(cos(q3)*sin(q1) + cos(q1)*cos(q2)*sin(q3))) + (cos(q4)*sin(q1)*sin(q3) - cos(q1)*(cos(q2)*cos(q3)*cos(q4) + sin(q2)*sin(q4)))*sin(q5))*(KUKA_LBR_param_.dblLink7InertXX*(cos(q6)*(sin(q1)*sin(q3)*sin(q4) + cos(q1)*(cos(q4)*sin(q2) - cos(q2)*cos(q3)*sin(q4))) - (cos(q5)*(cos(q4)*sin(q1)*sin(q3) - cos(q1)*(cos(q2)*cos(q3)*cos(q4) + sin(q2)*sin(q4))) + (cos(q3)*sin(q1) + cos(q1)*cos(q2)*sin(q3))*sin(q5))*sin(q6)) + KUKA_LBR_param_.dblLink7InertXY*(cos(q6)*(cos(q4)*sin(q1)*sin(q2) - (cos(q2)*cos(q3)*sin(q1) + cos(q1)*sin(q3))*sin(q4)) + (cos(q5)*sin(q1)*sin(q2)*sin(q4) + cos(q1)*(cos(q4)*cos(q5)*sin(q3) + cos(q3)*sin(q5)) + cos(q2)*sin(q1)*(cos(q3)*cos(q4)*cos(q5) - sin(q3)*sin(q5)))*sin(q6)) + KUKA_LBR_param_.dblLink7InertXZ*(cos(q2)*(cos(q4)*cos(q6) + cos(q5)*sin(q4)*sin(q6)) + sin(q2)*(sin(q3)*sin(q5)*sin(q6) + cos(q3)*(cos(q6)*sin(q4) - cos(q4)*cos(q5)*sin(q6))))) + (cos(q1)*(cos(q3)*cos(q5) - cos(q4)*sin(q3)*sin(q5)) - sin(q1)*(sin(q2)*sin(q4)*sin(q5) + cos(q2)*(cos(q5)*sin(q3) + cos(q3)*cos(q4)*sin(q5))))*(KUKA_LBR_param_.dblLink7InertXY*(cos(q6)*(sin(q1)*sin(q3)*sin(q4) + cos(q1)*(cos(q4)*sin(q2) - cos(q2)*cos(q3)*sin(q4))) - (cos(q5)*(cos(q4)*sin(q1)*sin(q3) - cos(q1)*(cos(q2)*cos(q3)*cos(q4) + sin(q2)*sin(q4))) + (cos(q3)*sin(q1) + cos(q1)*cos(q2)*sin(q3))*sin(q5))*sin(q6)) + KUKA_LBR_param_.dblLink7InertYY*(cos(q6)*(cos(q4)*sin(q1)*sin(q2) - (cos(q2)*cos(q3)*sin(q1) + cos(q1)*sin(q3))*sin(q4)) + (cos(q5)*sin(q1)*sin(q2)*sin(q4) + cos(q1)*(cos(q4)*cos(q5)*sin(q3) + cos(q3)*sin(q5)) + cos(q2)*sin(q1)*(cos(q3)*cos(q4)*cos(q5) - sin(q3)*sin(q5)))*sin(q6)) + KUKA_LBR_param_.dblLink7InertYZ*(cos(q2)*(cos(q4)*cos(q6) + cos(q5)*sin(q4)*sin(q6)) + sin(q2)*(sin(q3)*sin(q5)*sin(q6) + cos(q3)*(cos(q6)*sin(q4) - cos(q4)*cos(q5)*sin(q6))))) + (cos(q5)*sin(q2)*sin(q3) + (cos(q3)*cos(q4)*sin(q2) - cos(q2)*sin(q4))*sin(q5))*(KUKA_LBR_param_.dblLink7InertXZ*(cos(q6)*(sin(q1)*sin(q3)*sin(q4) + cos(q1)*(cos(q4)*sin(q2) - cos(q2)*cos(q3)*sin(q4))) - (cos(q5)*(cos(q4)*sin(q1)*sin(q3) - cos(q1)*(cos(q2)*cos(q3)*cos(q4) + sin(q2)*sin(q4))) + (cos(q3)*sin(q1) + cos(q1)*cos(q2)*sin(q3))*sin(q5))*sin(q6)) + KUKA_LBR_param_.dblLink7InertYZ*(cos(q6)*(cos(q4)*sin(q1)*sin(q2) - (cos(q2)*cos(q3)*sin(q1) + cos(q1)*sin(q3))*sin(q4)) + (cos(q5)*sin(q1)*sin(q2)*sin(q4) + cos(q1)*(cos(q4)*cos(q5)*sin(q3) + cos(q3)*sin(q5)) + cos(q2)*sin(q1)*(cos(q3)*cos(q4)*cos(q5) - sin(q3)*sin(q5)))*sin(q6)) + KUKA_LBR_param_.dblLink7InertZZ*(cos(q2)*(cos(q4)*cos(q6) + cos(q5)*sin(q4)*sin(q6)) + sin(q2)*(sin(q3)*sin(q5)*sin(q6) + cos(q3)*(cos(q6)*sin(q4) - cos(q4)*cos(q5)*sin(q6))))) - KUKA_LBR_param_.dblLink7Mass*(-(KUKA_LBR_param_.dblLink7CogY*cos(q6)*cos(q7)*sin(q2)*sin(q3)*sin(q5)) - KUKA_LBR_param_.dblLink7CogX*cos(q2)*cos(q7)*sin(q4)*sin(q5) + KUKA_LBR_param_.dblLink7CogY*cos(q2)*cos(q4)*cos(q7)*sin(q6) - KUKA_LBR_param_.dblLink7CogX*cos(q6)*sin(q2)*sin(q3)*sin(q5)*sin(q7) + KUKA_LBR_param_.dblLink7CogY*cos(q2)*sin(q4)*sin(q5)*sin(q7) + KUKA_LBR_param_.dblLink7CogX*cos(q2)*cos(q4)*sin(q6)*sin(q7) + cos(q5)*(cos(q7)*(KUKA_LBR_param_.dblLink7CogX*sin(q2)*sin(q3) - KUKA_LBR_param_.dblLink7CogY*cos(q2)*cos(q6)*sin(q4)) - (KUKA_LBR_param_.dblLink7CogY*sin(q2)*sin(q3) + KUKA_LBR_param_.dblLink7CogX*cos(q2)*cos(q6)*sin(q4))*sin(q7)) + cos(q3)*sin(q2)*(sin(q4)*sin(q6)*(KUKA_LBR_param_.dblLink7CogY*cos(q7) + KUKA_LBR_param_.dblLink7CogX*sin(q7)) + cos(q4)*(cos(q5)*cos(q6)*(KUKA_LBR_param_.dblLink7CogY*cos(q7) + KUKA_LBR_param_.dblLink7CogX*sin(q7)) + sin(q5)*(KUKA_LBR_param_.dblLink7CogX*cos(q7) - KUKA_LBR_param_.dblLink7CogY*sin(q7)))))*(cos(q2)*(cos(q4)*(KUKA_LBR_param_.dblLink7CogX*cos(q6)*cos(q7) - KUKA_LBR_param_.dblLink7CogZ*sin(q6) - KUKA_LBR_param_.dblLink7CogY*cos(q6)*sin(q7)) + cos(q5)*sin(q4)*(KUKA_LBR_param_.dblLink7CogZ*cos(q6) + KUKA_LBR_param_.dblLink7CogX*cos(q7)*sin(q6) - KUKA_LBR_param_.dblLink7CogY*sin(q6)*sin(q7))) - sin(q2)*(-(sin(q3)*sin(q5)*(KUKA_LBR_param_.dblLink7CogZ*cos(q6) + sin(q6)*(KUKA_LBR_param_.dblLink7CogX*cos(q7) - KUKA_LBR_param_.dblLink7CogY*sin(q7)))) + cos(q3)*(sin(q4)*(-(KUKA_LBR_param_.dblLink7CogX*cos(q6)*cos(q7)) + KUKA_LBR_param_.dblLink7CogZ*sin(q6) + KUKA_LBR_param_.dblLink7CogY*cos(q6)*sin(q7)) + cos(q4)*cos(q5)*(KUKA_LBR_param_.dblLink7CogZ*cos(q6) + KUKA_LBR_param_.dblLink7CogX*cos(q7)*sin(q6) - KUKA_LBR_param_.dblLink7CogY*sin(q6)*sin(q7))))) + KUKA_LBR_param_.dblLink7Mass*(-(sin(q1)*(cos(q6)*(-(KUKA_LBR_param_.dblLink7CogX*cos(q7)*sin(q3)*sin(q4)) + KUKA_LBR_param_.dblLink7CogZ*cos(q3)*sin(q5) + KUKA_LBR_param_.dblLink7CogY*sin(q3)*sin(q4)*sin(q7)) + sin(q6)*(KUKA_LBR_param_.dblLink7CogZ*sin(q3)*sin(q4) + cos(q3)*sin(q5)*(KUKA_LBR_param_.dblLink7CogX*cos(q7) - KUKA_LBR_param_.dblLink7CogY*sin(q7))) + cos(q4)*cos(q5)*sin(q3)*(KUKA_LBR_param_.dblLink7CogZ*cos(q6) + sin(q6)*(KUKA_LBR_param_.dblLink7CogX*cos(q7) - KUKA_LBR_param_.dblLink7CogY*sin(q7))))) + cos(q1)*(sin(q2)*(cos(q4)*(KUKA_LBR_param_.dblLink7CogX*cos(q6)*cos(q7) - KUKA_LBR_param_.dblLink7CogZ*sin(q6) - KUKA_LBR_param_.dblLink7CogY*cos(q6)*sin(q7)) + cos(q5)*sin(q4)*(KUKA_LBR_param_.dblLink7CogZ*cos(q6) + KUKA_LBR_param_.dblLink7CogX*cos(q7)*sin(q6) - KUKA_LBR_param_.dblLink7CogY*sin(q6)*sin(q7))) + cos(q2)*(-(sin(q3)*sin(q5)*(KUKA_LBR_param_.dblLink7CogZ*cos(q6) + sin(q6)*(KUKA_LBR_param_.dblLink7CogX*cos(q7) - KUKA_LBR_param_.dblLink7CogY*sin(q7)))) + cos(q3)*(sin(q4)*(-(KUKA_LBR_param_.dblLink7CogX*cos(q6)*cos(q7)) + KUKA_LBR_param_.dblLink7CogZ*sin(q6) + KUKA_LBR_param_.dblLink7CogY*cos(q6)*sin(q7)) + cos(q4)*cos(q5)*(KUKA_LBR_param_.dblLink7CogZ*cos(q6) + KUKA_LBR_param_.dblLink7CogX*cos(q7)*sin(q6) - KUKA_LBR_param_.dblLink7CogY*sin(q6)*sin(q7))))))*(sin(q1)*(cos(q3)*(-(cos(q6)*sin(q5)*(KUKA_LBR_param_.dblLink7CogY*cos(q7) + KUKA_LBR_param_.dblLink7CogX*sin(q7))) + cos(q5)*(KUKA_LBR_param_.dblLink7CogX*cos(q7) - KUKA_LBR_param_.dblLink7CogY*sin(q7))) - sin(q3)*(sin(q4)*sin(q6)*(KUKA_LBR_param_.dblLink7CogY*cos(q7) + KUKA_LBR_param_.dblLink7CogX*sin(q7)) + cos(q4)*(cos(q5)*cos(q6)*(KUKA_LBR_param_.dblLink7CogY*cos(q7) + KUKA_LBR_param_.dblLink7CogX*sin(q7)) + sin(q5)*(KUKA_LBR_param_.dblLink7CogX*cos(q7) - KUKA_LBR_param_.dblLink7CogY*sin(q7))))) + cos(q1)*(sin(q2)*(cos(q7)*(KUKA_LBR_param_.dblLink7CogX*sin(q4)*sin(q5) - KUKA_LBR_param_.dblLink7CogY*cos(q4)*sin(q6)) - (KUKA_LBR_param_.dblLink7CogY*sin(q4)*sin(q5) + KUKA_LBR_param_.dblLink7CogX*cos(q4)*sin(q6))*sin(q7) + cos(q5)*cos(q6)*sin(q4)*(KUKA_LBR_param_.dblLink7CogY*cos(q7) + KUKA_LBR_param_.dblLink7CogX*sin(q7))) + cos(q2)*(sin(q3)*(-(cos(q6)*sin(q5)*(KUKA_LBR_param_.dblLink7CogY*cos(q7) + KUKA_LBR_param_.dblLink7CogX*sin(q7))) + cos(q5)*(KUKA_LBR_param_.dblLink7CogX*cos(q7) - KUKA_LBR_param_.dblLink7CogY*sin(q7))) + cos(q3)*(sin(q4)*sin(q6)*(KUKA_LBR_param_.dblLink7CogY*cos(q7) + KUKA_LBR_param_.dblLink7CogX*sin(q7)) + cos(q4)*(cos(q5)*cos(q6)*(KUKA_LBR_param_.dblLink7CogY*cos(q7) + KUKA_LBR_param_.dblLink7CogX*sin(q7)) + sin(q5)*(KUKA_LBR_param_.dblLink7CogX*cos(q7) - KUKA_LBR_param_.dblLink7CogY*sin(q7))))))) + KUKA_LBR_param_.dblLink7Mass*(KUKA_LBR_param_.dblLink7CogZ*cos(q5)*cos(q6)*sin(q1)*sin(q2)*sin(q4) - KUKA_LBR_param_.dblLink7CogX*cos(q1)*cos(q6)*cos(q7)*sin(q3)*sin(q4) + KUKA_LBR_param_.dblLink7CogZ*cos(q1)*cos(q3)*cos(q6)*sin(q5) + KUKA_LBR_param_.dblLink7CogX*cos(q5)*cos(q7)*sin(q1)*sin(q2)*sin(q4)*sin(q6) + KUKA_LBR_param_.dblLink7CogZ*cos(q1)*sin(q3)*sin(q4)*sin(q6) + KUKA_LBR_param_.dblLink7CogX*cos(q1)*cos(q3)*cos(q7)*sin(q5)*sin(q6) + KUKA_LBR_param_.dblLink7CogY*cos(q1)*cos(q6)*sin(q3)*sin(q4)*sin(q7) - KUKA_LBR_param_.dblLink7CogY*cos(q5)*sin(q1)*sin(q2)*sin(q4)*sin(q6)*sin(q7) - KUKA_LBR_param_.dblLink7CogY*cos(q1)*cos(q3)*sin(q5)*sin(q6)*sin(q7) + cos(q4)*(cos(q6)*(KUKA_LBR_param_.dblLink7CogX*cos(q7)*sin(q1)*sin(q2) + KUKA_LBR_param_.dblLink7CogZ*cos(q1)*cos(q5)*sin(q3) - KUKA_LBR_param_.dblLink7CogY*sin(q1)*sin(q2)*sin(q7)) - sin(q6)*(KUKA_LBR_param_.dblLink7CogZ*sin(q1)*sin(q2) + cos(q1)*cos(q5)*sin(q3)*(-(KUKA_LBR_param_.dblLink7CogX*cos(q7)) + KUKA_LBR_param_.dblLink7CogY*sin(q7)))) + cos(q2)*sin(q1)*(-(sin(q3)*sin(q5)*(KUKA_LBR_param_.dblLink7CogZ*cos(q6) + sin(q6)*(KUKA_LBR_param_.dblLink7CogX*cos(q7) - KUKA_LBR_param_.dblLink7CogY*sin(q7)))) + cos(q3)*(sin(q4)*(-(KUKA_LBR_param_.dblLink7CogX*cos(q6)*cos(q7)) + KUKA_LBR_param_.dblLink7CogZ*sin(q6) + KUKA_LBR_param_.dblLink7CogY*cos(q6)*sin(q7)) + cos(q4)*cos(q5)*(KUKA_LBR_param_.dblLink7CogZ*cos(q6) + KUKA_LBR_param_.dblLink7CogX*cos(q7)*sin(q6) - KUKA_LBR_param_.dblLink7CogY*sin(q6)*sin(q7)))))*(cos(q1)*(cos(q3)*(cos(q6)*sin(q5)*(KUKA_LBR_param_.dblLink7CogY*cos(q7) + KUKA_LBR_param_.dblLink7CogX*sin(q7)) + cos(q5)*(-(KUKA_LBR_param_.dblLink7CogX*cos(q7)) + KUKA_LBR_param_.dblLink7CogY*sin(q7))) + sin(q3)*(sin(q4)*sin(q6)*(KUKA_LBR_param_.dblLink7CogY*cos(q7) + KUKA_LBR_param_.dblLink7CogX*sin(q7)) + cos(q4)*(cos(q5)*cos(q6)*(KUKA_LBR_param_.dblLink7CogY*cos(q7) + KUKA_LBR_param_.dblLink7CogX*sin(q7)) + sin(q5)*(KUKA_LBR_param_.dblLink7CogX*cos(q7) - KUKA_LBR_param_.dblLink7CogY*sin(q7))))) + sin(q1)*(sin(q2)*(cos(q7)*(KUKA_LBR_param_.dblLink7CogX*sin(q4)*sin(q5) - KUKA_LBR_param_.dblLink7CogY*cos(q4)*sin(q6)) - (KUKA_LBR_param_.dblLink7CogY*sin(q4)*sin(q5) + KUKA_LBR_param_.dblLink7CogX*cos(q4)*sin(q6))*sin(q7) + cos(q5)*cos(q6)*sin(q4)*(KUKA_LBR_param_.dblLink7CogY*cos(q7) + KUKA_LBR_param_.dblLink7CogX*sin(q7))) + cos(q2)*(sin(q3)*(-(cos(q6)*sin(q5)*(KUKA_LBR_param_.dblLink7CogY*cos(q7) + KUKA_LBR_param_.dblLink7CogX*sin(q7))) + cos(q5)*(KUKA_LBR_param_.dblLink7CogX*cos(q7) - KUKA_LBR_param_.dblLink7CogY*sin(q7))) + cos(q3)*(sin(q4)*sin(q6)*(KUKA_LBR_param_.dblLink7CogY*cos(q7) + KUKA_LBR_param_.dblLink7CogX*sin(q7)) + cos(q4)*(cos(q5)*cos(q6)*(KUKA_LBR_param_.dblLink7CogY*cos(q7) + KUKA_LBR_param_.dblLink7CogX*sin(q7)) + sin(q5)*(KUKA_LBR_param_.dblLink7CogX*cos(q7) - KUKA_LBR_param_.dblLink7CogY*sin(q7)))))));
dblMassInertFullRow7Col7 = (cos(q6)*(sin(q1)*sin(q3)*sin(q4) + cos(q1)*(cos(q4)*sin(q2) - cos(q2)*cos(q3)*sin(q4))) - (cos(q5)*(cos(q4)*sin(q1)*sin(q3) - cos(q1)*(cos(q2)*cos(q3)*cos(q4) + sin(q2)*sin(q4))) + (cos(q3)*sin(q1) + cos(q1)*cos(q2)*sin(q3))*sin(q5))*sin(q6))*(KUKA_LBR_param_.dblLink7InertXX*(cos(q6)*(sin(q1)*sin(q3)*sin(q4) + cos(q1)*(cos(q4)*sin(q2) - cos(q2)*cos(q3)*sin(q4))) - (cos(q5)*(cos(q4)*sin(q1)*sin(q3) - cos(q1)*(cos(q2)*cos(q3)*cos(q4) + sin(q2)*sin(q4))) + (cos(q3)*sin(q1) + cos(q1)*cos(q2)*sin(q3))*sin(q5))*sin(q6)) + KUKA_LBR_param_.dblLink7InertXY*(cos(q6)*(cos(q4)*sin(q1)*sin(q2) - (cos(q2)*cos(q3)*sin(q1) + cos(q1)*sin(q3))*sin(q4)) + (cos(q5)*sin(q1)*sin(q2)*sin(q4) + cos(q1)*(cos(q4)*cos(q5)*sin(q3) + cos(q3)*sin(q5)) + cos(q2)*sin(q1)*(cos(q3)*cos(q4)*cos(q5) - sin(q3)*sin(q5)))*sin(q6)) + KUKA_LBR_param_.dblLink7InertXZ*(cos(q2)*(cos(q4)*cos(q6) + cos(q5)*sin(q4)*sin(q6)) + sin(q2)*(sin(q3)*sin(q5)*sin(q6) + cos(q3)*(cos(q6)*sin(q4) - cos(q4)*cos(q5)*sin(q6))))) + (cos(q6)*(cos(q4)*sin(q1)*sin(q2) - (cos(q2)*cos(q3)*sin(q1) + cos(q1)*sin(q3))*sin(q4)) + (cos(q5)*sin(q1)*sin(q2)*sin(q4) + cos(q1)*(cos(q4)*cos(q5)*sin(q3) + cos(q3)*sin(q5)) + cos(q2)*sin(q1)*(cos(q3)*cos(q4)*cos(q5) - sin(q3)*sin(q5)))*sin(q6))*(KUKA_LBR_param_.dblLink7InertXY*(cos(q6)*(sin(q1)*sin(q3)*sin(q4) + cos(q1)*(cos(q4)*sin(q2) - cos(q2)*cos(q3)*sin(q4))) - (cos(q5)*(cos(q4)*sin(q1)*sin(q3) - cos(q1)*(cos(q2)*cos(q3)*cos(q4) + sin(q2)*sin(q4))) + (cos(q3)*sin(q1) + cos(q1)*cos(q2)*sin(q3))*sin(q5))*sin(q6)) + KUKA_LBR_param_.dblLink7InertYY*(cos(q6)*(cos(q4)*sin(q1)*sin(q2) - (cos(q2)*cos(q3)*sin(q1) + cos(q1)*sin(q3))*sin(q4)) + (cos(q5)*sin(q1)*sin(q2)*sin(q4) + cos(q1)*(cos(q4)*cos(q5)*sin(q3) + cos(q3)*sin(q5)) + cos(q2)*sin(q1)*(cos(q3)*cos(q4)*cos(q5) - sin(q3)*sin(q5)))*sin(q6)) + KUKA_LBR_param_.dblLink7InertYZ*(cos(q2)*(cos(q4)*cos(q6) + cos(q5)*sin(q4)*sin(q6)) + sin(q2)*(sin(q3)*sin(q5)*sin(q6) + cos(q3)*(cos(q6)*sin(q4) - cos(q4)*cos(q5)*sin(q6))))) + (cos(q2)*(cos(q4)*cos(q6) + cos(q5)*sin(q4)*sin(q6)) + sin(q2)*(sin(q3)*sin(q5)*sin(q6) + cos(q3)*(cos(q6)*sin(q4) - cos(q4)*cos(q5)*sin(q6))))*(KUKA_LBR_param_.dblLink7InertXZ*(cos(q6)*(sin(q1)*sin(q3)*sin(q4) + cos(q1)*(cos(q4)*sin(q2) - cos(q2)*cos(q3)*sin(q4))) - (cos(q5)*(cos(q4)*sin(q1)*sin(q3) - cos(q1)*(cos(q2)*cos(q3)*cos(q4) + sin(q2)*sin(q4))) + (cos(q3)*sin(q1) + cos(q1)*cos(q2)*sin(q3))*sin(q5))*sin(q6)) + KUKA_LBR_param_.dblLink7InertYZ*(cos(q6)*(cos(q4)*sin(q1)*sin(q2) - (cos(q2)*cos(q3)*sin(q1) + cos(q1)*sin(q3))*sin(q4)) + (cos(q5)*sin(q1)*sin(q2)*sin(q4) + cos(q1)*(cos(q4)*cos(q5)*sin(q3) + cos(q3)*sin(q5)) + cos(q2)*sin(q1)*(cos(q3)*cos(q4)*cos(q5) - sin(q3)*sin(q5)))*sin(q6)) + KUKA_LBR_param_.dblLink7InertZZ*(cos(q2)*(cos(q4)*cos(q6) + cos(q5)*sin(q4)*sin(q6)) + sin(q2)*(sin(q3)*sin(q5)*sin(q6) + cos(q3)*(cos(q6)*sin(q4) - cos(q4)*cos(q5)*sin(q6))))) + KUKA_LBR_param_.dblLink7Mass*power(-(KUKA_LBR_param_.dblLink7CogY*cos(q6)*cos(q7)*sin(q2)*sin(q3)*sin(q5)) - KUKA_LBR_param_.dblLink7CogX*cos(q2)*cos(q7)*sin(q4)*sin(q5) + KUKA_LBR_param_.dblLink7CogY*cos(q2)*cos(q4)*cos(q7)*sin(q6) - KUKA_LBR_param_.dblLink7CogX*cos(q6)*sin(q2)*sin(q3)*sin(q5)*sin(q7) + KUKA_LBR_param_.dblLink7CogY*cos(q2)*sin(q4)*sin(q5)*sin(q7) + KUKA_LBR_param_.dblLink7CogX*cos(q2)*cos(q4)*sin(q6)*sin(q7) + cos(q5)*(cos(q7)*(KUKA_LBR_param_.dblLink7CogX*sin(q2)*sin(q3) - KUKA_LBR_param_.dblLink7CogY*cos(q2)*cos(q6)*sin(q4)) - (KUKA_LBR_param_.dblLink7CogY*sin(q2)*sin(q3) + KUKA_LBR_param_.dblLink7CogX*cos(q2)*cos(q6)*sin(q4))*sin(q7)) + cos(q3)*sin(q2)*(sin(q4)*sin(q6)*(KUKA_LBR_param_.dblLink7CogY*cos(q7) + KUKA_LBR_param_.dblLink7CogX*sin(q7)) + cos(q4)*(cos(q5)*cos(q6)*(KUKA_LBR_param_.dblLink7CogY*cos(q7) + KUKA_LBR_param_.dblLink7CogX*sin(q7)) + sin(q5)*(KUKA_LBR_param_.dblLink7CogX*cos(q7) - KUKA_LBR_param_.dblLink7CogY*sin(q7)))),2) + KUKA_LBR_param_.dblLink7Mass*power(sin(q1)*(cos(q3)*(-(cos(q6)*sin(q5)*(KUKA_LBR_param_.dblLink7CogY*cos(q7) + KUKA_LBR_param_.dblLink7CogX*sin(q7))) + cos(q5)*(KUKA_LBR_param_.dblLink7CogX*cos(q7) - KUKA_LBR_param_.dblLink7CogY*sin(q7))) - sin(q3)*(sin(q4)*sin(q6)*(KUKA_LBR_param_.dblLink7CogY*cos(q7) + KUKA_LBR_param_.dblLink7CogX*sin(q7)) + cos(q4)*(cos(q5)*cos(q6)*(KUKA_LBR_param_.dblLink7CogY*cos(q7) + KUKA_LBR_param_.dblLink7CogX*sin(q7)) + sin(q5)*(KUKA_LBR_param_.dblLink7CogX*cos(q7) - KUKA_LBR_param_.dblLink7CogY*sin(q7))))) + cos(q1)*(sin(q2)*(cos(q7)*(KUKA_LBR_param_.dblLink7CogX*sin(q4)*sin(q5) - KUKA_LBR_param_.dblLink7CogY*cos(q4)*sin(q6)) - (KUKA_LBR_param_.dblLink7CogY*sin(q4)*sin(q5) + KUKA_LBR_param_.dblLink7CogX*cos(q4)*sin(q6))*sin(q7) + cos(q5)*cos(q6)*sin(q4)*(KUKA_LBR_param_.dblLink7CogY*cos(q7) + KUKA_LBR_param_.dblLink7CogX*sin(q7))) + cos(q2)*(sin(q3)*(-(cos(q6)*sin(q5)*(KUKA_LBR_param_.dblLink7CogY*cos(q7) + KUKA_LBR_param_.dblLink7CogX*sin(q7))) + cos(q5)*(KUKA_LBR_param_.dblLink7CogX*cos(q7) - KUKA_LBR_param_.dblLink7CogY*sin(q7))) + cos(q3)*(sin(q4)*sin(q6)*(KUKA_LBR_param_.dblLink7CogY*cos(q7) + KUKA_LBR_param_.dblLink7CogX*sin(q7)) + cos(q4)*(cos(q5)*cos(q6)*(KUKA_LBR_param_.dblLink7CogY*cos(q7) + KUKA_LBR_param_.dblLink7CogX*sin(q7)) + sin(q5)*(KUKA_LBR_param_.dblLink7CogX*cos(q7) - KUKA_LBR_param_.dblLink7CogY*sin(q7)))))),2) + KUKA_LBR_param_.dblLink7Mass*power(cos(q1)*(cos(q3)*(cos(q6)*sin(q5)*(KUKA_LBR_param_.dblLink7CogY*cos(q7) + KUKA_LBR_param_.dblLink7CogX*sin(q7)) + cos(q5)*(-(KUKA_LBR_param_.dblLink7CogX*cos(q7)) + KUKA_LBR_param_.dblLink7CogY*sin(q7))) + sin(q3)*(sin(q4)*sin(q6)*(KUKA_LBR_param_.dblLink7CogY*cos(q7) + KUKA_LBR_param_.dblLink7CogX*sin(q7)) + cos(q4)*(cos(q5)*cos(q6)*(KUKA_LBR_param_.dblLink7CogY*cos(q7) + KUKA_LBR_param_.dblLink7CogX*sin(q7)) + sin(q5)*(KUKA_LBR_param_.dblLink7CogX*cos(q7) - KUKA_LBR_param_.dblLink7CogY*sin(q7))))) + sin(q1)*(sin(q2)*(cos(q7)*(KUKA_LBR_param_.dblLink7CogX*sin(q4)*sin(q5) - KUKA_LBR_param_.dblLink7CogY*cos(q4)*sin(q6)) - (KUKA_LBR_param_.dblLink7CogY*sin(q4)*sin(q5) + KUKA_LBR_param_.dblLink7CogX*cos(q4)*sin(q6))*sin(q7) + cos(q5)*cos(q6)*sin(q4)*(KUKA_LBR_param_.dblLink7CogY*cos(q7) + KUKA_LBR_param_.dblLink7CogX*sin(q7))) + cos(q2)*(sin(q3)*(-(cos(q6)*sin(q5)*(KUKA_LBR_param_.dblLink7CogY*cos(q7) + KUKA_LBR_param_.dblLink7CogX*sin(q7))) + cos(q5)*(KUKA_LBR_param_.dblLink7CogX*cos(q7) - KUKA_LBR_param_.dblLink7CogY*sin(q7))) + cos(q3)*(sin(q4)*sin(q6)*(KUKA_LBR_param_.dblLink7CogY*cos(q7) + KUKA_LBR_param_.dblLink7CogX*sin(q7)) + cos(q4)*(cos(q5)*cos(q6)*(KUKA_LBR_param_.dblLink7CogY*cos(q7) + KUKA_LBR_param_.dblLink7CogX*sin(q7)) + sin(q5)*(KUKA_LBR_param_.dblLink7CogX*cos(q7) - KUKA_LBR_param_.dblLink7CogY*sin(q7)))))),2);

% matCoriolisCentrifugalFull %
dblCoriolisCentrifugalFullRow1Col1 = KUKA_LBR_param_.dblLink7Mass*q14*((cos(q1)*(cos(q3)*(-(cos(q6)*sin(q5)*(KUKA_LBR_param_.dblLink7CogY*cos(q7) + KUKA_LBR_param_.dblLink7CogX*sin(q7))) + cos(q5)*(KUKA_LBR_param_.dblLink7CogX*cos(q7) - KUKA_LBR_param_.dblLink7CogY*sin(q7))) - sin(q3)*(sin(q4)*sin(q6)*(KUKA_LBR_param_.dblLink7CogY*cos(q7) + KUKA_LBR_param_.dblLink7CogX*sin(q7)) + cos(q4)*(cos(q5)*cos(q6)*(KUKA_LBR_param_.dblLink7CogY*cos(q7) + KUKA_LBR_param_.dblLink7CogX*sin(q7)) + sin(q5)*(KUKA_LBR_param_.dblLink7CogX*cos(q7) - KUKA_LBR_param_.dblLink7CogY*sin(q7))))) + sin(q1)*(-(sin(q2)*(KUKA_LBR_param_.dblLink7CogX*cos(q7)*sin(q4)*sin(q5) - KUKA_LBR_param_.dblLink7CogY*sin(q4)*sin(q5)*sin(q7) + cos(q5)*cos(q6)*sin(q4)*(KUKA_LBR_param_.dblLink7CogY*cos(q7) + KUKA_LBR_param_.dblLink7CogX*sin(q7)) - cos(q4)*sin(q6)*(KUKA_LBR_param_.dblLink7CogY*cos(q7) + KUKA_LBR_param_.dblLink7CogX*sin(q7)))) + cos(q2)*(sin(q3)*(cos(q6)*sin(q5)*(KUKA_LBR_param_.dblLink7CogY*cos(q7) + KUKA_LBR_param_.dblLink7CogX*sin(q7)) + cos(q5)*(-(KUKA_LBR_param_.dblLink7CogX*cos(q7)) + KUKA_LBR_param_.dblLink7CogY*sin(q7))) - cos(q3)*(sin(q4)*sin(q6)*(KUKA_LBR_param_.dblLink7CogY*cos(q7) + KUKA_LBR_param_.dblLink7CogX*sin(q7)) + cos(q4)*(cos(q5)*cos(q6)*(KUKA_LBR_param_.dblLink7CogY*cos(q7) + KUKA_LBR_param_.dblLink7CogX*sin(q7)) + sin(q5)*(KUKA_LBR_param_.dblLink7CogX*cos(q7) - KUKA_LBR_param_.dblLink7CogY*sin(q7)))))))*(cos(q1)*(cos(q3)*(cos(q5)*(KUKA_LBR_param_.dblLink7CogY*cos(q7) + KUKA_LBR_param_.dblLink7CogX*sin(q7)) + sin(q5)*(KUKA_LBR_param_.dblLink7CogX*cos(q6)*cos(q7) - KUKA_LBR_param_.dblLink7CogZ*sin(q6) - KUKA_LBR_param_.dblLink7CogY*cos(q6)*sin(q7))) + sin(q3)*(sin(q4)*(KUKA_LBR_param_.dblLink45Len + KUKA_LBR_param_.dblLink7CogZ*cos(q6) + KUKA_LBR_param_.dblLink7CogX*cos(q7)*sin(q6) - KUKA_LBR_param_.dblLink7CogY*sin(q6)*sin(q7)) - cos(q4)*(sin(q5)*(KUKA_LBR_param_.dblLink7CogY*cos(q7) + KUKA_LBR_param_.dblLink7CogX*sin(q7)) + cos(q5)*(-(KUKA_LBR_param_.dblLink7CogX*cos(q6)*cos(q7)) + KUKA_LBR_param_.dblLink7CogZ*sin(q6) + KUKA_LBR_param_.dblLink7CogY*cos(q6)*sin(q7))))) + sin(q1)*(-(sin(q2)*(KUKA_LBR_param_.dblLink23Len + KUKA_LBR_param_.dblLink7CogY*cos(q7)*sin(q4)*sin(q5) + KUKA_LBR_param_.dblLink7CogX*sin(q4)*sin(q5)*sin(q7) + cos(q5)*sin(q4)*(-(KUKA_LBR_param_.dblLink7CogX*cos(q6)*cos(q7)) + KUKA_LBR_param_.dblLink7CogZ*sin(q6) + KUKA_LBR_param_.dblLink7CogY*cos(q6)*sin(q7)) + cos(q4)*(KUKA_LBR_param_.dblLink45Len + KUKA_LBR_param_.dblLink7CogZ*cos(q6) + KUKA_LBR_param_.dblLink7CogX*cos(q7)*sin(q6) - KUKA_LBR_param_.dblLink7CogY*sin(q6)*sin(q7)))) + cos(q2)*(-(sin(q3)*(cos(q5)*(KUKA_LBR_param_.dblLink7CogY*cos(q7) + KUKA_LBR_param_.dblLink7CogX*sin(q7)) + sin(q5)*(KUKA_LBR_param_.dblLink7CogX*cos(q6)*cos(q7) - KUKA_LBR_param_.dblLink7CogZ*sin(q6) - KUKA_LBR_param_.dblLink7CogY*cos(q6)*sin(q7)))) + cos(q3)*(sin(q4)*(KUKA_LBR_param_.dblLink45Len + KUKA_LBR_param_.dblLink7CogZ*cos(q6) + KUKA_LBR_param_.dblLink7CogX*cos(q7)*sin(q6) - KUKA_LBR_param_.dblLink7CogY*sin(q6)*sin(q7)) - cos(q4)*(sin(q5)*(KUKA_LBR_param_.dblLink7CogY*cos(q7) + KUKA_LBR_param_.dblLink7CogX*sin(q7)) + cos(q5)*(-(KUKA_LBR_param_.dblLink7CogX*cos(q6)*cos(q7)) + KUKA_LBR_param_.dblLink7CogZ*sin(q6) + KUKA_LBR_param_.dblLink7CogY*cos(q6)*sin(q7))))))) + (sin(q1)*(cos(q3)*(-(cos(q6)*sin(q5)*(KUKA_LBR_param_.dblLink7CogY*cos(q7) + KUKA_LBR_param_.dblLink7CogX*sin(q7))) + cos(q5)*(KUKA_LBR_param_.dblLink7CogX*cos(q7) - KUKA_LBR_param_.dblLink7CogY*sin(q7))) - sin(q3)*(sin(q4)*sin(q6)*(KUKA_LBR_param_.dblLink7CogY*cos(q7) + KUKA_LBR_param_.dblLink7CogX*sin(q7)) + cos(q4)*(cos(q5)*cos(q6)*(KUKA_LBR_param_.dblLink7CogY*cos(q7) + KUKA_LBR_param_.dblLink7CogX*sin(q7)) + sin(q5)*(KUKA_LBR_param_.dblLink7CogX*cos(q7) - KUKA_LBR_param_.dblLink7CogY*sin(q7))))) + cos(q1)*(sin(q2)*(KUKA_LBR_param_.dblLink7CogX*cos(q7)*sin(q4)*sin(q5) - KUKA_LBR_param_.dblLink7CogY*sin(q4)*sin(q5)*sin(q7) + cos(q5)*cos(q6)*sin(q4)*(KUKA_LBR_param_.dblLink7CogY*cos(q7) + KUKA_LBR_param_.dblLink7CogX*sin(q7)) - cos(q4)*sin(q6)*(KUKA_LBR_param_.dblLink7CogY*cos(q7) + KUKA_LBR_param_.dblLink7CogX*sin(q7))) + cos(q2)*(sin(q3)*(-(cos(q6)*sin(q5)*(KUKA_LBR_param_.dblLink7CogY*cos(q7) + KUKA_LBR_param_.dblLink7CogX*sin(q7))) + cos(q5)*(KUKA_LBR_param_.dblLink7CogX*cos(q7) - KUKA_LBR_param_.dblLink7CogY*sin(q7))) + cos(q3)*(sin(q4)*sin(q6)*(KUKA_LBR_param_.dblLink7CogY*cos(q7) + KUKA_LBR_param_.dblLink7CogX*sin(q7)) + cos(q4)*(cos(q5)*cos(q6)*(KUKA_LBR_param_.dblLink7CogY*cos(q7) + KUKA_LBR_param_.dblLink7CogX*sin(q7)) + sin(q5)*(KUKA_LBR_param_.dblLink7CogX*cos(q7) - KUKA_LBR_param_.dblLink7CogY*sin(q7)))))))*(sin(q1)*(cos(q3)*(cos(q5)*(KUKA_LBR_param_.dblLink7CogY*cos(q7) + KUKA_LBR_param_.dblLink7CogX*sin(q7)) + sin(q5)*(KUKA_LBR_param_.dblLink7CogX*cos(q6)*cos(q7) - KUKA_LBR_param_.dblLink7CogZ*sin(q6) - KUKA_LBR_param_.dblLink7CogY*cos(q6)*sin(q7))) + sin(q3)*(sin(q4)*(KUKA_LBR_param_.dblLink45Len + KUKA_LBR_param_.dblLink7CogZ*cos(q6) + KUKA_LBR_param_.dblLink7CogX*cos(q7)*sin(q6) - KUKA_LBR_param_.dblLink7CogY*sin(q6)*sin(q7)) - cos(q4)*(sin(q5)*(KUKA_LBR_param_.dblLink7CogY*cos(q7) + KUKA_LBR_param_.dblLink7CogX*sin(q7)) + cos(q5)*(-(KUKA_LBR_param_.dblLink7CogX*cos(q6)*cos(q7)) + KUKA_LBR_param_.dblLink7CogZ*sin(q6) + KUKA_LBR_param_.dblLink7CogY*cos(q6)*sin(q7))))) + cos(q1)*(sin(q2)*(KUKA_LBR_param_.dblLink23Len + KUKA_LBR_param_.dblLink7CogY*cos(q7)*sin(q4)*sin(q5) + KUKA_LBR_param_.dblLink7CogX*sin(q4)*sin(q5)*sin(q7) + cos(q5)*sin(q4)*(-(KUKA_LBR_param_.dblLink7CogX*cos(q6)*cos(q7)) + KUKA_LBR_param_.dblLink7CogZ*sin(q6) + KUKA_LBR_param_.dblLink7CogY*cos(q6)*sin(q7)) + cos(q4)*(KUKA_LBR_param_.dblLink45Len + KUKA_LBR_param_.dblLink7CogZ*cos(q6) + KUKA_LBR_param_.dblLink7CogX*cos(q7)*sin(q6) - KUKA_LBR_param_.dblLink7CogY*sin(q6)*sin(q7))) + cos(q2)*(sin(q3)*(cos(q5)*(KUKA_LBR_param_.dblLink7CogY*cos(q7) + KUKA_LBR_param_.dblLink7CogX*sin(q7)) + sin(q5)*(KUKA_LBR_param_.dblLink7CogX*cos(q6)*cos(q7) - KUKA_LBR_param_.dblLink7CogZ*sin(q6) - KUKA_LBR_param_.dblLink7CogY*cos(q6)*sin(q7))) + cos(q3)*(-(sin(q4)*(KUKA_LBR_param_.dblLink45Len + KUKA_LBR_param_.dblLink7CogZ*cos(q6) + KUKA_LBR_param_.dblLink7CogX*cos(q7)*sin(q6) - KUKA_LBR_param_.dblLink7CogY*sin(q6)*sin(q7))) + cos(q4)*(sin(q5)*(KUKA_LBR_param_.dblLink7CogY*cos(q7) + KUKA_LBR_param_.dblLink7CogX*sin(q7)) + cos(q5)*(-(KUKA_LBR_param_.dblLink7CogX*cos(q6)*cos(q7)) + KUKA_LBR_param_.dblLink7CogZ*sin(q6) + KUKA_LBR_param_.dblLink7CogY*cos(q6)*sin(q7))))))));
